simulink model "simulator_prototype_v2"  (R2021b)
(part 7 of 12)

t4573 = t3468.*t4113;
t4590 = t4080.*(t1896-t3232).*(-1.0e-8);
t4591 = (t4080.*(t1896-t3232))./1.0e+8;
t4603 = t4080.*(t1896-t3232).*(-6.2e-7);
t4604 = t4080.*(t1896-t3232).*6.2e-7;
t4610 = t4149.*(t1896-t3232).*(-7.26735e-3);
t4611 = t4149.*(t1896-t3232).*7.26735e-3;
t4648 = t528+t983+t1015+t1068+t1494+t1529+t2523+t2789+t2809+t3020+t3021;
t4649 = t2292+t3283+t3583+t3590;
t4653 = t1018+t1020+t1049+t1505+t2760+t2789+t2809+t2822+t3020+t3021;
t4654 = t562+t996+t1046+t1093+t1516+t1543+t2636+t2902+t2921+t3040+t3041;
t4662 = t1050+t1051+t1067+t1527+t2852+t2902+t2921+t2936+t3040+t3041;
t4675 = -t4302.*(t1861-t3214);
t4678 = t4302.*(t1861-t3214);
t4716 = t2757+t3403+t3704+t3707;
t4764 = t4323.*(t1896-t3232).*(-7.26735e-3);
t4777 = t3887+t4095;
t4780 = t3889+t4102;
t4785 = -t4365.*(t1861-t3214);
t4787 = t4365.*(t1861-t3214);
t4790 = t4080.*(t2694-t2701+t3036-t3043).*(-1.0e-8);
t4811 = t4783.*1.838876e-2;
t4813 = t4784.*9.99471e-3;
t4814 = t3909+t4126;
t4827 = t3915+t4137;
t4830 = t4080.*(t2694-t2701+t3036-t3043).*(-3.24e-6);
t4831 = t4080.*(t2694-t2701+t3036-t3043).*(-7.83e-6);
t4832 = t4080.*(t2694-t2701+t3036-t3043).*(-6.2e-7);
t4840 = t28.*t4817;
t4841 = t34.*t4817;
t4872 = t4399.*(t1896-t3232).*(-7.26735e-3);
t4873 = t4399.*(t1896-t3232).*7.26735e-3;
t4977 = t4211+t4218;
t4994 = t3209.*t4707;
t4995 = t3210.*t4707;
t5013 = t3229.*t4776.*7.26735e-3;
t5014 = t3230.*t4776.*7.26735e-3;
t5030 = -t5029;
t5058 = t3481.*t4758;
t5144 = t3524.*t4795.*7.26735e-3;
t5145 = t4795.*(t1896-t3232).*(-7.26735e-3);
t5159 = t3481.*t4865.*9.840000000000001e-6;
t5189 = t3789.*t4817;
t5197 = t50.*t189.*t5191.*9.543032792050485e-17;
t5199 = t3882.*t4707;
t5200 = -t4707.*(-t1901+t3122+t3270);
t5202 = t4707.*(-t1901+t3122+t3270);
t5207 = -t3863.*(t4127+t33.*(t1959-t3306+t38.*t1022.*(t855-t878).*2.196325630278387e-1));
t5225 = t3904.*t4776.*7.26735e-3;
t5226 = t4776.*(t1959-t3306+t38.*t1022.*(t855-t878).*2.196325630278387e-1).*(-7.26735e-3);
t5236 = -t5231;
t5244 = -t5241;
t5255 = t4080.*t4758;
t5265 = t4099+t4784;
t5266 = t4104+t4783;
t5301 = t4113.*t4795.*7.26735e-3;
t5302 = t4795.*(t1005+t26.*(t1941-t3308+t39.*t1022.*(t855-t878).*2.196325630278387e-1)).*(-7.26735e-3);
t5361 = t4312.*t4822;
et67 = -t2306-t2317+t3144+t3147+t35.*t941.*t948.*(t850-t874).*3.775747223193135e-1;
et68 = t36.*t941.*t948.*(t850-t874).*2.244797987218524e-1;
t5362 = (et67+et68).*(-t3519+t3521+t50.*t188.*t202.*(t46-t47).*2.711709361697228e-39);
t5433 = t3732.*t3877.*t3901.*t4134.*1.08769e-2;
t5434 = t3732.*t4134.*(t2674-t2676+t3022-t3027).*(t2694-t2701+t3036-t3043).*1.08769e-2;
t5440 = t3689.*t3877.*t3901.*t4175.*1.08769e-2;
t5441 = t3689.*t4175.*(t2674-t2676+t3022-t3027).*(t2694-t2701+t3036-t3043).*1.08769e-2;
t5480 = t3784.*t3877.*t3901.*t4134.*1.08769e-2;
t5481 = t3784.*t4134.*(t2674-t2676+t3022-t3027).*(t2694-t2701+t3036-t3043).*1.08769e-2;
t5483 = t3782.*t3877.*t3901.*t4175.*1.08769e-2;
t5484 = t3782.*t4175.*(t2674-t2676+t3022-t3027).*(t2694-t2701+t3036-t3043).*1.08769e-2;
t5489 = t3733+t4448+t4467;
t5668 = t3877.*t3901.*t3918.*(t1488+t1874+t2519+t2740+t2747+t3096+t3097).*(-7.26735e-3);
t5669 = t3918.*(t2674-t2676+t3022-t3027).*(t2694-t2701+t3036-t3043).*(t1488+t1874+t2519+t2740+t2747+t3096+t3097).*(-7.26735e-3);
t5670 = t3877.*t3901.*t3918.*(t1488+t1874+t2519+t2740+t2747+t3096+t3097).*7.26735e-3;
t5671 = t3918.*(t2674-t2676+t3022-t3027).*(t2694-t2701+t3036-t3043).*(t1488+t1874+t2519+t2740+t2747+t3096+t3097).*7.26735e-3;
t5672 = t3877.*t3892.*t3901.*(t1513+t1879+t2598+t2820+t2834+t3117+t3118).*(-7.26735e-3);
t5673 = t3892.*(t2674-t2676+t3022-t3027).*(t2694-t2701+t3036-t3043).*(t1513+t1879+t2598+t2820+t2834+t3117+t3118).*(-7.26735e-3);
t5674 = t3877.*t3892.*t3901.*(t1513+t1879+t2598+t2820+t2834+t3117+t3118).*7.26735e-3;
t5675 = t3892.*(t2674-t2676+t3022-t3027).*(t2694-t2701+t3036-t3043).*(t1513+t1879+t2598+t2820+t2834+t3117+t3118).*7.26735e-3;
t5678 = t3877.*t3901.*t3984.*(t1488+t1874+t2519+t2740+t2747+t3096+t3097).*(-7.26735e-3);
t5679 = t3984.*(t2674-t2676+t3022-t3027).*(t2694-t2701+t3036-t3043).*(t1488+t1874+t2519+t2740+t2747+t3096+t3097).*(-7.26735e-3);
tau_c = ft_9({t1005,t1022,t1089,t1104,t1105,t1108,t1115,t1121,t1158,t1159,t1190,t1193,t1194,t1196,t1205,t1207,t1208,t1210,t1212,t1214,t1217,t1218,t1219,t1220,t1221,t1222,t123,t1230,t1235,t1236,t1237,t1238,t1288,t1289,t1302,t1303,t1319,t1320,t1336,t1348,t1350,t1351,t1360,t1369,t1378,t1396,t14,t140,t1425,t1435,t1456,t1477,t1488,t15,t1513,t1539,t1544,t1545,t1547,t1548,t1549,t1553,t1554,t1559,t1564,t1565,t1576,t1577,t1578,t1579,t1581,t1584,t1585,t1586,t1587,t1591,t1595,t1596,t1598,t1599,t16,t1600,t1601,t1602,t1604,t1605,t1606,t1607,t1608,t1609,t1612,t1613,t1614,t1615,t1616,t1626,t1627,t1628,t1629,t1631,t1637,t1640,t1641,t1648,t1649,t1659,t1660,t1661,t1666,t1667,t1683,t1686,t1690,t1692,t17,t1700,t1701,t1703,t1704,t1705,t1712,t1717,t1738,t1741,t1742,t1750,t1752,t1753,t1754,t1758,t1759,t1775,t1776,t18,t1861,t1874,t1879,t188,t1881,t189,t1896,t19,t1901,t1941,t1953,t1959,t1973,t1993,t1994,t2,t20,t201,t202,t2023,t2053,t2060,t2089,t2090,t2098,t2099,t21,t2117,t2120,t2122,t2123,t2125,t2130,t2137,t2138,t2139,t2140,t2141,t2142,t2145,t2146,t2147,t2149,t2150,t2151,t2152,t2153,t2154,t2155,t2156,t2157,t2159,t2160,t2162,t2164,t2165,t2166,t2167,t2168,t2169,t2174,t2183,t2187,t2193,t2194,t2195,t2199,t22,t2203,t2215,t2219,t2222,t2223,t2239,t2240,t2256,t2257,t2291,t2292,t2293,t2294,t2295,t2296,t2297,t2298,t2299,t23,t2300,t2301,t2302,t2303,t2304,t2306,t2307,t2308,t2309,t2310,t2311,t2313,t2317,t2320,t2322,t2323,t2324,t2325,t2326,t2327,t2328,t2329,t2337,t2338,t2339,t2341,t2342,t2343,t2344,t2352,t2353,t2354,t2355,t2357,t2358,t2359,t236,t2360,t2361,t2362,t2363,t2364,t2365,t2366,t2367,t2368,t2369,t237,t2370,t2371,t2374,t2375,t2378,t2379,t238,t2380,t2384,t2388,t2389,t2391,t2394,t2395,t2397,t2398,t2399,t24,t2400,t2401,t2402,t2403,t2404,t2405,t241,t2413,t2414,t2419,t2421,t2422,t2423,t2433,t2434,t2438,t244,t2447,t2448,t2449,t2450,t2459,t2460,t2461,t2471,t2472,t2492,t2493,t2494,t25,t2502,t2508,t2509,t2510,t2515,t2519,t2520,t2525,t2527,t2529,t2530,t2532,t2534,t2539,t2555,t2556,t2572,t2575,t2583,t2598,t26,t2605,t2606,t2612,t2613,t2615,t2618,t2619,t262,t2638,t264,t2651,t2652,t2664,t2670,t2671,t2673,t2674,t2675,t2676,t2678,t2680,t2681,t2682,t2683,t2684,t2685,t2686,t2687,t2689,t2690,t2692,t2693,t2694,t2695,t2696,t2697,t2698,t27,t2700,t2701,t2704,t2705,t2707,t2708,t2709,t2711,t2712,t2713,t2715,t2716,t2717,t2719,t2720,t2721,t2733,t2735,t2736,t2740,t2742,t2744,t2745,t2747,t2748,t2749,t2750,t2753,t2754,t2759,t2765,t2769,t2773,t2774,t2775,t2777,t2778,t2779,t2781,t2785,t2786,t2787,t2788,t2790,t2792,t2795,t2797,t2798,t2799,t28,t2801,t2802,t2803,t2804,t2805,t2807,t2808,t2813,t2814,t2820,t2823,t2828,t2831,t2834,t2835,t2838,t2850,t2851,t2927,t2937,t2941,t2942,t2945,t2946,t2947,t2948,t2950,t2951,t2953,t2954,t2955,t2956,t2957,t2962,t2963,t2964,t2965,t2966,t2969,t2970,t2971,t2972,t2973,t2975,t2976,t2977,t2978,t2979,t2982,t2984,t2985,t2986,t2987,t2990,t2991,t2993,t2994,t2998,t3,t30,t3003,t3004,t3006,t3008,t3009,t3010,t3015,t3016,t3017,t3018,t3019,t3022,t3027,t3029,t3030,t3031,t3036,t3043,t3044,t3045,t3047,t3049,t3050,t3051,t3054,t3055,t3056,t3057,t3063,t3064,t3065,t3066,t3067,t3068,t3069,t3072,t3073,t3074,t3075,t3076,t3077,t3078,t3079,t3080,t3081,t3082,t3083,t3085,t3086,t3087,t3088,t3096,t3097,t31,t3109,t3117,t3118,t3119,t3121,t3122,t3128,t3129,t313,t3130,t3131,t3132,t3133,t3134,t3135,t3139,t314,t3140,t3141,t3142,t3144,t3147,t3149,t3150,t3152,t3153,t3154,t3155,t3156,t3157,t3158,t3159,t3160,t3161,t3162,t3163,t3164,t3165,t3166,t3170,t3171,t3172,t3178,t3179,t3180,t3184,t3186,t3187,t3188,t3189,t3190,t3191,t3193,t3194,t3196,t3197,t3198,t3199,t32,t3200,t3201,t3204,t3205,t3206,t3209,t321,t3210,t3212,t3214,t3215,t3217,t3218,t322,t3220,t3222,t3223,t3224,t3225,t3226,t3227,t3228,t3229,t3230,t3231,t3232,t3233,t3235,t3238,t3240,t3241,t3242,t3244,t3245,t3246,t3247,t3248,t3249,t3250,t3252,t3253,t3254,t3256,t3258,t3259,t326,t3260,t3261,t3262,t3263,t3264,t3265,t3266,t3269,t3270,t3271,t3272,t3275,t3276,t3277,t3278,t328,t3280,t3281,t3282,t3283,t3284,t3285,t3287,t3288,t3289,t329,t3290,t3291,t3293,t3294,t3296,t3297,t33,t330,t3300,t3301,t3302,t3303,t3304,t3305,t3306,t3308,t331,t3313,t3316,t3318,t3319,t332,t3321,t3322,t3323,t3324,t3325,t3326,t3327,t3328,t3329,t333,t3330,t3331,t3332,t3333,t3334,t3335,t3336,t3338,t3339,t3341,t3342,t3343,t3344,t3346,t3347,t3348,t3349,t335,t3350,t3351,t3352,t3353,t3354,t3355,t3356,t3359,t3360,t3367,t3369,t3370,t3373,t3376,t3377,t3379,t338,t3382,t3383,t3384,t3385,t3386,t3387,t3388,t3389,t339,t3392,t3394,t3395,t3396,t3397,t3398,t3399,t34,t3400,t3401,t3407,t3408,t3409,t341,t3410,t3411,t3412,t3415,t3417,t3419,t3420,t3421,t3422,t3423,t3424,t3427,t3428,t3429,t343,t3430,t3432,t3433,t3434,t3435,t3436,t3437,t3438,t3440,t3441,t3442,t3443,t3444,t3445,t3446,t3447,t3449,t3450,t3451,t3452,t3453,t3455,t3456,t3457,t3458,t3459,t346,t3461,t3464,t3465,t3467,t3468,t3470,t3473,t3475,t3477,t3479,t3480,t3481,t3483,t3484,t3485,t3486,t3487,t3488,t3489,t3490,t3495,t3498,t35,t350,t3505,t351,t3511,t3519,t352,t3522,t3523,t3524,t3526,t3527,t3528,t3529,t3531,t3533,t3534,t3535,t3536,t3537,t3538,t354,t3541,t3547,t3552,t3558,t3559,t356,t3560,t3561,t3563,t3566,t3576,t3577,t3578,t3579,t358,t3581,t3584,t3588,t359,t3590,t3595,t3598,t36,t360,t3607,t3617,t362,t3622,t3623,t3624,t3625,t3627,t3628,t363,t3630,t3634,t364,t3645,t3647,t365,t3655,t3659,t366,t3662,t3665,t3667,t3669,t3670,t3672,t3673,t3674,t3676,t3677,t3678,t3679,t3680,t3681,t3682,t3683,t3684,t3685,t3686,t3687,t3688,t3689,t369,t3690,t3699,t370,t3700,t3703,t3705,t371,t3711,t372,t3725,t3732,t3734,t3735,t3736,t3737,t3738,t3739,t3740,t3741,t3743,t3745,t3746,t3748,t3749,t3751,t3753,t3755,t3756,t3757,t3758,t3759,t3760,t3762,t3763,t3764,t3765,t3766,t3767,t3768,t3769,t3770,t3771,t3772,t3774,t3775,t3776,t3778,t3779,t378,t3782,t3783,t3784,t3785,t3786,t3787,t3788,t3789,t3790,t3791,t3792,t3793,t3794,t3795,t3796,t3798,t3799,t38,t380,t3800,t3802,t3804,t3805,t3807,t3811,t3812,t3813,t3814,t3815,t3816,t3817,t3818,t3819,t382,t3821,t3822,t3823,t3826,t3827,t3828,t3832,t3833,t3834,t3836,t3842,t3843,t3844,t3845,t3847,t3849,t3850,t3852,t3853,t3854,t3855,t3856,t3858,t3859,t3862,t3863,t3864,t3865,t3866,t3867,t3869,t387,t3870,t3871,t3872,t3873,t3876,t3877,t3880,t3882,t3886,t3891,t3892,t3893,t3894,t3895,t3898,t39,t3900,t3901,t3904,t3908,t3910,t3913,t3916,t3917,t3918,t3919,t3920,t3921,t3925,t3926,t3927,t3928,t3929,t3932,t3933,t3934,t3935,t3936,t3937,t3938,t3939,t3940,t3941,t3943,t3945,t3949,t3953,t3954,t3955,t3956,t3958,t3960,t3962,t3964,t3965,t3966,t3970,t3971,t3974,t3975,t3976,t3978,t3984,t3987,t3993,t3994,t3995,t3997,t3998,t4,t4000,t4001,t4002,t4003,t4004,t4005,t4009,t4012,t4019,t4020,t4023,t4028,t4029,t4030,t4033,t4045,t4046,t4048,t4049,t4054,t4058,t4060,t4063,t4080,t4087,t4088,t410,t4106,t4107,t4108,t4109,t4111,t4113,t4122,t4125,t4127,t4129,t4131,t4133,t4134,t4138,t4139,t4143,t4144,t4149,t4154,t4157,t4158,t4160,t4162,t4163,t4164,t4165,t4166,t4170,t4171,t4172,t4173,t4174,t4175,t4176,t4177,t4182,t4183,t4185,t4186,t4187,t4188,t4191,t4195,t4196,t4197,t4198,t42,t4204,t4205,t4206,t4207,t4212,t4214,t4215,t4219,t4220,t4221,t4225,t4228,t4230,t4231,t4233,t4234,t4235,t4236,t4241,t4242,t4244,t4249,t4250,t4251,t4253,t4254,t4257,t4259,t4262,t4263,t4272,t4273,t4277,t4279,t4280,t4281,t4283,t4285,t4286,t4288,t429,t4290,t4292,t4295,t4298,t4299,t43,t4300,t4302,t4304,t4308,t4310,t4317,t4318,t4321,t4322,t4323,t4324,t4327,t4328,t4329,t4330,t4333,t4334,t4336,t4337,t4338,t4339,t4340,t4342,t4344,t4346,t4347,t4348,t4349,t4350,t4351,t4352,t4355,t4356,t4360,t4362,t4363,t4364,t4365,t4366,t4367,t4368,t4371,t4399,t4401,t4404,t4405,t4407,t4408,t4412,t4413,t4415,t4416,t4417,t4418,t4419,t4420,t4421,t4425,t4426,t4427,t4428,t4429,t4430,t4431,t4432,t4434,t4435,t4436,t4437,t4439,t4441,t4444,t4446,t4447,t4449,t4450,t4451,t4453,t4454,t4455,t4456,t4458,t4460,t4462,t4463,t4468,t4471,t4473,t4474,t4476,t4479,t4480,t4483,t4484,t4489,t4496,t4500,t4573,t4574,t4579,t4587,t4589,t4591,t4594,t4599,t46,t4602,t4604,t4607,t4610,t4611,t4614,t4615,t4617,t4620,t4640,t4641,t4642,t4644,t4645,t4647,t4648,t4649,t4650,t4652,t4653,t4654,t4655,t4661,t4662,t4663,t4664,t4667,t4669,t4678,t4679,t4680,t4682,t4683,t4686,t4687,t4688,t4689,t4690,t4691,t4692,t4693,t4694,t4695,t4696,t4697,t4698,t4699,t47,t4700,t4701,t4702,t4703,t4704,t4705,t4716,t4742,t4758,t4764,t4772,t4777,t4779,t4780,t4785,t4787,t4789,t4790,t4791,t4792,t4795,t4811,t4813,t4814,t4816,t4817,t4820,t4821,t4822,t4823,t4826,t4829,t4830,t4831,t4832,t4837,t4838,t4839,t4840,t4841,t4842,t4860,t4865,t4868,t4869,t4870,t4871,t4872,t4873,t4898,t4911,t4931,t4963,t4964,t4965,t4966,t4974,t4976,t4977,t4985,t4986,t4994,t4995,t5,t50,t5001,t5002,t5005,t5007,t5010,t5013,t5014,t5017,t5021,t5023,t5026,t5030,t5035,t5036,t5037,t5038,t5039,t5040,t5041,t5042,t5043,t5044,t5045,t5046,t5047,t5048,t5049,t5050,t5058,t5061,t5144,t5145,t5153,t5159,t5167,t5168,t5169,t5189,t5191,t5197,t5199,t5202,t5207,t5219,t5221,t5223,t5224,t5225,t5226,t5227,t5229,t5230,t5231,t5233,t5235,t5236,t5239,t5240,t5241,t5243,t5244,t5245,t5246,t5247,t5248,t5252,t5254,t5255,t5257,t5265,t5266,t5301,t5302,t5306,t5308,t5316,t5317,t5320,t5328,t5337,t5338,t5339,t5340,t5342,t5344,t5345,t5346,t5347,t5348,t5349,t5350,t5361,t5362,t5377,t5379,t5380,t5381,t5383,t5384,t5388,t5389,t5399,t5402,t5403,t5405,t5407,t5411,t5427,t5428,t5433,t5434,t5440,t5441,t5443,t5444,t5480,t5481,t5482,t5483,t5484,t5485,t5486,t5487,t5488,t5489,t5490,t5491,t5492,t5493,t5494,t5496,t5498,t5500,t5510,t5517,t5518,t5524,t5531,t5552,t5578,t5580,t56,t5620,t5626,t5627,t5631,t5670,t5671,t5674,t5675,t5678,t5679,t5694,t5695,t5702,t5703,t5719,t5722,t5723,t58,t5835,t5839,t5840,t59,t5932,t5951,t5953,t5954,t6,t60,t6183,t6184,t6185,t6219,t6221,t6247,t6253,t628,t635,t636,t638,t640,t641,t642,t643,t645,t646,t6484,t6485,t6486,t649,t654,t6543,t6544,t655,t656,t657,t659,t660,t663,t664,t665,t6658,t666,t6663,t667,t668,t669,t67,t670,t672,t673,t674,t675,t676,t677,t678,t679,t68,t681,t6811,t6812,t6813,t682,t683,t684,t685,t686,t687,t689,t6892,t6893,t691,t692,t693,t694,t7,t70,t702,t7041,t707,t708,t71,t710,t715,t716,t717,t718,t721,t722,t724,t725,t73,t736,t738,t740,t741,t749,t756,t76,t762,t768,t777,t792,t793,t801,t802,t808,t813,t819,t821,t850,t855,t874,t878,t89,t90,t91,t92,t941,t944,t948,t951,t97});
end
function tau_c = ft_9(ct)
t1005 = ct{1};
t1022 = ct{2};
t1089 = ct{3};
t1104 = ct{4};
t1105 = ct{5};
t1108 = ct{6};
t1115 = ct{7};
t1121 = ct{8};
t1158 = ct{9};
t1159 = ct{10};
t1190 = ct{11};
t1193 = ct{12};
t1194 = ct{13};
t1196 = ct{14};
t1205 = ct{15};
t1207 = ct{16};
t1208 = ct{17};
t1210 = ct{18};
t1212 = ct{19};
t1214 = ct{20};
t1217 = ct{21};
t1218 = ct{22};
t1219 = ct{23};
t1220 = ct{24};
t1221 = ct{25};
t1222 = ct{26};
t123 = ct{27};
t1230 = ct{28};
t1235 = ct{29};
t1236 = ct{30};
t1237 = ct{31};
t1238 = ct{32};
t1288 = ct{33};
t1289 = ct{34};
t1302 = ct{35};
t1303 = ct{36};
t1319 = ct{37};
t1320 = ct{38};
t1336 = ct{39};
t1348 = ct{40};
t1350 = ct{41};
t1351 = ct{42};
t1360 = ct{43};
t1369 = ct{44};
t1378 = ct{45};
t1396 = ct{46};
t14 = ct{47};
t140 = ct{48};
t1425 = ct{49};
t1435 = ct{50};
t1456 = ct{51};
t1477 = ct{52};
t1488 = ct{53};
t15 = ct{54};
t1513 = ct{55};
t1539 = ct{56};
t1544 = ct{57};
t1545 = ct{58};
t1547 = ct{59};
t1548 = ct{60};
t1549 = ct{61};
t1553 = ct{62};
t1554 = ct{63};
t1559 = ct{64};
t1564 = ct{65};
t1565 = ct{66};
t1576 = ct{67};
t1577 = ct{68};
t1578 = ct{69};
t1579 = ct{70};
t1581 = ct{71};
t1584 = ct{72};
t1585 = ct{73};
t1586 = ct{74};
t1587 = ct{75};
t1591 = ct{76};
t1595 = ct{77};
t1596 = ct{78};
t1598 = ct{79};
t1599 = ct{80};
t16 = ct{81};
t1600 = ct{82};
t1601 = ct{83};
t1602 = ct{84};
t1604 = ct{85};
t1605 = ct{86};
t1606 = ct{87};
t1607 = ct{88};
t1608 = ct{89};
t1609 = ct{90};
t1612 = ct{91};
t1613 = ct{92};
t1614 = ct{93};
t1615 = ct{94};
t1616 = ct{95};
t1626 = ct{96};
t1627 = ct{97};
t1628 = ct{98};
t1629 = ct{99};
t1631 = ct{100};
t1637 = ct{101};
t1640 = ct{102};
t1641 = ct{103};
t1648 = ct{104};
t1649 = ct{105};
t1659 = ct{106};
t1660 = ct{107};
t1661 = ct{108};
t1666 = ct{109};
t1667 = ct{110};
t1683 = ct{111};
t1686 = ct{112};
t1690 = ct{113};
t1692 = ct{114};
t17 = ct{115};
t1700 = ct{116};
t1701 = ct{117};
t1703 = ct{118};
t1704 = ct{119};
t1705 = ct{120};
t1712 = ct{121};
t1717 = ct{122};
t1738 = ct{123};
t1741 = ct{124};
t1742 = ct{125};
t1750 = ct{126};
t1752 = ct{127};
t1753 = ct{128};
t1754 = ct{129};
t1758 = ct{130};
t1759 = ct{131};
t1775 = ct{132};
t1776 = ct{133};
t18 = ct{134};
t1861 = ct{135};
t1874 = ct{136};
t1879 = ct{137};
t188 = ct{138};
t1881 = ct{139};
t189 = ct{140};
t1896 = ct{141};
t19 = ct{142};
t1901 = ct{143};
t1941 = ct{144};
t1953 = ct{145};
t1959 = ct{146};
t1973 = ct{147};
t1993 = ct{148};
t1994 = ct{149};
t2 = ct{150};
t20 = ct{151};
t201 = ct{152};
t202 = ct{153};
t2023 = ct{154};
t2053 = ct{155};
t2060 = ct{156};
t2089 = ct{157};
t2090 = ct{158};
t2098 = ct{159};
t2099 = ct{160};
t21 = ct{161};
t2117 = ct{162};
t2120 = ct{163};
t2122 = ct{164};
t2123 = ct{165};
t2125 = ct{166};
t2130 = ct{167};
t2137 = ct{168};
t2138 = ct{169};
t2139 = ct{170};
t2140 = ct{171};
t2141 = ct{172};
t2142 = ct{173};
t2145 = ct{174};
t2146 = ct{175};
t2147 = ct{176};
t2149 = ct{177};
t2150 = ct{178};
t2151 = ct{179};
t2152 = ct{180};
t2153 = ct{181};
t2154 = ct{182};
t2155 = ct{183};
t2156 = ct{184};
t2157 = ct{185};
t2159 = ct{186};
t2160 = ct{187};
t2162 = ct{188};
t2164 = ct{189};
t2165 = ct{190};
t2166 = ct{191};
t2167 = ct{192};
t2168 = ct{193};
t2169 = ct{194};
t2174 = ct{195};
t2183 = ct{196};
t2187 = ct{197};
t2193 = ct{198};
t2194 = ct{199};
t2195 = ct{200};
t2199 = ct{201};
t22 = ct{202};
t2203 = ct{203};
t2215 = ct{204};
t2219 = ct{205};
t2222 = ct{206};
t2223 = ct{207};
t2239 = ct{208};
t2240 = ct{209};
t2256 = ct{210};
t2257 = ct{211};
t2291 = ct{212};
t2292 = ct{213};
t2293 = ct{214};
t2294 = ct{215};
t2295 = ct{216};
t2296 = ct{217};
t2297 = ct{218};
t2298 = ct{219};
t2299 = ct{220};
t23 = ct{221};
t2300 = ct{222};
t2301 = ct{223};
t2302 = ct{224};
t2303 = ct{225};
t2304 = ct{226};
t2306 = ct{227};
t2307 = ct{228};
t2308 = ct{229};
t2309 = ct{230};
t2310 = ct{231};
t2311 = ct{232};
t2313 = ct{233};
t2317 = ct{234};
t2320 = ct{235};
t2322 = ct{236};
t2323 = ct{237};
t2324 = ct{238};
t2325 = ct{239};
t2326 = ct{240};
t2327 = ct{241};
t2328 = ct{242};
t2329 = ct{243};
t2337 = ct{244};
t2338 = ct{245};
t2339 = ct{246};
t2341 = ct{247};
t2342 = ct{248};
t2343 = ct{249};
t2344 = ct{250};
t2352 = ct{251};
t2353 = ct{252};
t2354 = ct{253};
t2355 = ct{254};
t2357 = ct{255};
t2358 = ct{256};
t2359 = ct{257};
t236 = ct{258};
t2360 = ct{259};
t2361 = ct{260};
t2362 = ct{261};
t2363 = ct{262};
t2364 = ct{263};
t2365 = ct{264};
t2366 = ct{265};
t2367 = ct{266};
t2368 = ct{267};
t2369 = ct{268};
t237 = ct{269};
t2370 = ct{270};
t2371 = ct{271};
t2374 = ct{272};
t2375 = ct{273};
t2378 = ct{274};
t2379 = ct{275};
t238 = ct{276};
t2380 = ct{277};
t2384 = ct{278};
t2388 = ct{279};
t2389 = ct{280};
t2391 = ct{281};
t2394 = ct{282};
t2395 = ct{283};
t2397 = ct{284};
t2398 = ct{285};
t2399 = ct{286};
t24 = ct{287};
t2400 = ct{288};
t2401 = ct{289};
t2402 = ct{290};
t2403 = ct{291};
t2404 = ct{292};
t2405 = ct{293};
t241 = ct{294};
t2413 = ct{295};
t2414 = ct{296};
t2419 = ct{297};
t2421 = ct{298};
t2422 = ct{299};
t2423 = ct{300};
t2433 = ct{301};
t2434 = ct{302};
t2438 = ct{303};
t244 = ct{304};
t2447 = ct{305};
t2448 = ct{306};
t2449 = ct{307};
t2450 = ct{308};
t2459 = ct{309};
t2460 = ct{310};
t2461 = ct{311};
t2471 = ct{312};
t2472 = ct{313};
t2492 = ct{314};
t2493 = ct{315};
t2494 = ct{316};
t25 = ct{317};
t2502 = ct{318};
t2508 = ct{319};
t2509 = ct{320};
t2510 = ct{321};
t2515 = ct{322};
t2519 = ct{323};
t2520 = ct{324};
t2525 = ct{325};
t2527 = ct{326};
t2529 = ct{327};
t2530 = ct{328};
t2532 = ct{329};
t2534 = ct{330};
t2539 = ct{331};
t2555 = ct{332};
t2556 = ct{333};
t2572 = ct{334};
t2575 = ct{335};
t2583 = ct{336};
t2598 = ct{337};
t26 = ct{338};
t2605 = ct{339};
t2606 = ct{340};
t2612 = ct{341};
t2613 = ct{342};
t2615 = ct{343};
t2618 = ct{344};
t2619 = ct{345};
t262 = ct{346};
t2638 = ct{347};
t264 = ct{348};
t2651 = ct{349};
t2652 = ct{350};
t2664 = ct{351};
t2670 = ct{352};
t2671 = ct{353};
t2673 = ct{354};
t2674 = ct{355};
t2675 = ct{356};
t2676 = ct{357};
t2678 = ct{358};
t2680 = ct{359};
t2681 = ct{360};
t2682 = ct{361};
t2683 = ct{362};
t2684 = ct{363};
t2685 = ct{364};
t2686 = ct{365};
t2687 = ct{366};
t2689 = ct{367};
t2690 = ct{368};
t2692 = ct{369};
t2693 = ct{370};
t2694 = ct{371};
t2695 = ct{372};
t2696 = ct{373};
t2697 = ct{374};
t2698 = ct{375};
t27 = ct{376};
t2700 = ct{377};
t2701 = ct{378};
t2704 = ct{379};
t2705 = ct{380};
t2707 = ct{381};
t2708 = ct{382};
t2709 = ct{383};
t2711 = ct{384};
t2712 = ct{385};
t2713 = ct{386};
t2715 = ct{387};
t2716 = ct{388};
t2717 = ct{389};
t2719 = ct{390};
t2720 = ct{391};
t2721 = ct{392};
t2733 = ct{393};
t2735 = ct{394};
t2736 = ct{395};
t2740 = ct{396};
t2742 = ct{397};
t2744 = ct{398};
t2745 = ct{399};
t2747 = ct{400};
t2748 = ct{401};
t2749 = ct{402};
t2750 = ct{403};
t2753 = ct{404};
t2754 = ct{405};
t2759 = ct{406};
t2765 = ct{407};
t2769 = ct{408};
t2773 = ct{409};
t2774 = ct{410};
t2775 = ct{411};
t2777 = ct{412};
t2778 = ct{413};
t2779 = ct{414};
t2781 = ct{415};
t2785 = ct{416};
t2786 = ct{417};
t2787 = ct{418};
t2788 = ct{419};
t2790 = ct{420};
t2792 = ct{421};
t2795 = ct{422};
t2797 = ct{423};
t2798 = ct{424};
t2799 = ct{425};
t28 = ct{426};
t2801 = ct{427};
t2802 = ct{428};
t2803 = ct{429};
t2804 = ct{430};
t2805 = ct{431};
t2807 = ct{432};
t2808 = ct{433};
t2813 = ct{434};
t2814 = ct{435};
t2820 = ct{436};
t2823 = ct{437};
t2828 = ct{438};
t2831 = ct{439};
t2834 = ct{440};
t2835 = ct{441};
t2838 = ct{442};
t2850 = ct{443};
t2851 = ct{444};
t2927 = ct{445};
t2937 = ct{446};
t2941 = ct{447};
t2942 = ct{448};
t2945 = ct{449};
t2946 = ct{450};
t2947 = ct{451};
t2948 = ct{452};
t2950 = ct{453};
t2951 = ct{454};
t2953 = ct{455};
t2954 = ct{456};
t2955 = ct{457};
t2956 = ct{458};
t2957 = ct{459};
t2962 = ct{460};
t2963 = ct{461};
t2964 = ct{462};
t2965 = ct{463};
t2966 = ct{464};
t2969 = ct{465};
t2970 = ct{466};
t2971 = ct{467};
t2972 = ct{468};
t2973 = ct{469};
t2975 = ct{470};
t2976 = ct{471};
t2977 = ct{472};
t2978 = ct{473};
t2979 = ct{474};
t2982 = ct{475};
t2984 = ct{476};
t2985 = ct{477};
t2986 = ct{478};
t2987 = ct{479};
t2990 = ct{480};
t2991 = ct{481};
t2993 = ct{482};
t2994 = ct{483};
t2998 = ct{484};
t3 = ct{485};
t30 = ct{486};
t3003 = ct{487};
t3004 = ct{488};
t3006 = ct{489};
t3008 = ct{490};
t3009 = ct{491};
t3010 = ct{492};
t3015 = ct{493};
t3016 = ct{494};
t3017 = ct{495};
t3018 = ct{496};
t3019 = ct{497};
t3022 = ct{498};
t3027 = ct{499};
t3029 = ct{500};
t3030 = ct{501};
t3031 = ct{502};
t3036 = ct{503};
t3043 = ct{504};
t3044 = ct{505};
t3045 = ct{506};
t3047 = ct{507};
t3049 = ct{508};
t3050 = ct{509};
t3051 = ct{510};
t3054 = ct{511};
t3055 = ct{512};
t3056 = ct{513};
t3057 = ct{514};
t3063 = ct{515};
t3064 = ct{516};
t3065 = ct{517};
t3066 = ct{518};
t3067 = ct{519};
t3068 = ct{520};
t3069 = ct{521};
t3072 = ct{522};
t3073 = ct{523};
t3074 = ct{524};
t3075 = ct{525};
t3076 = ct{526};
t3077 = ct{527};
t3078 = ct{528};
t3079 = ct{529};
t3080 = ct{530};
t3081 = ct{531};
t3082 = ct{532};
t3083 = ct{533};
t3085 = ct{534};
t3086 = ct{535};
t3087 = ct{536};
t3088 = ct{537};
t3096 = ct{538};
t3097 = ct{539};
t31 = ct{540};
t3109 = ct{541};
t3117 = ct{542};
t3118 = ct{543};
t3119 = ct{544};
t3121 = ct{545};
t3122 = ct{546};
t3128 = ct{547};
t3129 = ct{548};
t313 = ct{549};
t3130 = ct{550};
t3131 = ct{551};
t3132 = ct{552};
t3133 = ct{553};
t3134 = ct{554};
t3135 = ct{555};
t3139 = ct{556};
t314 = ct{557};
t3140 = ct{558};
t3141 = ct{559};
t3142 = ct{560};
t3144 = ct{561};
t3147 = ct{562};
t3149 = ct{563};
t3150 = ct{564};
t3152 = ct{565};
t3153 = ct{566};
t3154 = ct{567};
t3155 = ct{568};
t3156 = ct{569};
t3157 = ct{570};
t3158 = ct{571};
t3159 = ct{572};
t3160 = ct{573};
t3161 = ct{574};
t3162 = ct{575};
t3163 = ct{576};
t3164 = ct{577};
t3165 = ct{578};
t3166 = ct{579};
t3170 = ct{580};
t3171 = ct{581};
t3172 = ct{582};
t3178 = ct{583};
t3179 = ct{584};
t3180 = ct{585};
t3184 = ct{586};
t3186 = ct{587};
t3187 = ct{588};
t3188 = ct{589};
t3189 = ct{590};
t3190 = ct{591};
t3191 = ct{592};
t3193 = ct{593};
t3194 = ct{594};
t3196 = ct{595};
t3197 = ct{596};
t3198 = ct{597};
t3199 = ct{598};
t32 = ct{599};
t3200 = ct{600};
t3201 = ct{601};
t3204 = ct{602};
t3205 = ct{603};
t3206 = ct{604};
t3209 = ct{605};
t321 = ct{606};
t3210 = ct{607};
t3212 = ct{608};
t3214 = ct{609};
t3215 = ct{610};
t3217 = ct{611};
t3218 = ct{612};
t322 = ct{613};
t3220 = ct{614};
t3222 = ct{615};
t3223 = ct{616};
t3224 = ct{617};
t3225 = ct{618};
t3226 = ct{619};
t3227 = ct{620};
t3228 = ct{621};
t3229 = ct{622};
t3230 = ct{623};
t3231 = ct{624};
t3232 = ct{625};
t3233 = ct{626};
t3235 = ct{627};
t3238 = ct{628};
t3240 = ct{629};
t3241 = ct{630};
t3242 = ct{631};
t3244 = ct{632};
t3245 = ct{633};
t3246 = ct{634};
t3247 = ct{635};
t3248 = ct{636};
t3249 = ct{637};
t3250 = ct{638};
t3252 = ct{639};
t3253 = ct{640};
t3254 = ct{641};
t3256 = ct{642};
t3258 = ct{643};
t3259 = ct{644};
t326 = ct{645};
t3260 = ct{646};
t3261 = ct{647};
t3262 = ct{648};
t3263 = ct{649};
t3264 = ct{650};
t3265 = ct{651};
t3266 = ct{652};
t3269 = ct{653};
t3270 = ct{654};
t3271 = ct{655};
t3272 = ct{656};
t3275 = ct{657};
t3276 = ct{658};
t3277 = ct{659};
t3278 = ct{660};
t328 = ct{661};
t3280 = ct{662};
t3281 = ct{663};
t3282 = ct{664};
t3283 = ct{665};
t3284 = ct{666};
t3285 = ct{667};
t3287 = ct{668};
t3288 = ct{669};
t3289 = ct{670};
t329 = ct{671};
t3290 = ct{672};
t3291 = ct{673};
t3293 = ct{674};
t3294 = ct{675};
t3296 = ct{676};
t3297 = ct{677};
t33 = ct{678};
t330 = ct{679};
t3300 = ct{680};
t3301 = ct{681};
t3302 = ct{682};
t3303 = ct{683};
t3304 = ct{684};
t3305 = ct{685};
t3306 = ct{686};
t3308 = ct{687};
t331 = ct{688};
t3313 = ct{689};
t3316 = ct{690};
t3318 = ct{691};
t3319 = ct{692};
t332 = ct{693};
t3321 = ct{694};
t3322 = ct{695};
t3323 = ct{696};
t3324 = ct{697};
t3325 = ct{698};
t3326 = ct{699};
t3327 = ct{700};
t3328 = ct{701};
t3329 = ct{702};
t333 = ct{703};
t3330 = ct{704};
t3331 = ct{705};
t3332 = ct{706};
t3333 = ct{707};
t3334 = ct{708};
t3335 = ct{709};
t3336 = ct{710};
t3338 = ct{711};
t3339 = ct{712};
t3341 = ct{713};
t3342 = ct{714};
t3343 = ct{715};
t3344 = ct{716};
t3346 = ct{717};
t3347 = ct{718};
t3348 = ct{719};
t3349 = ct{720};
t335 = ct{721};
t3350 = ct{722};
t3351 = ct{723};
t3352 = ct{724};
t3353 = ct{725};
t3354 = ct{726};
t3355 = ct{727};
t3356 = ct{728};
t3359 = ct{729};
t3360 = ct{730};
t3367 = ct{731};
t3369 = ct{732};
t3370 = ct{733};
t3373 = ct{734};
t3376 = ct{735};
t3377 = ct{736};
t3379 = ct{737};
t338 = ct{738};
t3382 = ct{739};
t3383 = ct{740};
t3384 = ct{741};
t3385 = ct{742};
t3386 = ct{743};
t3387 = ct{744};
t3388 = ct{745};
t3389 = ct{746};
t339 = ct{747};
t3392 = ct{748};
t3394 = ct{749};
t3395 = ct{750};
t3396 = ct{751};
t3397 = ct{752};
t3398 = ct{753};
t3399 = ct{754};
t34 = ct{755};
t3400 = ct{756};
t3401 = ct{757};
t3407 = ct{758};
t3408 = ct{759};
t3409 = ct{760};
t341 = ct{761};
t3410 = ct{762};
t3411 = ct{763};
t3412 = ct{764};
t3415 = ct{765};
t3417 = ct{766};
t3419 = ct{767};
t3420 = ct{768};
t3421 = ct{769};
t3422 = ct{770};
t3423 = ct{771};
t3424 = ct{772};
t3427 = ct{773};
t3428 = ct{774};
t3429 = ct{775};
t343 = ct{776};
t3430 = ct{777};
t3432 = ct{778};
t3433 = ct{779};
t3434 = ct{780};
t3435 = ct{781};
t3436 = ct{782};
t3437 = ct{783};
t3438 = ct{784};
t3440 = ct{785};
t3441 = ct{786};
t3442 = ct{787};
t3443 = ct{788};
t3444 = ct{789};
t3445 = ct{790};
t3446 = ct{791};
t3447 = ct{792};
t3449 = ct{793};
t3450 = ct{794};
t3451 = ct{795};
t3452 = ct{796};
t3453 = ct{797};
t3455 = ct{798};
t3456 = ct{799};
t3457 = ct{800};
t3458 = ct{801};
t3459 = ct{802};
t346 = ct{803};
t3461 = ct{804};
t3464 = ct{805};
t3465 = ct{806};
t3467 = ct{807};
t3468 = ct{808};
t3470 = ct{809};
t3473 = ct{810};
t3475 = ct{811};
t3477 = ct{812};
t3479 = ct{813};
t3480 = ct{814};
t3481 = ct{815};
t3483 = ct{816};
t3484 = ct{817};
t3485 = ct{818};
t3486 = ct{819};
t3487 = ct{820};
t3488 = ct{821};
t3489 = ct{822};
t3490 = ct{823};
t3495 = ct{824};
t3498 = ct{825};
t35 = ct{826};
t350 = ct{827};
t3505 = ct{828};
t351 = ct{829};
t3511 = ct{830};
t3519 = ct{831};
t352 = ct{832};
t3522 = ct{833};
t3523 = ct{834};
t3524 = ct{835};
t3526 = ct{836};
t3527 = ct{837};
t3528 = ct{838};
t3529 = ct{839};
t3531 = ct{840};
t3533 = ct{841};
t3534 = ct{842};
t3535 = ct{843};
t3536 = ct{844};
t3537 = ct{845};
t3538 = ct{846};
t354 = ct{847};
t3541 = ct{848};
t3547 = ct{849};
t3552 = ct{850};
t3558 = ct{851};
t3559 = ct{852};
t356 = ct{853};
t3560 = ct{854};
t3561 = ct{855};
t3563 = ct{856};
t3566 = ct{857};
t3576 = ct{858};
t3577 = ct{859};
t3578 = ct{860};
t3579 = ct{861};
t358 = ct{862};
t3581 = ct{863};
t3584 = ct{864};
t3588 = ct{865};
t359 = ct{866};
t3590 = ct{867};
t3595 = ct{868};
t3598 = ct{869};
t36 = ct{870};
t360 = ct{871};
t3607 = ct{872};
t3617 = ct{873};
t362 = ct{874};
t3622 = ct{875};
t3623 = ct{876};
t3624 = ct{877};
t3625 = ct{878};
t3627 = ct{879};
t3628 = ct{880};
t363 = ct{881};
t3630 = ct{882};
t3634 = ct{883};
t364 = ct{884};
t3645 = ct{885};
t3647 = ct{886};
t365 = ct{887};
t3655 = ct{888};
t3659 = ct{889};
t366 = ct{890};
t3662 = ct{891};
t3665 = ct{892};
t3667 = ct{893};
t3669 = ct{894};
t3670 = ct{895};
t3672 = ct{896};
t3673 = ct{897};
t3674 = ct{898};
t3676 = ct{899};
t3677 = ct{900};
t3678 = ct{901};
t3679 = ct{902};
t3680 = ct{903};
t3681 = ct{904};
t3682 = ct{905};
t3683 = ct{906};
t3684 = ct{907};
t3685 = ct{908};
t3686 = ct{909};
t3687 = ct{910};
t3688 = ct{911};
t3689 = ct{912};
t369 = ct{913};
t3690 = ct{914};
t3699 = ct{915};
t370 = ct{916};
t3700 = ct{917};
t3703 = ct{918};
t3705 = ct{919};
t371 = ct{920};
t3711 = ct{921};
t372 = ct{922};
t3725 = ct{923};
t3732 = ct{924};
t3734 = ct{925};
t3735 = ct{926};
t3736 = ct{927};
t3737 = ct{928};
t3738 = ct{929};
t3739 = ct{930};
t3740 = ct{931};
t3741 = ct{932};
t3743 = ct{933};
t3745 = ct{934};
t3746 = ct{935};
t3748 = ct{936};
t3749 = ct{937};
t3751 = ct{938};
t3753 = ct{939};
t3755 = ct{940};
t3756 = ct{941};
t3757 = ct{942};
t3758 = ct{943};
t3759 = ct{944};
t3760 = ct{945};
t3762 = ct{946};
t3763 = ct{947};
t3764 = ct{948};
t3765 = ct{949};
t3766 = ct{950};
t3767 = ct{951};
t3768 = ct{952};
t3769 = ct{953};
t3770 = ct{954};
t3771 = ct{955};
t3772 = ct{956};
t3774 = ct{957};
t3775 = ct{958};
t3776 = ct{959};
t3778 = ct{960};
t3779 = ct{961};
t378 = ct{962};
t3782 = ct{963};
t3783 = ct{964};
t3784 = ct{965};
t3785 = ct{966};
t3786 = ct{967};
t3787 = ct{968};
t3788 = ct{969};
t3789 = ct{970};
t3790 = ct{971};
t3791 = ct{972};
t3792 = ct{973};
t3793 = ct{974};
t3794 = ct{975};
t3795 = ct{976};
t3796 = ct{977};
t3798 = ct{978};
t3799 = ct{979};
t38 = ct{980};
t380 = ct{981};
t3800 = ct{982};
t3802 = ct{983};
t3804 = ct{984};
t3805 = ct{985};
t3807 = ct{986};
t3811 = ct{987};
t3812 = ct{988};
t3813 = ct{989};
t3814 = ct{990};
t3815 = ct{991};
t3816 = ct{992};
t3817 = ct{993};
t3818 = ct{994};
t3819 = ct{995};
t382 = ct{996};
t3821 = ct{997};
t3822 = ct{998};
t3823 = ct{999};
t3826 = ct{1000};
t3827 = ct{1001};
t3828 = ct{1002};
t3832 = ct{1003};
t3833 = ct{1004};
t3834 = ct{1005};
t3836 = ct{1006};
t3842 = ct{1007};
t3843 = ct{1008};
t3844 = ct{1009};
t3845 = ct{1010};
t3847 = ct{1011};
t3849 = ct{1012};
t3850 = ct{1013};
t3852 = ct{1014};
t3853 = ct{1015};
t3854 = ct{1016};
t3855 = ct{1017};
t3856 = ct{1018};
t3858 = ct{1019};
t3859 = ct{1020};
t3862 = ct{1021};
t3863 = ct{1022};
t3864 = ct{1023};
t3865 = ct{1024};
t3866 = ct{1025};
t3867 = ct{1026};
t3869 = ct{1027};
t387 = ct{1028};
t3870 = ct{1029};
t3871 = ct{1030};
t3872 = ct{1031};
t3873 = ct{1032};
t3876 = ct{1033};
t3877 = ct{1034};
t3880 = ct{1035};
t3882 = ct{1036};
t3886 = ct{1037};
t3891 = ct{1038};
t3892 = ct{1039};
t3893 = ct{1040};
t3894 = ct{1041};
t3895 = ct{1042};
t3898 = ct{1043};
t39 = ct{1044};
t3900 = ct{1045};
t3901 = ct{1046};
t3904 = ct{1047};
t3908 = ct{1048};
t3910 = ct{1049};
t3913 = ct{1050};
t3916 = ct{1051};
t3917 = ct{1052};
t3918 = ct{1053};
t3919 = ct{1054};
t3920 = ct{1055};
t3921 = ct{1056};
t3925 = ct{1057};
t3926 = ct{1058};
t3927 = ct{1059};
t3928 = ct{1060};
t3929 = ct{1061};
t3932 = ct{1062};
t3933 = ct{1063};
t3934 = ct{1064};
t3935 = ct{1065};
t3936 = ct{1066};
t3937 = ct{1067};
t3938 = ct{1068};
t3939 = ct{1069};
t3940 = ct{1070};
t3941 = ct{1071};
t3943 = ct{1072};
t3945 = ct{1073};
t3949 = ct{1074};
t3953 = ct{1075};
t3954 = ct{1076};
t3955 = ct{1077};
t3956 = ct{1078};
t3958 = ct{1079};
t3960 = ct{1080};
t3962 = ct{1081};
t3964 = ct{1082};
t3965 = ct{1083};
t3966 = ct{1084};
t3970 = ct{1085};
t3971 = ct{1086};
t3974 = ct{1087};
t3975 = ct{1088};
t3976 = ct{1089};
t3978 = ct{1090};
t3984 = ct{1091};
t3987 = ct{1092};
t3993 = ct{1093};
t3994 = ct{1094};
t3995 = ct{1095};
t3997 = ct{1096};
t3998 = ct{1097};
t4 = ct{1098};
t4000 = ct{1099};
t4001 = ct{1100};
t4002 = ct{1101};
t4003 = ct{1102};
t4004 = ct{1103};
t4005 = ct{1104};
t4009 = ct{1105};
t4012 = ct{1106};
t4019 = ct{1107};
t4020 = ct{1108};
t4023 = ct{1109};
t4028 = ct{1110};
t4029 = ct{1111};
t4030 = ct{1112};
t4033 = ct{1113};
t4045 = ct{1114};
t4046 = ct{1115};
t4048 = ct{1116};
t4049 = ct{1117};
t4054 = ct{1118};
t4058 = ct{1119};
t4060 = ct{1120};
t4063 = ct{1121};
t4080 = ct{1122};
t4087 = ct{1123};
t4088 = ct{1124};
t410 = ct{1125};
t4106 = ct{1126};
t4107 = ct{1127};
t4108 = ct{1128};
t4109 = ct{1129};
t4111 = ct{1130};
t4113 = ct{1131};
t4122 = ct{1132};
t4125 = ct{1133};
t4127 = ct{1134};
t4129 = ct{1135};
t4131 = ct{1136};
t4133 = ct{1137};
t4134 = ct{1138};
t4138 = ct{1139};
t4139 = ct{1140};
t4143 = ct{1141};
t4144 = ct{1142};
t4149 = ct{1143};
t4154 = ct{1144};
t4157 = ct{1145};
t4158 = ct{1146};
t4160 = ct{1147};
t4162 = ct{1148};
t4163 = ct{1149};
t4164 = ct{1150};
t4165 = ct{1151};
t4166 = ct{1152};
t4170 = ct{1153};
t4171 = ct{1154};
t4172 = ct{1155};
t4173 = ct{1156};
t4174 = ct{1157};
t4175 = ct{1158};
t4176 = ct{1159};
t4177 = ct{1160};
t4182 = ct{1161};
t4183 = ct{1162};
t4185 = ct{1163};
t4186 = ct{1164};
t4187 = ct{1165};
t4188 = ct{1166};
t4191 = ct{1167};
t4195 = ct{1168};
t4196 = ct{1169};
t4197 = ct{1170};
t4198 = ct{1171};
t42 = ct{1172};
t4204 = ct{1173};
t4205 = ct{1174};
t4206 = ct{1175};
t4207 = ct{1176};
t4212 = ct{1177};
t4214 = ct{1178};
t4215 = ct{1179};
t4219 = ct{1180};
t4220 = ct{1181};
t4221 = ct{1182};
t4225 = ct{1183};
t4228 = ct{1184};
t4230 = ct{1185};
t4231 = ct{1186};
t4233 = ct{1187};
t4234 = ct{1188};
t4235 = ct{1189};
t4236 = ct{1190};
t4241 = ct{1191};
t4242 = ct{1192};
t4244 = ct{1193};
t4249 = ct{1194};
t4250 = ct{1195};
t4251 = ct{1196};
t4253 = ct{1197};
t4254 = ct{1198};
t4257 = ct{1199};
t4259 = ct{1200};
t4262 = ct{1201};
t4263 = ct{1202};
t4272 = ct{1203};
t4273 = ct{1204};
t4277 = ct{1205};
t4279 = ct{1206};
t4280 = ct{1207};
t4281 = ct{1208};
t4283 = ct{1209};
t4285 = ct{1210};
t4286 = ct{1211};
t4288 = ct{1212};
t429 = ct{1213};
t4290 = ct{1214};
t4292 = ct{1215};
t4295 = ct{1216};
t4298 = ct{1217};
t4299 = ct{1218};
t43 = ct{1219};
t4300 = ct{1220};
t4302 = ct{1221};
t4304 = ct{1222};
t4308 = ct{1223};
t4310 = ct{1224};
t4317 = ct{1225};
t4318 = ct{1226};
t4321 = ct{1227};
t4322 = ct{1228};
t4323 = ct{1229};
t4324 = ct{1230};
t4327 = ct{1231};
t4328 = ct{1232};
t4329 = ct{1233};
t4330 = ct{1234};
t4333 = ct{1235};
t4334 = ct{1236};
t4336 = ct{1237};
t4337 = ct{1238};
t4338 = ct{1239};
t4339 = ct{1240};
t4340 = ct{1241};
t4342 = ct{1242};
t4344 = ct{1243};
t4346 = ct{1244};
t4347 = ct{1245};
t4348 = ct{1246};
t4349 = ct{1247};
t4350 = ct{1248};
t4351 = ct{1249};
t4352 = ct{1250};
t4355 = ct{1251};
t4356 = ct{1252};
t4360 = ct{1253};
t4362 = ct{1254};
t4363 = ct{1255};
t4364 = ct{1256};
t4365 = ct{1257};
t4366 = ct{1258};
t4367 = ct{1259};
t4368 = ct{1260};
t4371 = ct{1261};
t4399 = ct{1262};
t4401 = ct{1263};
t4404 = ct{1264};
t4405 = ct{1265};
t4407 = ct{1266};
t4408 = ct{1267};
t4412 = ct{1268};
t4413 = ct{1269};
t4415 = ct{1270};
t4416 = ct{1271};
t4417 = ct{1272};
t4418 = ct{1273};
t4419 = ct{1274};
t4420 = ct{1275};
t4421 = ct{1276};
t4425 = ct{1277};
t4426 = ct{1278};
t4427 = ct{1279};
t4428 = ct{1280};
t4429 = ct{1281};
t4430 = ct{1282};
t4431 = ct{1283};
t4432 = ct{1284};
t4434 = ct{1285};
t4435 = ct{1286};
t4436 = ct{1287};
t4437 = ct{1288};
t4439 = ct{1289};
t4441 = ct{1290};
t4444 = ct{1291};
t4446 = ct{1292};
t4447 = ct{1293};
t4449 = ct{1294};
t4450 = ct{1295};
t4451 = ct{1296};
t4453 = ct{1297};
t4454 = ct{1298};
t4455 = ct{1299};
t4456 = ct{1300};
t4458 = ct{1301};
t4460 = ct{1302};
t4462 = ct{1303};
t4463 = ct{1304};
t4468 = ct{1305};
t4471 = ct{1306};
t4473 = ct{1307};
t4474 = ct{1308};
t4476 = ct{1309};
t4479 = ct{1310};
t4480 = ct{1311};
t4483 = ct{1312};
t4484 = ct{1313};
t4489 = ct{1314};
t4496 = ct{1315};
t4500 = ct{1316};
t4573 = ct{1317};
t4574 = ct{1318};
t4579 = ct{1319};
t4587 = ct{1320};
t4589 = ct{1321};
t4591 = ct{1322};
t4594 = ct{1323};
t4599 = ct{1324};
t46 = ct{1325};
t4602 = ct{1326};
t4604 = ct{1327};
t4607 = ct{1328};
t4610 = ct{1329};
t4611 = ct{1330};
t4614 = ct{1331};
t4615 = ct{1332};
t4617 = ct{1333};
t4620 = ct{1334};
t4640 = ct{1335};
t4641 = ct{1336};
t4642 = ct{1337};
t4644 = ct{1338};
t4645 = ct{1339};
t4647 = ct{1340};
t4648 = ct{1341};
t4649 = ct{1342};
t4650 = ct{1343};
t4652 = ct{1344};
t4653 = ct{1345};
t4654 = ct{1346};
t4655 = ct{1347};
t4661 = ct{1348};
t4662 = ct{1349};
t4663 = ct{1350};
t4664 = ct{1351};
t4667 = ct{1352};
t4669 = ct{1353};
t4678 = ct{1354};
t4679 = ct{1355};
t4680 = ct{1356};
t4682 = ct{1357};
t4683 = ct{1358};
t4686 = ct{1359};
t4687 = ct{1360};
t4688 = ct{1361};
t4689 = ct{1362};
t4690 = ct{1363};
t4691 = ct{1364};
t4692 = ct{1365};
t4693 = ct{1366};
t4694 = ct{1367};
t4695 = ct{1368};
t4696 = ct{1369};
t4697 = ct{1370};
t4698 = ct{1371};
t4699 = ct{1372};
t47 = ct{1373};
t4700 = ct{1374};
t4701 = ct{1375};
t4702 = ct{1376};
t4703 = ct{1377};
t4704 = ct{1378};
t4705 = ct{1379};
t4716 = ct{1380};
t4742 = ct{1381};
t4758 = ct{1382};
t4764 = ct{1383};
t4772 = ct{1384};
t4777 = ct{1385};
t4779 = ct{1386};
t4780 = ct{1387};
t4785 = ct{1388};
t4787 = ct{1389};
t4789 = ct{1390};
t4790 = ct{1391};
t4791 = ct{1392};
t4792 = ct{1393};
t4795 = ct{1394};
t4811 = ct{1395};
t4813 = ct{1396};
t4814 = ct{1397};
t4816 = ct{1398};
t4817 = ct{1399};
t4820 = ct{1400};
t4821 = ct{1401};
t4822 = ct{1402};
t4823 = ct{1403};
t4826 = ct{1404};
t4829 = ct{1405};
t4830 = ct{1406};
t4831 = ct{1407};
t4832 = ct{1408};
t4837 = ct{1409};
t4838 = ct{1410};
t4839 = ct{1411};
t4840 = ct{1412};
t4841 = ct{1413};
t4842 = ct{1414};
t4860 = ct{1415};
t4865 = ct{1416};
t4868 = ct{1417};
t4869 = ct{1418};
t4870 = ct{1419};
t4871 = ct{1420};
t4872 = ct{1421};
t4873 = ct{1422};
t4898 = ct{1423};
t4911 = ct{1424};
t4931 = ct{1425};
t4963 = ct{1426};
t4964 = ct{1427};
t4965 = ct{1428};
t4966 = ct{1429};
t4974 = ct{1430};
t4976 = ct{1431};
t4977 = ct{1432};
t4985 = ct{1433};
t4986 = ct{1434};
t4994 = ct{1435};
t4995 = ct{1436};
t5 = ct{1437};
t50 = ct{1438};
t5001 = ct{1439};
t5002 = ct{1440};
t5005 = ct{1441};
t5007 = ct{1442};
t5010 = ct{1443};
t5013 = ct{1444};
t5014 = ct{1445};
t5017 = ct{1446};
t5021 = ct{1447};
t5023 = ct{1448};
t5026 = ct{1449};
t5030 = ct{1450};
t5035 = ct{1451};
t5036 = ct{1452};
t5037 = ct{1453};
t5038 = ct{1454};
t5039 = ct{1455};
t5040 = ct{1456};
t5041 = ct{1457};
t5042 = ct{1458};
t5043 = ct{1459};
t5044 = ct{1460};
t5045 = ct{1461};
t5046 = ct{1462};
t5047 = ct{1463};
t5048 = ct{1464};
t5049 = ct{1465};
t5050 = ct{1466};
t5058 = ct{1467};
t5061 = ct{1468};
t5144 = ct{1469};
t5145 = ct{1470};
t5153 = ct{1471};
t5159 = ct{1472};
t5167 = ct{1473};
t5168 = ct{1474};
t5169 = ct{1475};
t5189 = ct{1476};
t5191 = ct{1477};
t5197 = ct{1478};
t5199 = ct{1479};
t5202 = ct{1480};
t5207 = ct{1481};
t5219 = ct{1482};
t5221 = ct{1483};
t5223 = ct{1484};
t5224 = ct{1485};
t5225 = ct{1486};
t5226 = ct{1487};
t5227 = ct{1488};
t5229 = ct{1489};
t5230 = ct{1490};
t5231 = ct{1491};
t5233 = ct{1492};
t5235 = ct{1493};
t5236 = ct{1494};
t5239 = ct{1495};
t5240 = ct{1496};
t5241 = ct{1497};
t5243 = ct{1498};
t5244 = ct{1499};
t5245 = ct{1500};
t5246 = ct{1501};
t5247 = ct{1502};
t5248 = ct{1503};
t5252 = ct{1504};
t5254 = ct{1505};
t5255 = ct{1506};
t5257 = ct{1507};
t5265 = ct{1508};
t5266 = ct{1509};
t5301 = ct{1510};
t5302 = ct{1511};
t5306 = ct{1512};
t5308 = ct{1513};
t5316 = ct{1514};
t5317 = ct{1515};
t5320 = ct{1516};
t5328 = ct{1517};
t5337 = ct{1518};
t5338 = ct{1519};
t5339 = ct{1520};
t5340 = ct{1521};
t5342 = ct{1522};
t5344 = ct{1523};
t5345 = ct{1524};
t5346 = ct{1525};
t5347 = ct{1526};
t5348 = ct{1527};
t5349 = ct{1528};
t5350 = ct{1529};
t5361 = ct{1530};
t5362 = ct{1531};
t5377 = ct{1532};
t5379 = ct{1533};
t5380 = ct{1534};
t5381 = ct{1535};
t5383 = ct{1536};
t5384 = ct{1537};
t5388 = ct{1538};
t5389 = ct{1539};
t5399 = ct{1540};
t5402 = ct{1541};
t5403 = ct{1542};
t5405 = ct{1543};
t5407 = ct{1544};
t5411 = ct{1545};
t5427 = ct{1546};
t5428 = ct{1547};
t5433 = ct{1548};
t5434 = ct{1549};
t5440 = ct{1550};
t5441 = ct{1551};
t5443 = ct{1552};
t5444 = ct{1553};
t5480 = ct{1554};
t5481 = ct{1555};
t5482 = ct{1556};
t5483 = ct{1557};
t5484 = ct{1558};
t5485 = ct{1559};
t5486 = ct{1560};
t5487 = ct{1561};
t5488 = ct{1562};
t5489 = ct{1563};
t5490 = ct{1564};
t5491 = ct{1565};
t5492 = ct{1566};
t5493 = ct{1567};
t5494 = ct{1568};
t5496 = ct{1569};
t5498 = ct{1570};
t5500 = ct{1571};
t5510 = ct{1572};
t5517 = ct{1573};
t5518 = ct{1574};
t5524 = ct{1575};
t5531 = ct{1576};
t5552 = ct{1577};
t5578 = ct{1578};
t5580 = ct{1579};
t56 = ct{1580};
t5620 = ct{1581};
t5626 = ct{1582};
t5627 = ct{1583};
t5631 = ct{1584};
t5670 = ct{1585};
t5671 = ct{1586};
t5674 = ct{1587};
t5675 = ct{1588};
t5678 = ct{1589};
t5679 = ct{1590};
t5694 = ct{1591};
t5695 = ct{1592};
t5702 = ct{1593};
t5703 = ct{1594};
t5719 = ct{1595};
t5722 = ct{1596};
t5723 = ct{1597};
t58 = ct{1598};
t5835 = ct{1599};
t5839 = ct{1600};
t5840 = ct{1601};
t59 = ct{1602};
t5932 = ct{1603};
t5951 = ct{1604};
t5953 = ct{1605};
t5954 = ct{1606};
t6 = ct{1607};
t60 = ct{1608};
t6183 = ct{1609};
t6184 = ct{1610};
t6185 = ct{1611};
t6219 = ct{1612};
t6221 = ct{1613};
t6247 = ct{1614};
t6253 = ct{1615};
t628 = ct{1616};
t635 = ct{1617};
t636 = ct{1618};
t638 = ct{1619};
t640 = ct{1620};
t641 = ct{1621};
t642 = ct{1622};
t643 = ct{1623};
t645 = ct{1624};
t646 = ct{1625};
t6484 = ct{1626};
t6485 = ct{1627};
t6486 = ct{1628};
t649 = ct{1629};
t654 = ct{1630};
t6543 = ct{1631};
t6544 = ct{1632};
t655 = ct{1633};
t656 = ct{1634};
t657 = ct{1635};
t659 = ct{1636};
t660 = ct{1637};
t663 = ct{1638};
t664 = ct{1639};
t665 = ct{1640};
t6658 = ct{1641};
t666 = ct{1642};
t6663 = ct{1643};
t667 = ct{1644};
t668 = ct{1645};
t669 = ct{1646};
t67 = ct{1647};
t670 = ct{1648};
t672 = ct{1649};
t673 = ct{1650};
t674 = ct{1651};
t675 = ct{1652};
t676 = ct{1653};
t677 = ct{1654};
t678 = ct{1655};
t679 = ct{1656};
t68 = ct{1657};
t681 = ct{1658};
t6811 = ct{1659};
t6812 = ct{1660};
t6813 = ct{1661};
t682 = ct{1662};
t683 = ct{1663};
t684 = ct{1664};
t685 = ct{1665};
t686 = ct{1666};
t687 = ct{1667};
t689 = ct{1668};
t6892 = ct{1669};
t6893 = ct{1670};
t691 = ct{1671};
t692 = ct{1672};
t693 = ct{1673};
t694 = ct{1674};
t7 = ct{1675};
t70 = ct{1676};
t702 = ct{1677};
t7041 = ct{1678};
t707 = ct{1679};
t708 = ct{1680};
t71 = ct{1681};
t710 = ct{1682};
t715 = ct{1683};
t716 = ct{1684};
t717 = ct{1685};
t718 = ct{1686};
t721 = ct{1687};
t722 = ct{1688};
t724 = ct{1689};
t725 = ct{1690};
t73 = ct{1691};
t736 = ct{1692};
t738 = ct{1693};
t740 = ct{1694};
t741 = ct{1695};
t749 = ct{1696};
t756 = ct{1697};
t76 = ct{1698};
t762 = ct{1699};
t768 = ct{1700};
t777 = ct{1701};
t792 = ct{1702};
t793 = ct{1703};
t801 = ct{1704};
t802 = ct{1705};
t808 = ct{1706};
t813 = ct{1707};
t819 = ct{1708};
t821 = ct{1709};
t850 = ct{1710};
t855 = ct{1711};
t874 = ct{1712};
t878 = ct{1713};
t89 = ct{1714};
t90 = ct{1715};
t91 = ct{1716};
t92 = ct{1717};
t941 = ct{1718};
t944 = ct{1719};
t948 = ct{1720};
t951 = ct{1721};
t97 = ct{1722};
t5681 = t3877.*t3901.*t3941.*(t1513+t1879+t2598+t2820+t2834+t3117+t3118).*(-7.26735e-3);
t5682 = t3941.*(t2674-t2676+t3022-t3027).*(t2694-t2701+t3036-t3043).*(t1513+t1879+t2598+t2820+t2834+t3117+t3118).*(-7.26735e-3);
t5700 = t3877.*t3901.*t4149.*(t1488+t1874+t2519+t2740+t2747+t3096+t3097).*(-7.26735e-3);
t5701 = t4149.*(t2674-t2676+t3022-t3027).*(t2694-t2701+t3036-t3043).*(t1488+t1874+t2519+t2740+t2747+t3096+t3097).*(-7.26735e-3);
t5720 = -t5719;
t5791 = t3901.*t4175.*t5223.*1.08769e-2;
t5792 = t4175.*t5224.*(t2694-t2701+t3036-t3043).*(-1.08769e-2);
t5852 = t4333+t4334+t4340+t4349;
t5853 = t4342+t4347+t4348+t4350;
t5890 = t3877.*t4134.*t5485;
t5891 = -t4134.*t5486.*(t2674-t2676+t3022-t3027);
et69 = -t2748-t2749+t2773+t2781-t2788+t3204+t3458+t3997-t4009+t262.*(t46-t47).*2.075672598245148e-23;
et70 = t264.*(t46-t47).*1.875105520197095e-20;
t5930 = -t3617.*t3877.*(et69+et70);
et71 = t50.*t189.*(-t4447+t4458+t3385.*(t2813-t2835+t18.*(t1456-t2355).*1.02e-6+t23.*(t1456-t2355).*9.0e-8)+t3386.*(-t2804+t2838+t3109+t23.*(t1456-t2355).*9.3e-7));
et72 = -9.543032792050485e-17;
t5994 = et71.*et72;
t6003 = -t2297.*(-t4447+t4458+t3385.*(t2813-t2835+t18.*(t1456-t2355).*1.02e-6+t23.*(t1456-t2355).*9.0e-8)+t3386.*(-t2804+t2838+t3109+t23.*(t1456-t2355).*9.3e-7));
t6004 = t2297.*(-t4447+t4458+t3385.*(t2813-t2835+t18.*(t1456-t2355).*1.02e-6+t23.*(t1456-t2355).*9.0e-8)+t3386.*(-t2804+t2838+t3109+t23.*(t1456-t2355).*9.3e-7));
t6013 = -t3047.*(-t4447+t4458+t3385.*(t2813-t2835+t18.*(t1456-t2355).*1.02e-6+t23.*(t1456-t2355).*9.0e-8)+t3386.*(-t2804+t2838+t3109+t23.*(t1456-t2355).*9.3e-7));
t6017 = t3047.*(-t4447+t4458+t3385.*(t2813-t2835+t18.*(t1456-t2355).*1.02e-6+t23.*(t1456-t2355).*9.0e-8)+t3386.*(-t2804+t2838+t3109+t23.*(t1456-t2355).*9.3e-7));
t6029 = t4172+t4174+t4964+t4966;
t6033 = -t201.*(t4173+t4965+t123.*t188.*(t2694-t2701+t3036-t3043).*2.442490654175345e-23+t50.*t189.*t4860.*(t42-t43).*2.711709361697228e-39);
t6206 = t3877.*t4134.*t5840;
t6207 = -t4134.*t5839.*(t2674-t2676+t3022-t3027);
t6209 = t4134.*t5839.*(t2674-t2676+t3022-t3027);
t6325 = t3901.*t4175.*(t1554+t2361+t2362+t2367+t2414+t3928+t3934+t4160+t4163+t17.*(-t1901+t3122+t3270).*5.68686e-3).*(-1.08769e-2);
t6339 = t3901.*t4175.*t5954.*1.08769e-2;
t6340 = t4175.*t5953.*(t2694-t2701+t3036-t3043).*(-1.08769e-2);
t6341 = t4175.*t5953.*(t2694-t2701+t3036-t3043).*1.08769e-2;
et73 = -t2137+t2777+t2778+t2779-t2787+t4012-t4205+t4207+t27.*(t1959-t3306+t38.*t1022.*(t855-t878).*2.196325630278387e-1).*6.1855407534e-5;
et74 = t33.*(t1959-t3306+t38.*t1022.*(t855-t878).*2.196325630278387e-1).*1.35652563578e-4;
t6367 = t4134.*(et73+et74).*(t2674-t2676+t3022-t3027);
t6507 = -t3891.*t6183.*(t2674-t2676+t3022-t3027);
et75 = t1288+t1289+t1302+t1303-t1319-t1320+t1336-t1348+t1350+t1351-t1360+t1369-t1378+t1396-t1425+t1435-t2174+t2183-t2187+t2193-t2194-t2195+t2199-t2203-t2215+t2219-t2222-t2223+t2239+t2240-t2256-t2257+t2555+t2556+t2572+t2583-t2605-t2606+t2612+t2613-t2618-t2619+t2651+t2652;
et76 = t24.*t25.*t26.*t50.*t202.*(-3.566935413776081e-21);
et77 = t30.*t31.*t32.*t50.*t202.*(-3.992732227073824e-24);
et78 = t24.*t25.*t32.*t33.*t50.*t202.*(-3.509445006623964e-21);
et79 = t27.*t30.*t31.*t32.*t50.*t202.*(-7.696420262413979e-21);
t6508 = -t3877.*t3891.*(et75+et76+et77+et78+et79);
et80 = t1288+t1289+t1302+t1303-t1319-t1320+t1336-t1348+t1350+t1351-t1360+t1369-t1378+t1396-t1425+t1435-t2174+t2183-t2187+t2193-t2194-t2195+t2199-t2203-t2215+t2219-t2222-t2223+t2239+t2240-t2256-t2257+t2555+t2556+t2572+t2583-t2605-t2606+t2612+t2613-t2618-t2619+t2651+t2652;
et81 = t24.*t25.*t26.*t50.*t202.*(-3.566935413776081e-21);
et82 = t30.*t31.*t32.*t50.*t202.*(-3.992732227073824e-24);
et83 = t24.*t25.*t32.*t33.*t50.*t202.*(-3.509445006623964e-21);
et84 = t27.*t30.*t31.*t32.*t50.*t202.*(-7.696420262413979e-21);
t6511 = t3877.*t3891.*(et80+et81+et82+et83+et84);
t6689 = t4134.*t4822.*t6183;
et85 = -t2306-t2317+t3144+t3147+t35.*t941.*t948.*(t850-t874).*3.775747223193135e-1;
et86 = t36.*t941.*t948.*(t850-t874).*2.244797987218524e-1;
et87 = t1288+t1289+t1302+t1303-t1319-t1320+t1336-t1348+t1350+t1351-t1360+t1369-t1378+t1396-t1425+t1435-t2174+t2183-t2187+t2193-t2194-t2195+t2199-t2203-t2215+t2219-t2222-t2223+t2239+t2240-t2256-t2257+t2555+t2556+t2572+t2583-t2605-t2606+t2612+t2613-t2618-t2619+t2651+t2652;
et88 = t24.*t25.*t26.*t50.*t202.*(-3.566935413776081e-21);
et89 = t30.*t31.*t32.*t50.*t202.*(-3.992732227073824e-24);
et90 = t24.*t25.*t32.*t33.*t50.*t202.*(-3.509445006623964e-21);
et91 = t27.*t30.*t31.*t32.*t50.*t202.*(-7.696420262413979e-21);
t6692 = t4134.*(et85+et86).*(et87+et88+et89+et90+et91);
et92 = -t2137+t2777+t2778+t2779-t2787+t4012-t4205+t4207+t27.*(t1959-t3306+t38.*t1022.*(t855-t878).*2.196325630278387e-1).*6.1855407534e-5;
et93 = t33.*(t1959-t3306+t38.*t1022.*(t855-t878).*2.196325630278387e-1).*1.35652563578e-4;
t6914 = -t5951.*(et92+et93);
et94 = -t2137+t2777+t2778+t2779-t2787+t4012-t4205+t4207+t27.*(t1959-t3306+t38.*t1022.*(t855-t878).*2.196325630278387e-1).*6.1855407534e-5;
et95 = t33.*(t1959-t3306+t38.*t1022.*(t855-t878).*2.196325630278387e-1).*1.35652563578e-4;
t6916 = t5951.*(et94+et95);
t7197 = t4687+t4690+t4691+t4692+t5035+t5040+t5043+t5047;
t7199 = t4694+t4696+t4700+t4701+t5039+t5041+t5049+t5050;
et96 = t50.*t202.*(t4686-t5035+t5038-t5040-t5047+t3880.*(t2694-t2701+t3036-t3043).*5.0e-8+t3901.*(-t1881+t3121+t3269).*5.0e-8+t3901.*(-t1901+t3122+t3270).*1.1e-7);
et97 = -9.543032792050485e-17;
t7204 = et96.*et97;
et98 = t50.*t202.*(t4686-t5035+t5038-t5040-t5047+t3880.*(t2694-t2701+t3036-t3043).*5.0e-8+t3901.*(-t1881+t3121+t3269).*5.0e-8+t3901.*(-t1901+t3122+t3270).*1.1e-7);
et99 = 9.543032792050485e-17;
t7205 = et98.*et99;
et100 = t50.*t202.*(t4699-t5039-t5041+t5048-t5049+t3880.*(t2694-t2701+t3036-t3043).*1.6e-7+t3901.*(-t1881+t3121+t3269).*1.6e-7+t3901.*(-t1901+t3122+t3270).*5.0e-8);
et101 = -5.673626844500105e-17;
t7206 = et100.*et101;
t3286 = -t3275;
t3292 = -t3282;
t3295 = -t3285;
t3298 = -t3294;
t3307 = -t3301;
t3309 = -t3304;
t3310 = -t3305;
t3337 = -t3329;
t3340 = -t3332;
t3345 = -t3339;
t3357 = -t3350;
t3358 = -t3352;
t3404 = -t3394;
t3405 = -t3397;
t3413 = -t3410;
t3414 = -t3412;
t3491 = t18.*t3483;
t3492 = -t3485;
t3493 = t23.*t3483;
t3496 = t17.*t3484;
t3497 = t18.*t3484;
t3499 = t22.*t3484;
t3500 = t23.*t3484;
t3506 = t3485.*(3.0./5.0e+2);
t3508 = t3487.*(3.0./5.0e+2);
t3513 = t22.*t3483.*(3.0./5.0e+2);
t3530 = t50.*t202.*t3242.*8.875020496606951e-23;
t3532 = -t3529;
t3539 = -t3534;
t3542 = t50.*t202.*t3242.*8.588729512845436e-24;
t3543 = t28.*t3528;
t3544 = t34.*t3528;
t3545 = t27.*t3531;
t3546 = t28.*t3531;
t3548 = t33.*t3531;
t3549 = t34.*t3531;
t3553 = t3535.*(3.0./5.0e+2);
t3555 = t3537.*(3.0./5.0e+2);
t3564 = t33.*t3528.*(3.0./5.0e+2);
t3570 = t3486.*9.99471e-3;
t3571 = t3488.*1.838876e-2;
t3572 = t3485.*1.247162e-2;
t3573 = t3487.*1.247162e-2;
t3574 = t3485.*5.68686e-3;
t3575 = t3487.*5.68686e-3;
t3591 = t17.*t3483.*1.247162e-2;
t3592 = t3485.*3.131399999999998e-4;
t3593 = t3487.*3.131399999999998e-4;
t3594 = t22.*t3483.*5.68686e-3;
t3613 = t22.*t3483.*3.131399999999998e-4;
t3618 = t3536.*9.99471e-3;
t3619 = t3538.*1.838876e-2;
t3620 = t3535.*1.247162e-2;
t3621 = t3537.*1.247162e-2;
t3636 = t27.*t3528.*1.247162e-2;
t3637 = t3535.*3.131399999999998e-4;
t3638 = t3537.*3.131399999999998e-4;
t3648 = t3563.*(-1.838876e-2);
t3649 = t3535.*4.36041e-5;
t3650 = t3537.*4.36041e-5;
t3652 = t33.*t3528.*3.131399999999998e-4;
t3658 = t33.*t3528.*4.36041e-5;
t3664 = -t3659;
t3691 = t3535.*1.35652563578e-4;
t3692 = t3537.*1.35652563578e-4;
t3693 = t3538.*1.33637554986e-4;
t3694 = t3536.*7.26350557185e-5;
t3695 = t3535.*6.1855407534e-5;
t3696 = t3537.*6.1855407534e-5;
t3706 = t2363.*t3242.*9.3e-7;
t3708 = t27.*t3528.*1.35652563578e-4;
t3714 = t33.*t3528.*6.1855407534e-5;
t3724 = t2363.*t3242.*9.0e-8;
t3727 = t3563.*(-1.33637554986e-4);
t3744 = -t3743;
t3797 = -t3796;
t3801 = t3057.*t3242.*9.3e-7;
t3803 = -t3800;
t3806 = t3057.*t3242.*9.0e-8;
t3824 = -t3812;
t3825 = -t3813;
t3829 = t2973.*t3528;
t3830 = t2971.*t3531;
t3831 = t2972.*t3531;
t3835 = t2973.*t3531;
t3841 = t2976.*t3528;
t3857 = -t3528.*(t1545-t2615);
t3860 = t3528.*(t1545-t2615);
t3861 = -t3858;
t3868 = t3119.*t3528;
t3875 = t27.*t3132.*t3528;
t3897 = t3154.*t3528;
t3899 = t3154.*t3531;
t3922 = -t3919;
t3942 = t3215+t3487;
t3959 = t3206.*t3528;
t3977 = -t3975;
t3979 = (t3230.*t3483)./1.0e+8;
t3981 = (t3230.*t3484)./1.0e+8;
t3983 = t17.*t3230.*t3483.*(-1.0e-8);
t3985 = t3233+t3537;
t3986 = t3241+t3535;
t4024 = -t4020;
t4027 = t3230.*t3483.*9.840000000000001e-6;
t4032 = t3230.*t3484.*9.840000000000001e-6;
t4039 = -t4029;
t4041 = -t4030;
t4047 = t3230.*t3483.*6.2e-7;
t4050 = t3230.*t3483.*3.24e-6;
t4051 = t3230.*t3483.*7.83e-6;
t4053 = t3230.*t3484.*6.2e-7;
t4055 = t3230.*t3484.*3.24e-6;
t4057 = t3230.*t3484.*7.83e-6;
t4061 = t22.*t3230.*t3483.*5.7e-7;
t4062 = t17.*t3230.*t3483.*1.02e-6;
t4065 = t17.*t3230.*t3483.*2.4e-7;
t4067 = t17.*t3230.*t3483.*4.0e-8;
t4068 = t22.*t3230.*t3483.*4.0e-8;
t4078 = t34.*(t3235-t3535).*(-9.99471e-3);
t4079 = t28.*(t3235-t3535).*(-1.838876e-2);
t4101 = -t4087;
t4135 = t28.*(t3235-t3535).*(-1.33637554986e-4);
t4136 = t34.*(t3235-t3535).*(-7.26350557185e-5);
t4140 = -t4133;
t4150 = -t4144;
t4151 = t4087.*9.99471e-3;
t4152 = t4088.*1.838876e-2;
t4161 = -t4154;
t4168 = t3420.*t3528;
t4178 = -t4176;
t4179 = t4131.*9.99471e-3;
t4181 = t4133.*1.838876e-2;
t4189 = -t4185;
t4190 = -t4187;
t4199 = t3468.*t3528;
t4200 = t3468.*t3531;
t4201 = -t4198;
t4208 = t4131.*7.26350557185e-5;
t4210 = -t4204;
t4213 = t4133.*1.33637554986e-4;
t4222 = t3486+t3495;
t4223 = t3488+t3505;
t4227 = -t4225;
t4229 = -t4228;
t4237 = (t3483.*t3528)./1.0e+8;
t4238 = (t3484.*t3528)./1.0e+8;
t4239 = (t3483.*t3531)./1.0e+8;
t4243 = -t4241;
t4245 = t3536+t3552;
t4246 = t3538+t3563;
t4252 = t3483.*t3528.*6.2e-7;
t4255 = t3484.*t3528.*6.2e-7;
t4256 = t3483.*t3531.*6.2e-7;
t4260 = t22.*t3483.*t3528.*5.7e-7;
t4261 = t17.*t3483.*t3528.*1.02e-6;
t4264 = t17.*t3483.*t3528.*2.4e-7;
t4265 = t17.*t3483.*t3528.*4.0e-8;
t4266 = t22.*t3483.*t3528.*4.0e-8;
t4274 = t17.*t2297.*(t3235-t3535).*(-1.02e-6);
t4278 = t2300+t2313+t3285+t3304;
t4287 = t33.*t3528.*t3789;
t4291 = -t4290;
t4294 = -t4292;
t4296 = -t3063.*(t3235-t3535);
t4306 = -t3132.*(t3235-t3535);
t4309 = (t1953-t2828).*(t3235-t3535);
t4319 = t2962+t3519+t3523;
t4326 = t2753+t2792+t3398+t3411;
t4400 = t3385.*t3943;
t4403 = t3386.*t3945;
t4409 = t27.*t3528.*t3863;
t4410 = -t4408;
t4422 = -t4418;
t4423 = -t4419;
t4424 = -t4420;
t4438 = (t3483.*t3901)./1.0e+8;
t4440 = (t3483.*t3904)./1.0e+8;
t4442 = (t3484.*t3901)./1.0e+8;
t4452 = t3483.*t3901.*9.840000000000001e-6;
t4459 = t3484.*t3901.*9.840000000000001e-6;
t4461 = t3484.*t3904.*9.840000000000001e-6;
t4464 = t3483.*t3901.*6.2e-7;
t4465 = t3483.*t3901.*3.24e-6;
t4466 = t3483.*t3901.*7.83e-6;
t4469 = t3483.*t3904.*3.24e-6;
t4470 = t3484.*t3901.*6.2e-7;
t4472 = t3483.*t3904.*7.83e-6;
t4475 = t3483.*t3904.*6.2e-7;
t4477 = t3484.*t3901.*3.24e-6;
t4478 = t3484.*t3901.*7.83e-6;
t4481 = t22.*t3483.*t3901.*5.7e-7;
t4482 = t17.*t3483.*t3901.*1.02e-6;
t4487 = t17.*t3483.*t3901.*2.4e-7;
t4488 = t17.*t3483.*t3901.*4.0e-8;
t4490 = t22.*t3483.*t3901.*4.0e-8;
t4581 = -t4573;
t4582 = (t3235-t3535).*(t335-t1539-t2831+t2851);
t4583 = t17.*(t1861-t3214).*(t3235-t3535).*1.02e-6;
t4588 = t3483.*t4108;
t4592 = t3528.*(t951+t16.*(-t1881+t3121+t3269)).*(-1.0e-8);
t4593 = (t3528.*(t951+t16.*(-t1881+t3121+t3269)))./1.0e+8;
t4596 = (t3483.*t4113)./1.0e+8;
t4605 = t3528.*(t951+t16.*(-t1881+t3121+t3269)).*(-6.2e-7);
t4606 = t3528.*(t951+t16.*(-t1881+t3121+t3269)).*6.2e-7;
t4608 = t3483.*t4113.*6.2e-7;
t4612 = t3528.*t4149.*7.26735e-3;
t4621 = -t3789.*(t3235-t3535);
t4624 = -t3793.*(t3235-t3535);
t4656 = -t3843.*(t3235-t3535);
t4658 = t3843.*(t3235-t3535);
t4665 = t3209.*t4366;
t4666 = t3210.*t4366;
t4671 = -t3863.*(t3235-t3535);
t4673 = t3863.*(t3235-t3535);
t4676 = t3483.*t4302;
t4684 = t3229.*t4401.*7.26735e-3;
t4685 = t3230.*t4401.*7.26735e-3;
t4770 = t3528.*t4323.*7.26735e-3;
t4781 = t18.*t4777;
t4782 = t23.*t4777;
t4786 = t3483.*t4365;
t4824 = t3913+t4138;
t4861 = t4841.*9.99471e-3;
t4862 = t4840.*1.838876e-2;
t4874 = t3528.*t4399.*7.26735e-3;
t4876 = t28.*(t3235-t3535).*(t2813-t2835+t18.*(t1456-t2355).*1.02e-6+t23.*(t1456-t2355).*9.0e-8);
t4877 = t34.*(t3235-t3535).*(-t2804+t2838+t3109+t23.*(t1456-t2355).*9.3e-7);
t4889 = t4841.*7.26350557185e-5;
t4891 = t4840.*1.33637554986e-4;
t4961 = t3209.*t4648;
t4962 = t3210.*t4648;
t4982 = t3229.*t4654.*7.26735e-3;
t4983 = t3230.*t4654.*7.26735e-3;
t4987 = t855.*t4977;
t4988 = t50.*t202.*t4977.*(-1.110223024625157e-16);
t4996 = -t4653.*(t1861-t3214);
t4997 = t3483.*t4653;
t4999 = t3132.*t4814;
t5011 = (t3229.*t4780)./1.0e+8;
t5015 = t3229.*t4777.*5.7e-7;
t5018 = t3229.*t4780.*1.02e-6;
t5020 = t3229.*t4777.*4.0e-8;
t5024 = t3229.*t4780.*2.4e-7;
t5028 = t3229.*t4780.*4.0e-8;
t5031 = t4662.*(t1896-t3232).*(-7.26735e-3);
t5032 = t4662.*(t1896-t3232).*7.26735e-3;
t5033 = t3528.*t4662.*7.26735e-3;
t5063 = t3483.*t4758;
t5064 = -t5058;
t5069 = t3484.*t4758;
t5090 = t3818+t3832+t3900;
t5092 = t645+t646+t666+t683+t1576+t1579+t1584+t1585+t2291+t2311+t2682+t3029+t3281+t3300;
t5094 = t3528.*(t17.*((t237.*(t42-t43))./9.007199254740992e+15+t21.*(-t1881+t3121+t3269))+t22.*(-t1901+t3122+t3270)).*(-1.0e-8);
t5095 = t4780.*(t1896-t3232).*(-1.0e-8);
t5096 = (t4780.*(t1896-t3232))./1.0e+8;
t5110 = t4777.*(t1896-t3232).*(-5.7e-7);
t5115 = t4777.*(t1896-t3232).*5.7e-7;
t5118 = t3528.*(t17.*((t237.*(t42-t43))./9.007199254740992e+15+t21.*(-t1881+t3121+t3269))+t22.*(-t1901+t3122+t3270)).*(-1.02e-6);
t5120 = t4780.*(t1896-t3232).*(-1.02e-6);
t5121 = t3528.*(t17.*((t237.*(t42-t43))./9.007199254740992e+15+t21.*(-t1881+t3121+t3269))+t22.*(-t1901+t3122+t3270)).*(-2.4e-7);
t5122 = t4777.*(t1896-t3232).*(-4.0e-8);
t5123 = t3528.*t4779.*5.7e-7;
t5124 = t4780.*(t1896-t3232).*1.02e-6;
t5125 = t4780.*(t1896-t3232).*(-2.4e-7);
t5126 = t4777.*(t1896-t3232).*4.0e-8;
t5127 = t3528.*(t17.*((t237.*(t42-t43))./9.007199254740992e+15+t21.*(-t1881+t3121+t3269))+t22.*(-t1901+t3122+t3270)).*(-4.0e-8);
t5128 = t4780.*(t1896-t3232).*2.4e-7;
t5129 = t4780.*(t1896-t3232).*(-4.0e-8);
t5130 = t4780.*(t1896-t3232).*4.0e-8;
t5131 = t3528.*t4779.*4.0e-8;
t5146 = -t5144;
t5147 = t3528.*t4795.*7.26735e-3;
t5148 = t3531.*t4795.*7.26735e-3;
t5152 = (t3483.*t4860)./1.0e+8;
t5160 = t3484.*t4860.*9.840000000000001e-6;
t5163 = t3483.*t4860.*3.24e-6;
t5164 = t3483.*t4860.*7.83e-6;
t5165 = t3483.*t4860.*6.2e-7;
t5195 = t3628.*t4277.*(t2694-t2701+t3036-t3043).*(-2.889644e-2);
t5198 = -t5197;
t5201 = -t5199;
t5203 = -t3617.*t4324.*(t2674-t2676+t3022-t3027);
t5205 = t3785+t3995+t4272;
t5206 = t3863.*t4814;
t5222 = t4780.*(t2694-t2701+t3036-t3043).*(-1.0e-8);
t5228 = t4777.*(t2694-t2701+t3036-t3043).*(-5.7e-7);
t5232 = t4780.*(t2694-t2701+t3036-t3043).*(-1.02e-6);
t5234 = t4777.*(t2694-t2701+t3036-t3043).*(-4.0e-8);
t5237 = t4780.*(t2694-t2701+t3036-t3043).*1.02e-6;
t5238 = t4780.*(t2694-t2701+t3036-t3043).*(-2.4e-7);
t5242 = t4780.*(t2694-t2701+t3036-t3043).*(-4.0e-8);
t5249 = t1193+t1194+t1222+t1236+t2138+t2141+t2156+t2157+t2733+t2765+t2948+t3069+t3396+t3407;
t5260 = t4780.*(t3235-t3535).*(-1.02e-6);
t5292 = t4129+t4840;
t5295 = t4139+t4841;
t5391 = t3230.*t5265.*9.3e-7;
t5392 = t3230.*t5265.*9.0e-8;
t5393 = t3230.*t5266.*1.02e-6;
t5395 = t3230.*t5266.*9.0e-8;
t5431 = t2520+t2525+t3464+t3467+t4191+t4195;
t5458 = t3528.*t5265.*9.3e-7;
t5461 = t3528.*t5265.*9.0e-8;
t5462 = t3528.*t5266.*1.02e-6;
t5465 = t3528.*t5266.*9.0e-8;
t5499 = t188.*t5489.*8.595599785252598e-1;
t5504 = t4175.*t4649.*(t2694-t2701+t3036-t3043).*(-1.08769e-2);
t5505 = t4175.*t4649.*(t2694-t2701+t3036-t3043).*1.08769e-2;
t5509 = t1548+t1564+t2326+t2343+t2352+t2353+t2354+t3149+t3369+t3926+t3936;
t5514 = t2307.*t5489;
t5515 = t17.*t2297.*t5489;
t5516 = t2338.*t5489;
t5522 = -t4134.*t4716.*(t2674-t2676+t3022-t3027);
t5523 = t4134.*t4716.*(t2674-t2676+t3022-t3027);
t5535 = t2994.*t5489;
t5550 = t3901.*t5265.*9.3e-7;
t5553 = t3901.*t5265.*9.0e-8;
t5554 = t3901.*t5266.*1.02e-6;
t5556 = t3901.*t5266.*9.0e-8;
t5557 = -t5489.*(t1456-t2355);
t5603 = -(t4840-t34.*(t1005+t26.*(t1941-t3308+t39.*t1022.*(t855-t878).*2.196325630278387e-1))).*(t2813-t2835+t18.*(t1456-t2355).*1.02e-6+t23.*(t1456-t2355).*9.0e-8);
t5633 = t2130+t2160+t2748+t2749+t2788+t2795+t2805+t3205+t3459+t4001+t4009;
t5750 = t3387+t3987+t3993+t3994+t4273;
t5841 = t3743+t3792+t3873+t3919+t4198+t4241;
t5876 = t201.*t5852.*8.595599785252598e-1;
t5879 = t201.*t5853.*5.110348748545983e-1;
t5941 = t1553+t2359+t2365+t2366+t2389+t3921+t3929+t3933+t4162+t4164;
t5977 = t4447+t4449+t4455+t4468;
t5993 = t2137+t2787+t2798+t2799+t2802+t4003+t4005+t4019+t4205+t4212;
t6074 = -t3209.*(t3802+t3813-t4283+t4368+t3165.*(t1959-t3306+t38.*t1022.*(t855-t878).*2.196325630278387e-1)+t3119.*(t1896-t3232));
t6075 = t3209.*(t3802+t3813-t4283+t4368+t3165.*(t1959-t3306+t38.*t1022.*(t855-t878).*2.196325630278387e-1)+t3119.*(t1896-t3232));
t6199 = (t2674-t2676+t3022-t3027).*(t3802+t3813-t4283+t4368+t3165.*(t1959-t3306+t38.*t1022.*(t855-t878).*2.196325630278387e-1)+t3119.*(t1896-t3232));
t6317 = t4716.*t5951;
t6493 = t4649.*t6183;
t6515 = t2309+t2374+t2509+t2532+t2977+t2982+t3894+t4107+t4158+t4165+t4811+t4813;
t6691 = -t6689;
t7009 = t1549+t1565+t2309+t2322+t2327+t2328+t2357+t2375+t2509+t2532+t2977+t2982+t3150+t3370+t3894+t3932+t3935+t4107+t4158+t4165+t4811+t4813;
t7032 = t1554+t2309+t2361+t2362+t2367+t2374+t2414+t2509+t2532+t2977+t2982+t3928+t3934+t3938+t4158+t4160+t4165+t4171+t4811+t4813;
t3501 = t22.*t3491;
t3502 = t22.*t3493;
t3503 = -t3493;
t3507 = -t3499;
t3510 = -t3506;
t3512 = -t3508;
t3515 = t3496.*(3.0./5.0e+2);
t3516 = t3499.*(3.0./5.0e+2);
t3550 = -t3544;
t3554 = -t3548;
t3556 = t33.*t3543;
t3557 = t33.*t3544;
t3562 = -t3555;
t3567 = t3545.*(3.0./5.0e+2);
t3568 = t3548.*(3.0./5.0e+2);
t3580 = -t3571;
t3582 = -t3572;
t3585 = t3491.*9.99471e-3;
t3586 = t3493.*9.99471e-3;
t3587 = t3491.*1.838876e-2;
t3589 = t3493.*1.838876e-2;
t3597 = t3497.*9.99471e-3;
t3601 = t3500.*1.838876e-2;
t3602 = -t3591;
t3603 = t3496.*1.247162e-2;
t3604 = t3499.*1.247162e-2;
t3605 = -t3592;
t3606 = t3496.*5.68686e-3;
t3608 = t3499.*5.68686e-3;
t3615 = t3496.*3.131399999999998e-4;
t3616 = t3499.*3.131399999999998e-4;
t3626 = -t3619;
t3629 = -t3621;
t3631 = t3543.*9.99471e-3;
t3632 = t3544.*9.99471e-3;
t3633 = t3543.*1.838876e-2;
t3635 = t3544.*1.838876e-2;
t3640 = t3546.*9.99471e-3;
t3642 = t3549.*1.838876e-2;
t3643 = t3545.*1.247162e-2;
t3644 = t3548.*1.247162e-2;
t3656 = t3545.*3.131399999999998e-4;
t3657 = t3548.*3.131399999999998e-4;
t3660 = t3545.*4.36041e-5;
t3661 = t3548.*4.36041e-5;
t3698 = -t3691;
t3701 = -t3693;
t3709 = t3543.*1.33637554986e-4;
t3710 = t3544.*1.33637554986e-4;
t3712 = t3543.*7.26350557185e-5;
t3713 = t3544.*7.26350557185e-5;
t3715 = -t3706;
t3716 = t3545.*1.35652563578e-4;
t3717 = t3548.*1.35652563578e-4;
t3719 = t3549.*1.33637554986e-4;
t3720 = t3546.*7.26350557185e-5;
t3721 = t3545.*6.1855407534e-5;
t3722 = -t3714;
t3723 = t3548.*6.1855407534e-5;
t3729 = -t3724;
t3837 = -t3829;
t3838 = -t3831;
t3839 = -t3835;
t3906 = -t3899;
t3946 = t3217+t3492;
t3950 = t18.*t3942;
t3951 = t23.*t3942;
t3957 = t3222+t3496;
t3968 = -t3959;
t3980 = -t3979;
t3982 = t17.*t3979;
t3990 = t28.*t3985;
t3991 = t34.*t3985;
t3992 = t3240+t3545;
t4031 = -t4027;
t4052 = -t4047;
t4059 = -t4053;
t4064 = -t4062;
t4069 = -t4067;
t4070 = -t4068;
t4155 = -t4151;
t4184 = -t4181;
t4202 = -t4199;
t4203 = -t4200;
t4217 = -t4213;
t4240 = t17.*t4237;
t4267 = -t4265;
t4268 = -t4266;
t4305 = t3132.*t3985;
t4314 = -t4309;
t4353 = -t3985.*(t2801-t2850);
tau_c = ft_10({t1005,t1022,t1089,t1104,t1105,t1108,t1115,t1121,t1158,t1159,t1190,t1196,t1205,t1207,t1208,t1210,t1212,t1214,t1217,t1218,t1219,t1220,t1221,t123,t1230,t1235,t1237,t1238,t1288,t1289,t1302,t1303,t1319,t1320,t1336,t1348,t1350,t1351,t1360,t1369,t1378,t1396,t14,t140,t1425,t1435,t1456,t1477,t1488,t15,t1513,t1539,t1544,t1547,t1548,t1553,t1554,t1559,t1564,t1576,t1577,t1578,t1579,t1581,t1584,t1585,t1586,t1587,t1591,t1595,t1596,t1598,t1599,t16,t1600,t1601,t1602,t1604,t1605,t1606,t1607,t1608,t1609,t1612,t1613,t1614,t1615,t1616,t1626,t1627,t1628,t1629,t1631,t1637,t1640,t1641,t1648,t1649,t1659,t1660,t1661,t1666,t1667,t1683,t1686,t1690,t1692,t17,t1700,t1701,t1703,t1704,t1705,t1712,t1717,t1738,t1741,t1742,t1750,t1752,t1753,t1754,t1758,t1759,t1775,t1776,t18,t1861,t1874,t1879,t188,t1881,t189,t1896,t19,t1901,t1941,t1953,t1959,t1973,t1993,t1994,t2,t20,t201,t202,t2023,t2053,t2060,t2089,t2090,t2098,t2099,t21,t2117,t2120,t2122,t2123,t2125,t2137,t2139,t2140,t2142,t2145,t2146,t2147,t2149,t2150,t2151,t2152,t2153,t2154,t2155,t2159,t2162,t2164,t2165,t2166,t2167,t2168,t2169,t2174,t2183,t2187,t2193,t2194,t2195,t2199,t22,t2203,t2215,t2219,t2222,t2223,t2239,t2240,t2256,t2257,t2291,t2292,t2293,t2294,t2295,t2296,t2297,t2298,t2299,t23,t2301,t2302,t2303,t2304,t2306,t2307,t2308,t2310,t2311,t2317,t2320,t2323,t2324,t2325,t2326,t2329,t2337,t2338,t2339,t2341,t2342,t2343,t2344,t2352,t2353,t2355,t2358,t2359,t236,t2360,t2361,t2362,t2363,t2364,t2365,t2366,t2367,t2368,t2369,t237,t2370,t2371,t2378,t2379,t238,t2380,t2384,t2388,t2389,t2391,t2394,t2395,t2397,t2398,t2399,t24,t2400,t2401,t2402,t2403,t2404,t2405,t241,t2413,t2414,t2419,t2421,t2422,t2423,t2433,t2434,t2438,t244,t2447,t2448,t2449,t2450,t2459,t2460,t2461,t2471,t2472,t2492,t2493,t2494,t25,t2502,t2508,t2510,t2515,t2519,t2527,t2529,t2530,t2534,t2539,t2555,t2556,t2572,t2575,t2583,t2598,t26,t2605,t2606,t2612,t2613,t2618,t2619,t262,t2638,t264,t2651,t2652,t2664,t2670,t2671,t2673,t2674,t2675,t2676,t2678,t2680,t2681,t2683,t2684,t2685,t2686,t2687,t2689,t2690,t2692,t2693,t2694,t2695,t2696,t2697,t2698,t27,t2700,t2701,t2704,t2705,t2707,t2708,t2709,t2711,t2712,t2713,t2715,t2716,t2717,t2719,t2720,t2721,t2735,t2736,t2740,t2742,t2744,t2745,t2747,t2748,t2749,t2750,t2754,t2759,t2769,t2773,t2774,t2775,t2777,t2778,t2779,t2781,t2785,t2786,t2787,t2788,t2790,t2797,t28,t2801,t2803,t2804,t2807,t2808,t2813,t2814,t2820,t2823,t2828,t2831,t2834,t2835,t2838,t2850,t2851,t2927,t2937,t2941,t2942,t2945,t2946,t2947,t2950,t2951,t2953,t2954,t2955,t2956,t2957,t2963,t2964,t2965,t2966,t2969,t2970,t2975,t2978,t2979,t2984,t2985,t2986,t2987,t2990,t2991,t2993,t2994,t2998,t3,t30,t3003,t3004,t3006,t3008,t3009,t3010,t3015,t3016,t3017,t3018,t3019,t3022,t3027,t3029,t3030,t3031,t3036,t3043,t3044,t3045,t3047,t3049,t3050,t3051,t3054,t3055,t3056,t3057,t3063,t3064,t3065,t3066,t3067,t3068,t3072,t3073,t3074,t3075,t3076,t3077,t3078,t3079,t3080,t3081,t3082,t3083,t3085,t3086,t3087,t3088,t3096,t3097,t31,t3109,t3117,t3118,t3121,t3122,t3128,t3129,t313,t3130,t3131,t3132,t3133,t3134,t3135,t3139,t314,t3140,t3141,t3142,t3144,t3147,t3149,t3152,t3153,t3155,t3156,t3157,t3158,t3159,t3160,t3161,t3162,t3163,t3164,t3166,t3170,t3171,t3172,t3178,t3179,t3180,t3184,t3186,t3187,t3188,t3189,t3190,t3191,t3193,t3194,t3196,t3197,t3198,t3199,t32,t3200,t3201,t3204,t3206,t3209,t321,t3210,t3212,t3214,t3218,t322,t3220,t3223,t3224,t3225,t3226,t3227,t3228,t3229,t3230,t3231,t3232,t3235,t3238,t3244,t3245,t3246,t3247,t3248,t3249,t3250,t3252,t3253,t3254,t3256,t3258,t3259,t326,t3260,t3261,t3262,t3263,t3264,t3265,t3266,t3269,t3270,t3271,t3272,t3275,t3276,t3277,t3278,t328,t3280,t3281,t3282,t3283,t3284,t3286,t3287,t3288,t3289,t329,t3290,t3291,t3292,t3293,t3294,t3295,t3296,t3297,t3298,t33,t330,t3300,t3302,t3303,t3305,t3306,t3307,t3308,t3309,t331,t3310,t3313,t3316,t3318,t3319,t332,t3321,t3322,t3323,t3324,t3325,t3326,t3327,t3328,t333,t3330,t3331,t3333,t3334,t3335,t3336,t3337,t3338,t3340,t3341,t3342,t3343,t3344,t3345,t3346,t3347,t3348,t3349,t335,t3351,t3353,t3354,t3355,t3356,t3357,t3358,t3359,t3360,t3367,t3369,t3373,t3376,t3377,t3379,t338,t3382,t3383,t3384,t3385,t3386,t3388,t3389,t339,t3392,t3395,t3397,t3399,t34,t3400,t3401,t3404,t3405,t3408,t3409,t341,t3410,t3412,t3413,t3414,t3415,t3417,t3419,t3420,t3421,t3422,t3423,t3424,t3427,t3428,t3429,t343,t3430,t3432,t3433,t3434,t3435,t3436,t3437,t3438,t3440,t3441,t3442,t3443,t3444,t3445,t3446,t3447,t3449,t3450,t3451,t3452,t3453,t3455,t3456,t3457,t3458,t346,t3461,t3465,t3468,t3470,t3473,t3475,t3477,t3479,t3480,t3481,t3483,t3484,t3489,t3490,t3491,t3493,t3497,t3498,t35,t350,t3500,t3501,t3502,t3503,t3505,t3507,t3508,t351,t3510,t3511,t3512,t3513,t3515,t3516,t352,t3522,t3524,t3526,t3527,t3528,t3530,t3531,t3532,t3533,t3535,t3539,t354,t3541,t3542,t3543,t3544,t3546,t3547,t3549,t3550,t3553,t3554,t3556,t3557,t3558,t3559,t356,t3560,t3561,t3562,t3563,t3564,t3566,t3567,t3568,t3570,t3571,t3572,t3573,t3574,t3575,t3576,t3577,t3578,t3579,t358,t3580,t3581,t3582,t3584,t3585,t3586,t3587,t3588,t3589,t359,t3590,t3591,t3593,t3594,t3595,t3597,t3598,t36,t360,t3601,t3602,t3603,t3604,t3605,t3606,t3607,t3608,t3613,t3615,t3616,t3617,t3618,t3619,t362,t3620,t3621,t3622,t3623,t3624,t3625,t3626,t3627,t3628,t3629,t363,t3630,t3631,t3632,t3633,t3634,t3635,t3636,t3637,t3638,t364,t3640,t3642,t3643,t3644,t3645,t3647,t3648,t3649,t365,t3650,t3652,t3655,t3656,t3657,t3658,t3659,t366,t3660,t3661,t3662,t3664,t3665,t3667,t3669,t3670,t3672,t3673,t3674,t3676,t3677,t3678,t3679,t3680,t3681,t3682,t3683,t3684,t3685,t3686,t3687,t3688,t3689,t369,t3690,t3692,t3693,t3694,t3695,t3696,t3698,t3699,t370,t3700,t3701,t3703,t3705,t3706,t3708,t3709,t371,t3710,t3711,t3712,t3713,t3714,t3715,t3716,t3717,t3719,t372,t3720,t3721,t3722,t3723,t3724,t3725,t3727,t3729,t3732,t3734,t3735,t3736,t3737,t3738,t3739,t3740,t3741,t3744,t3745,t3746,t3748,t3749,t3751,t3753,t3755,t3756,t3757,t3758,t3759,t3760,t3762,t3763,t3764,t3765,t3766,t3767,t3768,t3769,t3770,t3771,t3772,t3774,t3775,t3776,t3778,t3779,t378,t3782,t3783,t3784,t3786,t3787,t3788,t3789,t3790,t3791,t3793,t3794,t3795,t3797,t3798,t3799,t38,t380,t3801,t3803,t3804,t3805,t3806,t3807,t3811,t3814,t3815,t3816,t3817,t3819,t382,t3821,t3822,t3823,t3824,t3825,t3826,t3827,t3828,t3830,t3833,t3834,t3836,t3837,t3838,t3839,t3841,t3842,t3843,t3844,t3845,t3847,t3849,t3850,t3852,t3853,t3854,t3855,t3856,t3858,t3859,t3860,t3861,t3862,t3863,t3864,t3865,t3866,t3867,t3868,t3869,t387,t3870,t3871,t3872,t3875,t3876,t3877,t3880,t3882,t3886,t3891,t3892,t3893,t3895,t3897,t3898,t39,t3901,t3904,t3906,t3908,t3910,t3916,t3917,t3918,t3920,t3921,t3922,t3925,t3926,t3927,t3928,t3933,t3934,t3936,t3937,t3939,t3940,t3941,t3942,t3943,t3945,t3946,t3949,t3950,t3951,t3953,t3954,t3955,t3956,t3957,t3958,t3959,t3960,t3962,t3964,t3965,t3966,t3968,t3970,t3971,t3974,t3976,t3977,t3978,t3980,t3981,t3982,t3983,t3984,t3985,t3990,t3991,t3992,t3997,t3998,t4,t4000,t4002,t4004,t4009,t4012,t4023,t4024,t4027,t4028,t4031,t4032,t4033,t4039,t4041,t4045,t4046,t4048,t4049,t4050,t4051,t4052,t4053,t4054,t4055,t4057,t4058,t4059,t4060,t4061,t4062,t4063,t4064,t4065,t4067,t4069,t4070,t4078,t4079,t4080,t4087,t4088,t410,t4101,t4106,t4108,t4109,t4111,t4113,t4122,t4125,t4127,t4131,t4133,t4134,t4135,t4136,t4140,t4143,t4149,t4150,t4151,t4152,t4154,t4155,t4157,t4160,t4161,t4162,t4163,t4166,t4168,t4170,t4173,t4175,t4177,t4178,t4179,t4182,t4183,t4184,t4186,t4188,t4189,t4190,t4196,t4197,t42,t4200,t4201,t4202,t4203,t4205,t4206,t4207,t4208,t4210,t4214,t4215,t4217,t4219,t4220,t4221,t4222,t4223,t4225,t4227,t4228,t4229,t4230,t4231,t4233,t4234,t4235,t4236,t4237,t4238,t4239,t4240,t4242,t4243,t4244,t4245,t4246,t4249,t4250,t4251,t4252,t4253,t4254,t4255,t4256,t4257,t4259,t4260,t4261,t4262,t4263,t4264,t4266,t4267,t4268,t4274,t4277,t4278,t4279,t4280,t4281,t4283,t4285,t4286,t4287,t4288,t429,t4290,t4291,t4292,t4294,t4295,t4296,t4298,t4299,t43,t4300,t4304,t4305,t4306,t4308,t4310,t4314,t4317,t4318,t4321,t4322,t4323,t4324,t4326,t4327,t4328,t4329,t4330,t4336,t4337,t4338,t4339,t4344,t4346,t4351,t4352,t4353,t4355,t4356,t4360,t4362,t4363,t4364,t4367,t4371,t4400,t4403,t4404,t4405,t4407,t4409,t4410,t4412,t4413,t4415,t4416,t4417,t4421,t4422,t4423,t4424,t4425,t4426,t4427,t4428,t4429,t4430,t4431,t4432,t4434,t4435,t4436,t4437,t4438,t4439,t4440,t4441,t4442,t4444,t4446,t4447,t4450,t4451,t4452,t4453,t4454,t4456,t4458,t4459,t4460,t4461,t4462,t4463,t4464,t4465,t4466,t4469,t4470,t4471,t4472,t4473,t4474,t4475,t4476,t4477,t4478,t4479,t4480,t4481,t4482,t4483,t4484,t4487,t4488,t4489,t4490,t4496,t4500,t4574,t4579,t4581,t4582,t4583,t4587,t4588,t4589,t4591,t4593,t4594,t4596,t4599,t46,t4602,t4604,t4606,t4607,t4608,t4610,t4611,t4612,t4614,t4615,t4617,t4620,t4621,t4624,t4640,t4641,t4642,t4644,t4645,t4647,t4649,t4650,t4652,t4655,t4658,t4661,t4663,t4664,t4665,t4666,t4667,t4669,t4673,t4676,t4678,t4679,t4680,t4682,t4683,t4684,t4685,t4686,t4688,t4689,t4693,t4695,t4697,t4698,t4699,t47,t4702,t4703,t4704,t4705,t4716,t4742,t4758,t4764,t4770,t4772,t4777,t4780,t4781,t4782,t4785,t4786,t4787,t4789,t4790,t4791,t4792,t4795,t4814,t4816,t4817,t4820,t4821,t4822,t4823,t4824,t4826,t4829,t4830,t4831,t4832,t4837,t4838,t4839,t4840,t4842,t4860,t4861,t4862,t4865,t4868,t4869,t4870,t4871,t4872,t4873,t4874,t4876,t4877,t4889,t4891,t4898,t4911,t4931,t4961,t4962,t4963,t4965,t4974,t4976,t4977,t4982,t4983,t4985,t4986,t4987,t4994,t4995,t4996,t4997,t4999,t5,t50,t5001,t5002,t5005,t5007,t5010,t5011,t5013,t5014,t5015,t5017,t5018,t5020,t5021,t5023,t5024,t5026,t5028,t5030,t5031,t5032,t5033,t5035,t5036,t5037,t5038,t5039,t5040,t5041,t5042,t5044,t5045,t5046,t5047,t5048,t5049,t5058,t5061,t5063,t5064,t5069,t5090,t5092,t5094,t5096,t5115,t5118,t5121,t5123,t5124,t5126,t5127,t5128,t5130,t5131,t5144,t5145,t5146,t5147,t5148,t5152,t5153,t5159,t5160,t5163,t5164,t5165,t5167,t5168,t5169,t5189,t5191,t5195,t5198,t5201,t5202,t5203,t5205,t5206,t5207,t5219,t5221,t5222,t5223,t5224,t5225,t5226,t5227,t5228,t5229,t5230,t5231,t5232,t5233,t5234,t5235,t5236,t5237,t5238,t5239,t5240,t5241,t5242,t5243,t5244,t5245,t5246,t5247,t5248,t5249,t5252,t5254,t5255,t5257,t5260,t5265,t5266,t5295,t5301,t5302,t5306,t5308,t5316,t5317,t5320,t5328,t5337,t5338,t5339,t5340,t5342,t5344,t5345,t5346,t5347,t5348,t5349,t5350,t5361,t5362,t5377,t5379,t5380,t5381,t5383,t5384,t5388,t5389,t5391,t5392,t5393,t5395,t5399,t5402,t5403,t5405,t5407,t5411,t5427,t5428,t5431,t5433,t5434,t5440,t5441,t5443,t5444,t5458,t5461,t5462,t5465,t5480,t5481,t5482,t5483,t5484,t5485,t5486,t5487,t5488,t5489,t5490,t5491,t5492,t5493,t5494,t5496,t5498,t5499,t5500,t5504,t5505,t5509,t5510,t5514,t5515,t5516,t5517,t5518,t5522,t5523,t5524,t5531,t5535,t5550,t5552,t5553,t5554,t5556,t5557,t5578,t5580,t56,t5603,t5620,t5626,t5627,t5631,t5670,t5671,t5674,t5675,t5678,t5679,t5681,t5682,t5694,t5695,t5700,t5701,t5702,t5703,t5720,t5722,t5723,t5750,t5791,t5792,t58,t5835,t5839,t5840,t5841,t5852,t5853,t5876,t5879,t5890,t5891,t59,t5930,t5932,t5941,t5951,t5953,t5954,t5977,t5994,t6,t60,t6004,t6017,t6075,t6183,t6184,t6185,t6199,t6206,t6207,t6209,t6219,t6221,t6247,t6253,t628,t6317,t6339,t6341,t635,t636,t6367,t638,t640,t641,t642,t643,t6484,t6485,t6486,t649,t6493,t6507,t6508,t6511,t6515,t654,t6543,t6544,t655,t656,t657,t659,t660,t663,t664,t665,t6658,t6663,t667,t668,t6689,t669,t6691,t6692,t67,t670,t672,t673,t674,t675,t676,t677,t678,t679,t68,t681,t6811,t6812,t6813,t682,t684,t685,t686,t687,t689,t6892,t6893,t691,t6916,t692,t693,t694,t7,t70,t7009,t702,t7032,t7041,t707,t708,t71,t710,t715,t716,t717,t718,t7204,t721,t722,t724,t725,t73,t736,t738,t740,t741,t749,t756,t76,t762,t768,t777,t792,t793,t801,t802,t808,t813,t819,t821,t850,t855,t874,t878,t89,t90,t91,t92,t941,t944,t948,t951,t97});
end
function tau_c = ft_10(ct)
t1005 = ct{1};
t1022 = ct{2};
t1089 = ct{3};
t1104 = ct{4};
t1105 = ct{5};
t1108 = ct{6};
t1115 = ct{7};
t1121 = ct{8};
t1158 = ct{9};
t1159 = ct{10};
t1190 = ct{11};
t1196 = ct{12};
t1205 = ct{13};
t1207 = ct{14};
t1208 = ct{15};
t1210 = ct{16};
t1212 = ct{17};
t1214 = ct{18};
t1217 = ct{19};
t1218 = ct{20};
t1219 = ct{21};
t1220 = ct{22};
t1221 = ct{23};
t123 = ct{24};
t1230 = ct{25};
t1235 = ct{26};
t1237 = ct{27};
t1238 = ct{28};
t1288 = ct{29};
t1289 = ct{30};
t1302 = ct{31};
t1303 = ct{32};
t1319 = ct{33};
t1320 = ct{34};
t1336 = ct{35};
t1348 = ct{36};
t1350 = ct{37};
t1351 = ct{38};
t1360 = ct{39};
t1369 = ct{40};
t1378 = ct{41};
t1396 = ct{42};
t14 = ct{43};
t140 = ct{44};
t1425 = ct{45};
t1435 = ct{46};
t1456 = ct{47};
t1477 = ct{48};
t1488 = ct{49};
t15 = ct{50};
t1513 = ct{51};
t1539 = ct{52};
t1544 = ct{53};
t1547 = ct{54};
t1548 = ct{55};
t1553 = ct{56};
t1554 = ct{57};
t1559 = ct{58};
t1564 = ct{59};
t1576 = ct{60};
t1577 = ct{61};
t1578 = ct{62};
t1579 = ct{63};
t1581 = ct{64};
t1584 = ct{65};
t1585 = ct{66};
t1586 = ct{67};
t1587 = ct{68};
t1591 = ct{69};
t1595 = ct{70};
t1596 = ct{71};
t1598 = ct{72};
t1599 = ct{73};
t16 = ct{74};
t1600 = ct{75};
t1601 = ct{76};
t1602 = ct{77};
t1604 = ct{78};
t1605 = ct{79};
t1606 = ct{80};
t1607 = ct{81};
t1608 = ct{82};
t1609 = ct{83};
t1612 = ct{84};
t1613 = ct{85};
t1614 = ct{86};
t1615 = ct{87};
t1616 = ct{88};
t1626 = ct{89};
t1627 = ct{90};
t1628 = ct{91};
t1629 = ct{92};
t1631 = ct{93};
t1637 = ct{94};
t1640 = ct{95};
t1641 = ct{96};
t1648 = ct{97};
t1649 = ct{98};
t1659 = ct{99};
t1660 = ct{100};
t1661 = ct{101};
t1666 = ct{102};
t1667 = ct{103};
t1683 = ct{104};
t1686 = ct{105};
t1690 = ct{106};
t1692 = ct{107};
t17 = ct{108};
t1700 = ct{109};
t1701 = ct{110};
t1703 = ct{111};
t1704 = ct{112};
t1705 = ct{113};
t1712 = ct{114};
t1717 = ct{115};
t1738 = ct{116};
t1741 = ct{117};
t1742 = ct{118};
t1750 = ct{119};
t1752 = ct{120};
t1753 = ct{121};
t1754 = ct{122};
t1758 = ct{123};
t1759 = ct{124};
t1775 = ct{125};
t1776 = ct{126};
t18 = ct{127};
t1861 = ct{128};
t1874 = ct{129};
t1879 = ct{130};
t188 = ct{131};
t1881 = ct{132};
t189 = ct{133};
t1896 = ct{134};
t19 = ct{135};
t1901 = ct{136};
t1941 = ct{137};
t1953 = ct{138};
t1959 = ct{139};
t1973 = ct{140};
t1993 = ct{141};
t1994 = ct{142};
t2 = ct{143};
t20 = ct{144};
t201 = ct{145};
t202 = ct{146};
t2023 = ct{147};
t2053 = ct{148};
t2060 = ct{149};
t2089 = ct{150};
t2090 = ct{151};
t2098 = ct{152};
t2099 = ct{153};
t21 = ct{154};
t2117 = ct{155};
t2120 = ct{156};
t2122 = ct{157};
t2123 = ct{158};
t2125 = ct{159};
t2137 = ct{160};
t2139 = ct{161};
t2140 = ct{162};
t2142 = ct{163};
t2145 = ct{164};
t2146 = ct{165};
t2147 = ct{166};
t2149 = ct{167};
t2150 = ct{168};
t2151 = ct{169};
t2152 = ct{170};
t2153 = ct{171};
t2154 = ct{172};
t2155 = ct{173};
t2159 = ct{174};
t2162 = ct{175};
t2164 = ct{176};
t2165 = ct{177};
t2166 = ct{178};
t2167 = ct{179};
t2168 = ct{180};
t2169 = ct{181};
t2174 = ct{182};
t2183 = ct{183};
t2187 = ct{184};
t2193 = ct{185};
t2194 = ct{186};
t2195 = ct{187};
t2199 = ct{188};
t22 = ct{189};
t2203 = ct{190};
t2215 = ct{191};
t2219 = ct{192};
t2222 = ct{193};
t2223 = ct{194};
t2239 = ct{195};
t2240 = ct{196};
t2256 = ct{197};
t2257 = ct{198};
t2291 = ct{199};
t2292 = ct{200};
t2293 = ct{201};
t2294 = ct{202};
t2295 = ct{203};
t2296 = ct{204};
t2297 = ct{205};
t2298 = ct{206};
t2299 = ct{207};
t23 = ct{208};
t2301 = ct{209};
t2302 = ct{210};
t2303 = ct{211};
t2304 = ct{212};
t2306 = ct{213};
t2307 = ct{214};
t2308 = ct{215};
t2310 = ct{216};
t2311 = ct{217};
t2317 = ct{218};
t2320 = ct{219};
t2323 = ct{220};
t2324 = ct{221};
t2325 = ct{222};
t2326 = ct{223};
t2329 = ct{224};
t2337 = ct{225};
t2338 = ct{226};
t2339 = ct{227};
t2341 = ct{228};
t2342 = ct{229};
t2343 = ct{230};
t2344 = ct{231};
t2352 = ct{232};
t2353 = ct{233};
t2355 = ct{234};
t2358 = ct{235};
t2359 = ct{236};
t236 = ct{237};
t2360 = ct{238};
t2361 = ct{239};
t2362 = ct{240};
t2363 = ct{241};
t2364 = ct{242};
t2365 = ct{243};
t2366 = ct{244};
t2367 = ct{245};
t2368 = ct{246};
t2369 = ct{247};
t237 = ct{248};
t2370 = ct{249};
t2371 = ct{250};
t2378 = ct{251};
t2379 = ct{252};
t238 = ct{253};
t2380 = ct{254};
t2384 = ct{255};
t2388 = ct{256};
t2389 = ct{257};
t2391 = ct{258};
t2394 = ct{259};
t2395 = ct{260};
t2397 = ct{261};
t2398 = ct{262};
t2399 = ct{263};
t24 = ct{264};
t2400 = ct{265};
t2401 = ct{266};
t2402 = ct{267};
t2403 = ct{268};
t2404 = ct{269};
t2405 = ct{270};
t241 = ct{271};
t2413 = ct{272};
t2414 = ct{273};
t2419 = ct{274};
t2421 = ct{275};
t2422 = ct{276};
t2423 = ct{277};
t2433 = ct{278};
t2434 = ct{279};
t2438 = ct{280};
t244 = ct{281};
t2447 = ct{282};
t2448 = ct{283};
t2449 = ct{284};
t2450 = ct{285};
t2459 = ct{286};
t2460 = ct{287};
t2461 = ct{288};
t2471 = ct{289};
t2472 = ct{290};
t2492 = ct{291};
t2493 = ct{292};
t2494 = ct{293};
t25 = ct{294};
t2502 = ct{295};
t2508 = ct{296};
t2510 = ct{297};
t2515 = ct{298};
t2519 = ct{299};
t2527 = ct{300};
t2529 = ct{301};
t2530 = ct{302};
t2534 = ct{303};
t2539 = ct{304};
t2555 = ct{305};
t2556 = ct{306};
t2572 = ct{307};
t2575 = ct{308};
t2583 = ct{309};
t2598 = ct{310};
t26 = ct{311};
t2605 = ct{312};
t2606 = ct{313};
t2612 = ct{314};
t2613 = ct{315};
t2618 = ct{316};
t2619 = ct{317};
t262 = ct{318};
t2638 = ct{319};
t264 = ct{320};
t2651 = ct{321};
t2652 = ct{322};
t2664 = ct{323};
t2670 = ct{324};
t2671 = ct{325};
t2673 = ct{326};
t2674 = ct{327};
t2675 = ct{328};
t2676 = ct{329};
t2678 = ct{330};
t2680 = ct{331};
t2681 = ct{332};
t2683 = ct{333};
t2684 = ct{334};
t2685 = ct{335};
t2686 = ct{336};
t2687 = ct{337};
t2689 = ct{338};
t2690 = ct{339};
t2692 = ct{340};
t2693 = ct{341};
t2694 = ct{342};
t2695 = ct{343};
t2696 = ct{344};
t2697 = ct{345};
t2698 = ct{346};
t27 = ct{347};
t2700 = ct{348};
t2701 = ct{349};
t2704 = ct{350};
t2705 = ct{351};
t2707 = ct{352};
t2708 = ct{353};
t2709 = ct{354};
t2711 = ct{355};
t2712 = ct{356};
t2713 = ct{357};
t2715 = ct{358};
t2716 = ct{359};
t2717 = ct{360};
t2719 = ct{361};
t2720 = ct{362};
t2721 = ct{363};
t2735 = ct{364};
t2736 = ct{365};
t2740 = ct{366};
t2742 = ct{367};
t2744 = ct{368};
t2745 = ct{369};
t2747 = ct{370};
t2748 = ct{371};
t2749 = ct{372};
t2750 = ct{373};
t2754 = ct{374};
t2759 = ct{375};
t2769 = ct{376};
t2773 = ct{377};
t2774 = ct{378};
t2775 = ct{379};
t2777 = ct{380};
t2778 = ct{381};
t2779 = ct{382};
t2781 = ct{383};
t2785 = ct{384};
t2786 = ct{385};
t2787 = ct{386};
t2788 = ct{387};
t2790 = ct{388};
t2797 = ct{389};
t28 = ct{390};
t2801 = ct{391};
t2803 = ct{392};
t2804 = ct{393};
t2807 = ct{394};
t2808 = ct{395};
t2813 = ct{396};
t2814 = ct{397};
t2820 = ct{398};
t2823 = ct{399};
t2828 = ct{400};
t2831 = ct{401};
t2834 = ct{402};
t2835 = ct{403};
t2838 = ct{404};
t2850 = ct{405};
t2851 = ct{406};
t2927 = ct{407};
t2937 = ct{408};
t2941 = ct{409};
t2942 = ct{410};
t2945 = ct{411};
t2946 = ct{412};
t2947 = ct{413};
t2950 = ct{414};
t2951 = ct{415};
t2953 = ct{416};
t2954 = ct{417};
t2955 = ct{418};
t2956 = ct{419};
t2957 = ct{420};
t2963 = ct{421};
t2964 = ct{422};
t2965 = ct{423};
t2966 = ct{424};
t2969 = ct{425};
t2970 = ct{426};
t2975 = ct{427};
t2978 = ct{428};
t2979 = ct{429};
t2984 = ct{430};
t2985 = ct{431};
t2986 = ct{432};
t2987 = ct{433};
t2990 = ct{434};
t2991 = ct{435};
t2993 = ct{436};
t2994 = ct{437};
t2998 = ct{438};
t3 = ct{439};
t30 = ct{440};
t3003 = ct{441};
t3004 = ct{442};
t3006 = ct{443};
t3008 = ct{444};
t3009 = ct{445};
t3010 = ct{446};
t3015 = ct{447};
t3016 = ct{448};
t3017 = ct{449};
t3018 = ct{450};
t3019 = ct{451};
t3022 = ct{452};
t3027 = ct{453};
t3029 = ct{454};
t3030 = ct{455};
t3031 = ct{456};
t3036 = ct{457};
t3043 = ct{458};
t3044 = ct{459};
t3045 = ct{460};
t3047 = ct{461};
t3049 = ct{462};
t3050 = ct{463};
t3051 = ct{464};
t3054 = ct{465};
t3055 = ct{466};
t3056 = ct{467};
t3057 = ct{468};
t3063 = ct{469};
t3064 = ct{470};
t3065 = ct{471};
t3066 = ct{472};
t3067 = ct{473};
t3068 = ct{474};
t3072 = ct{475};
t3073 = ct{476};
t3074 = ct{477};
t3075 = ct{478};
t3076 = ct{479};
t3077 = ct{480};
t3078 = ct{481};
t3079 = ct{482};
t3080 = ct{483};
t3081 = ct{484};
t3082 = ct{485};
t3083 = ct{486};
t3085 = ct{487};
t3086 = ct{488};
t3087 = ct{489};
t3088 = ct{490};
t3096 = ct{491};
t3097 = ct{492};
t31 = ct{493};
t3109 = ct{494};
t3117 = ct{495};
t3118 = ct{496};
t3121 = ct{497};
t3122 = ct{498};
t3128 = ct{499};
t3129 = ct{500};
t313 = ct{501};
t3130 = ct{502};
t3131 = ct{503};
t3132 = ct{504};
t3133 = ct{505};
t3134 = ct{506};
t3135 = ct{507};
t3139 = ct{508};
t314 = ct{509};
t3140 = ct{510};
t3141 = ct{511};
t3142 = ct{512};
t3144 = ct{513};
t3147 = ct{514};
t3149 = ct{515};
t3152 = ct{516};
t3153 = ct{517};
t3155 = ct{518};
t3156 = ct{519};
t3157 = ct{520};
t3158 = ct{521};
t3159 = ct{522};
t3160 = ct{523};
t3161 = ct{524};
t3162 = ct{525};
t3163 = ct{526};
t3164 = ct{527};
t3166 = ct{528};
t3170 = ct{529};
t3171 = ct{530};
t3172 = ct{531};
t3178 = ct{532};
t3179 = ct{533};
t3180 = ct{534};
t3184 = ct{535};
t3186 = ct{536};
t3187 = ct{537};
t3188 = ct{538};
t3189 = ct{539};
t3190 = ct{540};
t3191 = ct{541};
t3193 = ct{542};
t3194 = ct{543};
t3196 = ct{544};
t3197 = ct{545};
t3198 = ct{546};
t3199 = ct{547};
t32 = ct{548};
t3200 = ct{549};
t3201 = ct{550};
t3204 = ct{551};
t3206 = ct{552};
t3209 = ct{553};
t321 = ct{554};
t3210 = ct{555};
t3212 = ct{556};
t3214 = ct{557};
t3218 = ct{558};
t322 = ct{559};
t3220 = ct{560};
t3223 = ct{561};
t3224 = ct{562};
t3225 = ct{563};
t3226 = ct{564};
t3227 = ct{565};
t3228 = ct{566};
t3229 = ct{567};
t3230 = ct{568};
t3231 = ct{569};
t3232 = ct{570};
t3235 = ct{571};
t3238 = ct{572};
t3244 = ct{573};
t3245 = ct{574};
t3246 = ct{575};
t3247 = ct{576};
t3248 = ct{577};
t3249 = ct{578};
t3250 = ct{579};
t3252 = ct{580};
t3253 = ct{581};
t3254 = ct{582};
t3256 = ct{583};
t3258 = ct{584};
t3259 = ct{585};
t326 = ct{586};
t3260 = ct{587};
t3261 = ct{588};
t3262 = ct{589};
t3263 = ct{590};
t3264 = ct{591};
t3265 = ct{592};
t3266 = ct{593};
t3269 = ct{594};
t3270 = ct{595};
t3271 = ct{596};
t3272 = ct{597};
t3275 = ct{598};
t3276 = ct{599};
t3277 = ct{600};
t3278 = ct{601};
t328 = ct{602};
t3280 = ct{603};
t3281 = ct{604};
t3282 = ct{605};
t3283 = ct{606};
t3284 = ct{607};
t3286 = ct{608};
t3287 = ct{609};
t3288 = ct{610};
t3289 = ct{611};
t329 = ct{612};
t3290 = ct{613};
t3291 = ct{614};
t3292 = ct{615};
t3293 = ct{616};
t3294 = ct{617};
t3295 = ct{618};
t3296 = ct{619};
t3297 = ct{620};
t3298 = ct{621};
t33 = ct{622};
t330 = ct{623};
t3300 = ct{624};
t3302 = ct{625};
t3303 = ct{626};
t3305 = ct{627};
t3306 = ct{628};
t3307 = ct{629};
t3308 = ct{630};
t3309 = ct{631};
t331 = ct{632};
t3310 = ct{633};
t3313 = ct{634};
t3316 = ct{635};
t3318 = ct{636};
t3319 = ct{637};
t332 = ct{638};
t3321 = ct{639};
t3322 = ct{640};
t3323 = ct{641};
t3324 = ct{642};
t3325 = ct{643};
t3326 = ct{644};
t3327 = ct{645};
t3328 = ct{646};
t333 = ct{647};
t3330 = ct{648};
t3331 = ct{649};
t3333 = ct{650};
t3334 = ct{651};
t3335 = ct{652};
t3336 = ct{653};
t3337 = ct{654};
t3338 = ct{655};
t3340 = ct{656};
t3341 = ct{657};
t3342 = ct{658};
t3343 = ct{659};
t3344 = ct{660};
t3345 = ct{661};
t3346 = ct{662};
t3347 = ct{663};
t3348 = ct{664};
t3349 = ct{665};
t335 = ct{666};
t3351 = ct{667};
t3353 = ct{668};
t3354 = ct{669};
t3355 = ct{670};
t3356 = ct{671};
t3357 = ct{672};
t3358 = ct{673};
t3359 = ct{674};
t3360 = ct{675};
t3367 = ct{676};
t3369 = ct{677};
t3373 = ct{678};
t3376 = ct{679};
t3377 = ct{680};
t3379 = ct{681};
t338 = ct{682};
t3382 = ct{683};
t3383 = ct{684};
t3384 = ct{685};
t3385 = ct{686};
t3386 = ct{687};
t3388 = ct{688};
t3389 = ct{689};
t339 = ct{690};
t3392 = ct{691};
t3395 = ct{692};
t3397 = ct{693};
t3399 = ct{694};
t34 = ct{695};
t3400 = ct{696};
t3401 = ct{697};
t3404 = ct{698};
t3405 = ct{699};
t3408 = ct{700};
t3409 = ct{701};
t341 = ct{702};
t3410 = ct{703};
t3412 = ct{704};
t3413 = ct{705};
t3414 = ct{706};
t3415 = ct{707};
t3417 = ct{708};
t3419 = ct{709};
t3420 = ct{710};
t3421 = ct{711};
t3422 = ct{712};
t3423 = ct{713};
t3424 = ct{714};
t3427 = ct{715};
t3428 = ct{716};
t3429 = ct{717};
t343 = ct{718};
t3430 = ct{719};
t3432 = ct{720};
t3433 = ct{721};
t3434 = ct{722};
t3435 = ct{723};
t3436 = ct{724};
t3437 = ct{725};
t3438 = ct{726};
t3440 = ct{727};
t3441 = ct{728};
t3442 = ct{729};
t3443 = ct{730};
t3444 = ct{731};
t3445 = ct{732};
t3446 = ct{733};
t3447 = ct{734};
t3449 = ct{735};
t3450 = ct{736};
t3451 = ct{737};
t3452 = ct{738};
t3453 = ct{739};
t3455 = ct{740};
t3456 = ct{741};
t3457 = ct{742};
t3458 = ct{743};
t346 = ct{744};
t3461 = ct{745};
t3465 = ct{746};
t3468 = ct{747};
t3470 = ct{748};
t3473 = ct{749};
t3475 = ct{750};
t3477 = ct{751};
t3479 = ct{752};
t3480 = ct{753};
t3481 = ct{754};
t3483 = ct{755};
t3484 = ct{756};
t3489 = ct{757};
t3490 = ct{758};
t3491 = ct{759};
t3493 = ct{760};
t3497 = ct{761};
t3498 = ct{762};
t35 = ct{763};
t350 = ct{764};
t3500 = ct{765};
t3501 = ct{766};
t3502 = ct{767};
t3503 = ct{768};
t3505 = ct{769};
t3507 = ct{770};
t3508 = ct{771};
t351 = ct{772};
t3510 = ct{773};
t3511 = ct{774};
t3512 = ct{775};
t3513 = ct{776};
t3515 = ct{777};
t3516 = ct{778};
t352 = ct{779};
t3522 = ct{780};
t3524 = ct{781};
t3526 = ct{782};
t3527 = ct{783};
t3528 = ct{784};
t3530 = ct{785};
t3531 = ct{786};
t3532 = ct{787};
t3533 = ct{788};
t3535 = ct{789};
t3539 = ct{790};
t354 = ct{791};
t3541 = ct{792};
t3542 = ct{793};
t3543 = ct{794};
t3544 = ct{795};
t3546 = ct{796};
t3547 = ct{797};
t3549 = ct{798};
t3550 = ct{799};
t3553 = ct{800};
t3554 = ct{801};
t3556 = ct{802};
t3557 = ct{803};
t3558 = ct{804};
t3559 = ct{805};
t356 = ct{806};
t3560 = ct{807};
t3561 = ct{808};
t3562 = ct{809};
t3563 = ct{810};
t3564 = ct{811};
t3566 = ct{812};
t3567 = ct{813};
t3568 = ct{814};
t3570 = ct{815};
t3571 = ct{816};
t3572 = ct{817};
t3573 = ct{818};
t3574 = ct{819};
t3575 = ct{820};
t3576 = ct{821};
t3577 = ct{822};
t3578 = ct{823};
t3579 = ct{824};
t358 = ct{825};
t3580 = ct{826};
t3581 = ct{827};
t3582 = ct{828};
t3584 = ct{829};
t3585 = ct{830};
t3586 = ct{831};
t3587 = ct{832};
t3588 = ct{833};
t3589 = ct{834};
t359 = ct{835};
t3590 = ct{836};
t3591 = ct{837};
t3593 = ct{838};
t3594 = ct{839};
t3595 = ct{840};
t3597 = ct{841};
t3598 = ct{842};
t36 = ct{843};
t360 = ct{844};
t3601 = ct{845};
t3602 = ct{846};
t3603 = ct{847};
t3604 = ct{848};
t3605 = ct{849};
t3606 = ct{850};
t3607 = ct{851};
t3608 = ct{852};
t3613 = ct{853};
t3615 = ct{854};
t3616 = ct{855};
t3617 = ct{856};
t3618 = ct{857};
t3619 = ct{858};
t362 = ct{859};
t3620 = ct{860};
t3621 = ct{861};
t3622 = ct{862};
t3623 = ct{863};
t3624 = ct{864};
t3625 = ct{865};
t3626 = ct{866};
t3627 = ct{867};
t3628 = ct{868};
t3629 = ct{869};
t363 = ct{870};
t3630 = ct{871};
t3631 = ct{872};
t3632 = ct{873};
t3633 = ct{874};
t3634 = ct{875};
t3635 = ct{876};
t3636 = ct{877};
t3637 = ct{878};
t3638 = ct{879};
t364 = ct{880};
t3640 = ct{881};
t3642 = ct{882};
t3643 = ct{883};
t3644 = ct{884};
t3645 = ct{885};
t3647 = ct{886};
t3648 = ct{887};
t3649 = ct{888};
t365 = ct{889};
t3650 = ct{890};
t3652 = ct{891};
t3655 = ct{892};
t3656 = ct{893};
t3657 = ct{894};
t3658 = ct{895};
t3659 = ct{896};
t366 = ct{897};
t3660 = ct{898};
t3661 = ct{899};
t3662 = ct{900};
t3664 = ct{901};
t3665 = ct{902};
t3667 = ct{903};
t3669 = ct{904};
t3670 = ct{905};
t3672 = ct{906};
t3673 = ct{907};
t3674 = ct{908};
t3676 = ct{909};
t3677 = ct{910};
t3678 = ct{911};
t3679 = ct{912};
t3680 = ct{913};
t3681 = ct{914};
t3682 = ct{915};
t3683 = ct{916};
t3684 = ct{917};
t3685 = ct{918};
t3686 = ct{919};
t3687 = ct{920};
t3688 = ct{921};
t3689 = ct{922};
t369 = ct{923};
t3690 = ct{924};
t3692 = ct{925};
t3693 = ct{926};
t3694 = ct{927};
t3695 = ct{928};
t3696 = ct{929};
t3698 = ct{930};
t3699 = ct{931};
t370 = ct{932};
t3700 = ct{933};
t3701 = ct{934};
t3703 = ct{935};
t3705 = ct{936};
t3706 = ct{937};
t3708 = ct{938};
t3709 = ct{939};
t371 = ct{940};
t3710 = ct{941};
t3711 = ct{942};
t3712 = ct{943};
t3713 = ct{944};
t3714 = ct{945};
t3715 = ct{946};
t3716 = ct{947};
t3717 = ct{948};
t3719 = ct{949};
t372 = ct{950};
t3720 = ct{951};
t3721 = ct{952};
t3722 = ct{953};
t3723 = ct{954};
t3724 = ct{955};
t3725 = ct{956};
t3727 = ct{957};
t3729 = ct{958};
t3732 = ct{959};
t3734 = ct{960};
t3735 = ct{961};
t3736 = ct{962};
t3737 = ct{963};
t3738 = ct{964};
t3739 = ct{965};
t3740 = ct{966};
t3741 = ct{967};
t3744 = ct{968};
t3745 = ct{969};
t3746 = ct{970};
t3748 = ct{971};
t3749 = ct{972};
t3751 = ct{973};
t3753 = ct{974};
t3755 = ct{975};
t3756 = ct{976};
t3757 = ct{977};
t3758 = ct{978};
t3759 = ct{979};
t3760 = ct{980};
t3762 = ct{981};
t3763 = ct{982};
t3764 = ct{983};
t3765 = ct{984};
t3766 = ct{985};
t3767 = ct{986};
t3768 = ct{987};
t3769 = ct{988};
t3770 = ct{989};
t3771 = ct{990};
t3772 = ct{991};
t3774 = ct{992};
t3775 = ct{993};
t3776 = ct{994};
t3778 = ct{995};
t3779 = ct{996};
t378 = ct{997};
t3782 = ct{998};
t3783 = ct{999};
t3784 = ct{1000};
t3786 = ct{1001};
t3787 = ct{1002};
t3788 = ct{1003};
t3789 = ct{1004};
t3790 = ct{1005};
t3791 = ct{1006};
t3793 = ct{1007};
t3794 = ct{1008};
t3795 = ct{1009};
t3797 = ct{1010};
t3798 = ct{1011};
t3799 = ct{1012};
t38 = ct{1013};
t380 = ct{1014};
t3801 = ct{1015};
t3803 = ct{1016};
t3804 = ct{1017};
t3805 = ct{1018};
t3806 = ct{1019};
t3807 = ct{1020};
t3811 = ct{1021};
t3814 = ct{1022};
t3815 = ct{1023};
t3816 = ct{1024};
t3817 = ct{1025};
t3819 = ct{1026};
t382 = ct{1027};
t3821 = ct{1028};
t3822 = ct{1029};
t3823 = ct{1030};
t3824 = ct{1031};
t3825 = ct{1032};
t3826 = ct{1033};
t3827 = ct{1034};
t3828 = ct{1035};
t3830 = ct{1036};
t3833 = ct{1037};
t3834 = ct{1038};
t3836 = ct{1039};
t3837 = ct{1040};
t3838 = ct{1041};
t3839 = ct{1042};
t3841 = ct{1043};
t3842 = ct{1044};
t3843 = ct{1045};
t3844 = ct{1046};
t3845 = ct{1047};
t3847 = ct{1048};
t3849 = ct{1049};
t3850 = ct{1050};
t3852 = ct{1051};
t3853 = ct{1052};
t3854 = ct{1053};
t3855 = ct{1054};
t3856 = ct{1055};
t3858 = ct{1056};
t3859 = ct{1057};
t3860 = ct{1058};
t3861 = ct{1059};
t3862 = ct{1060};
t3863 = ct{1061};
t3864 = ct{1062};
t3865 = ct{1063};
t3866 = ct{1064};
t3867 = ct{1065};
t3868 = ct{1066};
t3869 = ct{1067};
t387 = ct{1068};
t3870 = ct{1069};
t3871 = ct{1070};
t3872 = ct{1071};
t3875 = ct{1072};
t3876 = ct{1073};
t3877 = ct{1074};
t3880 = ct{1075};
t3882 = ct{1076};
t3886 = ct{1077};
t3891 = ct{1078};
t3892 = ct{1079};
t3893 = ct{1080};
t3895 = ct{1081};
t3897 = ct{1082};
t3898 = ct{1083};
t39 = ct{1084};
t3901 = ct{1085};
t3904 = ct{1086};
t3906 = ct{1087};
t3908 = ct{1088};
t3910 = ct{1089};
t3916 = ct{1090};
t3917 = ct{1091};
t3918 = ct{1092};
t3920 = ct{1093};
t3921 = ct{1094};
t3922 = ct{1095};
t3925 = ct{1096};
t3926 = ct{1097};
t3927 = ct{1098};
t3928 = ct{1099};
t3933 = ct{1100};
t3934 = ct{1101};
t3936 = ct{1102};
t3937 = ct{1103};
t3939 = ct{1104};
t3940 = ct{1105};
t3941 = ct{1106};
t3942 = ct{1107};
t3943 = ct{1108};
t3945 = ct{1109};
t3946 = ct{1110};
t3949 = ct{1111};
t3950 = ct{1112};
t3951 = ct{1113};
t3953 = ct{1114};
t3954 = ct{1115};
t3955 = ct{1116};
t3956 = ct{1117};
t3957 = ct{1118};
t3958 = ct{1119};
t3959 = ct{1120};
t3960 = ct{1121};
t3962 = ct{1122};
t3964 = ct{1123};
t3965 = ct{1124};
t3966 = ct{1125};
t3968 = ct{1126};
t3970 = ct{1127};
t3971 = ct{1128};
t3974 = ct{1129};
t3976 = ct{1130};
t3977 = ct{1131};
t3978 = ct{1132};
t3980 = ct{1133};
t3981 = ct{1134};
t3982 = ct{1135};
t3983 = ct{1136};
t3984 = ct{1137};
t3985 = ct{1138};
t3990 = ct{1139};
t3991 = ct{1140};
t3992 = ct{1141};
t3997 = ct{1142};
t3998 = ct{1143};
t4 = ct{1144};
t4000 = ct{1145};
t4002 = ct{1146};
t4004 = ct{1147};
t4009 = ct{1148};
t4012 = ct{1149};
t4023 = ct{1150};
t4024 = ct{1151};
t4027 = ct{1152};
t4028 = ct{1153};
t4031 = ct{1154};
t4032 = ct{1155};
t4033 = ct{1156};
t4039 = ct{1157};
t4041 = ct{1158};
t4045 = ct{1159};
t4046 = ct{1160};
t4048 = ct{1161};
t4049 = ct{1162};
t4050 = ct{1163};
t4051 = ct{1164};
t4052 = ct{1165};
t4053 = ct{1166};
t4054 = ct{1167};
t4055 = ct{1168};
t4057 = ct{1169};
t4058 = ct{1170};
t4059 = ct{1171};
t4060 = ct{1172};
t4061 = ct{1173};
t4062 = ct{1174};
t4063 = ct{1175};
t4064 = ct{1176};
t4065 = ct{1177};
t4067 = ct{1178};
t4069 = ct{1179};
t4070 = ct{1180};
t4078 = ct{1181};
t4079 = ct{1182};
t4080 = ct{1183};
t4087 = ct{1184};
t4088 = ct{1185};
t410 = ct{1186};
t4101 = ct{1187};
t4106 = ct{1188};
t4108 = ct{1189};
t4109 = ct{1190};
t4111 = ct{1191};
t4113 = ct{1192};
t4122 = ct{1193};
t4125 = ct{1194};
t4127 = ct{1195};
t4131 = ct{1196};
t4133 = ct{1197};
t4134 = ct{1198};
t4135 = ct{1199};
t4136 = ct{1200};
t4140 = ct{1201};
t4143 = ct{1202};
t4149 = ct{1203};
t4150 = ct{1204};
t4151 = ct{1205};
t4152 = ct{1206};
t4154 = ct{1207};
t4155 = ct{1208};
t4157 = ct{1209};
t4160 = ct{1210};
t4161 = ct{1211};
t4162 = ct{1212};
t4163 = ct{1213};
t4166 = ct{1214};
t4168 = ct{1215};
t4170 = ct{1216};
t4173 = ct{1217};
t4175 = ct{1218};
t4177 = ct{1219};
t4178 = ct{1220};
t4179 = ct{1221};
t4182 = ct{1222};
t4183 = ct{1223};
t4184 = ct{1224};
t4186 = ct{1225};
t4188 = ct{1226};
t4189 = ct{1227};
t4190 = ct{1228};
t4196 = ct{1229};
t4197 = ct{1230};
t42 = ct{1231};
t4200 = ct{1232};
t4201 = ct{1233};
t4202 = ct{1234};
t4203 = ct{1235};
t4205 = ct{1236};
t4206 = ct{1237};
t4207 = ct{1238};
t4208 = ct{1239};
t4210 = ct{1240};
t4214 = ct{1241};
t4215 = ct{1242};
t4217 = ct{1243};
t4219 = ct{1244};
t4220 = ct{1245};
t4221 = ct{1246};
t4222 = ct{1247};
t4223 = ct{1248};
t4225 = ct{1249};
t4227 = ct{1250};
t4228 = ct{1251};
t4229 = ct{1252};
t4230 = ct{1253};
t4231 = ct{1254};
t4233 = ct{1255};
t4234 = ct{1256};
t4235 = ct{1257};
t4236 = ct{1258};
t4237 = ct{1259};
t4238 = ct{1260};
t4239 = ct{1261};
t4240 = ct{1262};
t4242 = ct{1263};
t4243 = ct{1264};
t4244 = ct{1265};
t4245 = ct{1266};
t4246 = ct{1267};
t4249 = ct{1268};
t4250 = ct{1269};
t4251 = ct{1270};
t4252 = ct{1271};
t4253 = ct{1272};
t4254 = ct{1273};
t4255 = ct{1274};
t4256 = ct{1275};
t4257 = ct{1276};
t4259 = ct{1277};
t4260 = ct{1278};
t4261 = ct{1279};
t4262 = ct{1280};
t4263 = ct{1281};
t4264 = ct{1282};
t4266 = ct{1283};
t4267 = ct{1284};
t4268 = ct{1285};
t4274 = ct{1286};
t4277 = ct{1287};
t4278 = ct{1288};
t4279 = ct{1289};
t4280 = ct{1290};
t4281 = ct{1291};
t4283 = ct{1292};
t4285 = ct{1293};
t4286 = ct{1294};
t4287 = ct{1295};
t4288 = ct{1296};
t429 = ct{1297};
t4290 = ct{1298};
t4291 = ct{1299};
t4292 = ct{1300};
t4294 = ct{1301};
t4295 = ct{1302};
t4296 = ct{1303};
t4298 = ct{1304};
t4299 = ct{1305};
t43 = ct{1306};
t4300 = ct{1307};
t4304 = ct{1308};
t4305 = ct{1309};
t4306 = ct{1310};
t4308 = ct{1311};
t4310 = ct{1312};
t4314 = ct{1313};
t4317 = ct{1314};
t4318 = ct{1315};
t4321 = ct{1316};
t4322 = ct{1317};
t4323 = ct{1318};
t4324 = ct{1319};
t4326 = ct{1320};
t4327 = ct{1321};
t4328 = ct{1322};
t4329 = ct{1323};
t4330 = ct{1324};
t4336 = ct{1325};
t4337 = ct{1326};
t4338 = ct{1327};
t4339 = ct{1328};
t4344 = ct{1329};
t4346 = ct{1330};
t4351 = ct{1331};
t4352 = ct{1332};
t4353 = ct{1333};
t4355 = ct{1334};
t4356 = ct{1335};
t4360 = ct{1336};
t4362 = ct{1337};
t4363 = ct{1338};
t4364 = ct{1339};
t4367 = ct{1340};
t4371 = ct{1341};
t4400 = ct{1342};
t4403 = ct{1343};
t4404 = ct{1344};
t4405 = ct{1345};
t4407 = ct{1346};
t4409 = ct{1347};
t4410 = ct{1348};
t4412 = ct{1349};
t4413 = ct{1350};
t4415 = ct{1351};
t4416 = ct{1352};
t4417 = ct{1353};
t4421 = ct{1354};
t4422 = ct{1355};
t4423 = ct{1356};
t4424 = ct{1357};
t4425 = ct{1358};
t4426 = ct{1359};
t4427 = ct{1360};
t4428 = ct{1361};
t4429 = ct{1362};
t4430 = ct{1363};
t4431 = ct{1364};
t4432 = ct{1365};
t4434 = ct{1366};
t4435 = ct{1367};
t4436 = ct{1368};
t4437 = ct{1369};
t4438 = ct{1370};
t4439 = ct{1371};
t4440 = ct{1372};
t4441 = ct{1373};
t4442 = ct{1374};
t4444 = ct{1375};
t4446 = ct{1376};
t4447 = ct{1377};
t4450 = ct{1378};
t4451 = ct{1379};
t4452 = ct{1380};
t4453 = ct{1381};
t4454 = ct{1382};
t4456 = ct{1383};
t4458 = ct{1384};
t4459 = ct{1385};
t4460 = ct{1386};
t4461 = ct{1387};
t4462 = ct{1388};
t4463 = ct{1389};
t4464 = ct{1390};
t4465 = ct{1391};
t4466 = ct{1392};
t4469 = ct{1393};
t4470 = ct{1394};
t4471 = ct{1395};
t4472 = ct{1396};
t4473 = ct{1397};
t4474 = ct{1398};
t4475 = ct{1399};
t4476 = ct{1400};
t4477 = ct{1401};
t4478 = ct{1402};
t4479 = ct{1403};
t4480 = ct{1404};
t4481 = ct{1405};
t4482 = ct{1406};
t4483 = ct{1407};
t4484 = ct{1408};
t4487 = ct{1409};
t4488 = ct{1410};
t4489 = ct{1411};
t4490 = ct{1412};
t4496 = ct{1413};
t4500 = ct{1414};
t4574 = ct{1415};
t4579 = ct{1416};
t4581 = ct{1417};
t4582 = ct{1418};
t4583 = ct{1419};
t4587 = ct{1420};
t4588 = ct{1421};
t4589 = ct{1422};
t4591 = ct{1423};
t4593 = ct{1424};
t4594 = ct{1425};
t4596 = ct{1426};
t4599 = ct{1427};
t46 = ct{1428};
t4602 = ct{1429};
t4604 = ct{1430};
t4606 = ct{1431};
t4607 = ct{1432};
t4608 = ct{1433};
t4610 = ct{1434};
t4611 = ct{1435};
t4612 = ct{1436};
t4614 = ct{1437};
t4615 = ct{1438};
t4617 = ct{1439};
t4620 = ct{1440};
t4621 = ct{1441};
t4624 = ct{1442};
t4640 = ct{1443};
t4641 = ct{1444};
t4642 = ct{1445};
t4644 = ct{1446};
t4645 = ct{1447};
t4647 = ct{1448};
t4649 = ct{1449};
t4650 = ct{1450};
t4652 = ct{1451};
t4655 = ct{1452};
t4658 = ct{1453};
t4661 = ct{1454};
t4663 = ct{1455};
t4664 = ct{1456};
t4665 = ct{1457};
t4666 = ct{1458};
t4667 = ct{1459};
t4669 = ct{1460};
t4673 = ct{1461};
t4676 = ct{1462};
t4678 = ct{1463};
t4679 = ct{1464};
t4680 = ct{1465};
t4682 = ct{1466};
t4683 = ct{1467};
t4684 = ct{1468};
t4685 = ct{1469};
t4686 = ct{1470};
t4688 = ct{1471};
t4689 = ct{1472};
t4693 = ct{1473};
t4695 = ct{1474};
t4697 = ct{1475};
t4698 = ct{1476};
t4699 = ct{1477};
t47 = ct{1478};
t4702 = ct{1479};
t4703 = ct{1480};
t4704 = ct{1481};
t4705 = ct{1482};
t4716 = ct{1483};
t4742 = ct{1484};
t4758 = ct{1485};
t4764 = ct{1486};
t4770 = ct{1487};
t4772 = ct{1488};
t4777 = ct{1489};
t4780 = ct{1490};
t4781 = ct{1491};
t4782 = ct{1492};
t4785 = ct{1493};
t4786 = ct{1494};
t4787 = ct{1495};
t4789 = ct{1496};
t4790 = ct{1497};
t4791 = ct{1498};
t4792 = ct{1499};
t4795 = ct{1500};
t4814 = ct{1501};
t4816 = ct{1502};
t4817 = ct{1503};
t4820 = ct{1504};
t4821 = ct{1505};
t4822 = ct{1506};
t4823 = ct{1507};
t4824 = ct{1508};
t4826 = ct{1509};
t4829 = ct{1510};
t4830 = ct{1511};
t4831 = ct{1512};
t4832 = ct{1513};
t4837 = ct{1514};
t4838 = ct{1515};
t4839 = ct{1516};
t4840 = ct{1517};
t4842 = ct{1518};
t4860 = ct{1519};
t4861 = ct{1520};
t4862 = ct{1521};
t4865 = ct{1522};
t4868 = ct{1523};
t4869 = ct{1524};
t4870 = ct{1525};
t4871 = ct{1526};
t4872 = ct{1527};
t4873 = ct{1528};
t4874 = ct{1529};
t4876 = ct{1530};
t4877 = ct{1531};
t4889 = ct{1532};
t4891 = ct{1533};
t4898 = ct{1534};
t4911 = ct{1535};
t4931 = ct{1536};
t4961 = ct{1537};
t4962 = ct{1538};
t4963 = ct{1539};
t4965 = ct{1540};
t4974 = ct{1541};
t4976 = ct{1542};
t4977 = ct{1543};
t4982 = ct{1544};
t4983 = ct{1545};
t4985 = ct{1546};
t4986 = ct{1547};
t4987 = ct{1548};
t4994 = ct{1549};
t4995 = ct{1550};
t4996 = ct{1551};
t4997 = ct{1552};
t4999 = ct{1553};
t5 = ct{1554};
t50 = ct{1555};
t5001 = ct{1556};
t5002 = ct{1557};
t5005 = ct{1558};
t5007 = ct{1559};
t5010 = ct{1560};
t5011 = ct{1561};
t5013 = ct{1562};
t5014 = ct{1563};
t5015 = ct{1564};
t5017 = ct{1565};
t5018 = ct{1566};
t5020 = ct{1567};
t5021 = ct{1568};
t5023 = ct{1569};
t5024 = ct{1570};
t5026 = ct{1571};
t5028 = ct{1572};
t5030 = ct{1573};
t5031 = ct{1574};
t5032 = ct{1575};
t5033 = ct{1576};
t5035 = ct{1577};
t5036 = ct{1578};
t5037 = ct{1579};
t5038 = ct{1580};
t5039 = ct{1581};
t5040 = ct{1582};
t5041 = ct{1583};
t5042 = ct{1584};
t5044 = ct{1585};
t5045 = ct{1586};
t5046 = ct{1587};
t5047 = ct{1588};
t5048 = ct{1589};
t5049 = ct{1590};
t5058 = ct{1591};
t5061 = ct{1592};
t5063 = ct{1593};
t5064 = ct{1594};
t5069 = ct{1595};
t5090 = ct{1596};
t5092 = ct{1597};
t5094 = ct{1598};
t5096 = ct{1599};
t5115 = ct{1600};
t5118 = ct{1601};
t5121 = ct{1602};
t5123 = ct{1603};
t5124 = ct{1604};
t5126 = ct{1605};
t5127 = ct{1606};
t5128 = ct{1607};
t5130 = ct{1608};
t5131 = ct{1609};
t5144 = ct{1610};
t5145 = ct{1611};
t5146 = ct{1612};
t5147 = ct{1613};
t5148 = ct{1614};
t5152 = ct{1615};
t5153 = ct{1616};
t5159 = ct{1617};
t5160 = ct{1618};
t5163 = ct{1619};
t5164 = ct{1620};
t5165 = ct{1621};
t5167 = ct{1622};
t5168 = ct{1623};
t5169 = ct{1624};
t5189 = ct{1625};
t5191 = ct{1626};
t5195 = ct{1627};
t5198 = ct{1628};
t5201 = ct{1629};
t5202 = ct{1630};
t5203 = ct{1631};
t5205 = ct{1632};
t5206 = ct{1633};
t5207 = ct{1634};
t5219 = ct{1635};
t5221 = ct{1636};
t5222 = ct{1637};
t5223 = ct{1638};
t5224 = ct{1639};
t5225 = ct{1640};
t5226 = ct{1641};
t5227 = ct{1642};
t5228 = ct{1643};
t5229 = ct{1644};
t5230 = ct{1645};
t5231 = ct{1646};
t5232 = ct{1647};
t5233 = ct{1648};
t5234 = ct{1649};
t5235 = ct{1650};
t5236 = ct{1651};
t5237 = ct{1652};
t5238 = ct{1653};
t5239 = ct{1654};
t5240 = ct{1655};
t5241 = ct{1656};
t5242 = ct{1657};
t5243 = ct{1658};
t5244 = ct{1659};
t5245 = ct{1660};
t5246 = ct{1661};
t5247 = ct{1662};
t5248 = ct{1663};
t5249 = ct{1664};
t5252 = ct{1665};
t5254 = ct{1666};
t5255 = ct{1667};
t5257 = ct{1668};
t5260 = ct{1669};
t5265 = ct{1670};
t5266 = ct{1671};
t5295 = ct{1672};
t5301 = ct{1673};
t5302 = ct{1674};
t5306 = ct{1675};
t5308 = ct{1676};
t5316 = ct{1677};
t5317 = ct{1678};
t5320 = ct{1679};
t5328 = ct{1680};
t5337 = ct{1681};
t5338 = ct{1682};
t5339 = ct{1683};
t5340 = ct{1684};
t5342 = ct{1685};
t5344 = ct{1686};
t5345 = ct{1687};
t5346 = ct{1688};
t5347 = ct{1689};
t5348 = ct{1690};
t5349 = ct{1691};
t5350 = ct{1692};
t5361 = ct{1693};
t5362 = ct{1694};
t5377 = ct{1695};
t5379 = ct{1696};
t5380 = ct{1697};
t5381 = ct{1698};
t5383 = ct{1699};
t5384 = ct{1700};
t5388 = ct{1701};
t5389 = ct{1702};
t5391 = ct{1703};
t5392 = ct{1704};
t5393 = ct{1705};
t5395 = ct{1706};
t5399 = ct{1707};
t5402 = ct{1708};
t5403 = ct{1709};
t5405 = ct{1710};
t5407 = ct{1711};
t5411 = ct{1712};
t5427 = ct{1713};
t5428 = ct{1714};
t5431 = ct{1715};
t5433 = ct{1716};
t5434 = ct{1717};
t5440 = ct{1718};
t5441 = ct{1719};
t5443 = ct{1720};
t5444 = ct{1721};
t5458 = ct{1722};
t5461 = ct{1723};
t5462 = ct{1724};
t5465 = ct{1725};
t5480 = ct{1726};
t5481 = ct{1727};
t5482 = ct{1728};
t5483 = ct{1729};
t5484 = ct{1730};
t5485 = ct{1731};
t5486 = ct{1732};
t5487 = ct{1733};
t5488 = ct{1734};
t5489 = ct{1735};
t5490 = ct{1736};
t5491 = ct{1737};
t5492 = ct{1738};
t5493 = ct{1739};
t5494 = ct{1740};
t5496 = ct{1741};
t5498 = ct{1742};
t5499 = ct{1743};
t5500 = ct{1744};
t5504 = ct{1745};
t5505 = ct{1746};
t5509 = ct{1747};
t5510 = ct{1748};
t5514 = ct{1749};
t5515 = ct{1750};
t5516 = ct{1751};
t5517 = ct{1752};
t5518 = ct{1753};
t5522 = ct{1754};
t5523 = ct{1755};
t5524 = ct{1756};
t5531 = ct{1757};
t5535 = ct{1758};
t5550 = ct{1759};
t5552 = ct{1760};
t5553 = ct{1761};
t5554 = ct{1762};
t5556 = ct{1763};
t5557 = ct{1764};
t5578 = ct{1765};
t5580 = ct{1766};
t56 = ct{1767};
t5603 = ct{1768};
t5620 = ct{1769};
t5626 = ct{1770};
t5627 = ct{1771};
t5631 = ct{1772};
t5670 = ct{1773};
t5671 = ct{1774};
t5674 = ct{1775};
t5675 = ct{1776};
t5678 = ct{1777};
t5679 = ct{1778};
t5681 = ct{1779};
t5682 = ct{1780};
t5694 = ct{1781};
t5695 = ct{1782};
t5700 = ct{1783};
t5701 = ct{1784};
t5702 = ct{1785};
t5703 = ct{1786};
t5720 = ct{1787};
t5722 = ct{1788};
t5723 = ct{1789};
t5750 = ct{1790};
t5791 = ct{1791};
t5792 = ct{1792};
t58 = ct{1793};
t5835 = ct{1794};
t5839 = ct{1795};
t5840 = ct{1796};
t5841 = ct{1797};
t5852 = ct{1798};
t5853 = ct{1799};
t5876 = ct{1800};
t5879 = ct{1801};
t5890 = ct{1802};
t5891 = ct{1803};
t59 = ct{1804};
t5930 = ct{1805};
t5932 = ct{1806};
t5941 = ct{1807};
t5951 = ct{1808};
t5953 = ct{1809};
t5954 = ct{1810};
t5977 = ct{1811};
t5994 = ct{1812};
t6 = ct{1813};
t60 = ct{1814};
t6004 = ct{1815};
t6017 = ct{1816};
t6075 = ct{1817};
t6183 = ct{1818};
t6184 = ct{1819};
t6185 = ct{1820};
t6199 = ct{1821};
t6206 = ct{1822};
t6207 = ct{1823};
t6209 = ct{1824};
t6219 = ct{1825};
t6221 = ct{1826};
t6247 = ct{1827};
t6253 = ct{1828};
t628 = ct{1829};
t6317 = ct{1830};
t6339 = ct{1831};
t6341 = ct{1832};
t635 = ct{1833};
t636 = ct{1834};
t6367 = ct{1835};
t638 = ct{1836};
t640 = ct{1837};
t641 = ct{1838};
t642 = ct{1839};
t643 = ct{1840};
t6484 = ct{1841};
t6485 = ct{1842};
t6486 = ct{1843};
t649 = ct{1844};
t6493 = ct{1845};
t6507 = ct{1846};
t6508 = ct{1847};
t6511 = ct{1848};
t6515 = ct{1849};
t654 = ct{1850};
t6543 = ct{1851};
t6544 = ct{1852};
t655 = ct{1853};
t656 = ct{1854};
t657 = ct{1855};
t659 = ct{1856};
t660 = ct{1857};
t663 = ct{1858};
t664 = ct{1859};
t665 = ct{1860};
t6658 = ct{1861};
t6663 = ct{1862};
t667 = ct{1863};
t668 = ct{1864};
t6689 = ct{1865};
t669 = ct{1866};
t6691 = ct{1867};
t6692 = ct{1868};
t67 = ct{1869};
t670 = ct{1870};
t672 = ct{1871};
t673 = ct{1872};
t674 = ct{1873};
t675 = ct{1874};
t676 = ct{1875};
t677 = ct{1876};
t678 = ct{1877};
t679 = ct{1878};
t68 = ct{1879};
t681 = ct{1880};
t6811 = ct{1881};
t6812 = ct{1882};
t6813 = ct{1883};
t682 = ct{1884};
t684 = ct{1885};
t685 = ct{1886};
t686 = ct{1887};
t687 = ct{1888};
t689 = ct{1889};
t6892 = ct{1890};
t6893 = ct{1891};
t691 = ct{1892};
t6916 = ct{1893};
t692 = ct{1894};
t693 = ct{1895};
t694 = ct{1896};
t7 = ct{1897};
t70 = ct{1898};
t7009 = ct{1899};
t702 = ct{1900};
t7032 = ct{1901};
t7041 = ct{1902};
t707 = ct{1903};
t708 = ct{1904};
t71 = ct{1905};
t710 = ct{1906};
t715 = ct{1907};
t716 = ct{1908};
t717 = ct{1909};
t718 = ct{1910};
t7204 = ct{1911};
t721 = ct{1912};
t722 = ct{1913};
t724 = ct{1914};
t725 = ct{1915};
t73 = ct{1916};
t736 = ct{1917};
t738 = ct{1918};
t740 = ct{1919};
t741 = ct{1920};
t749 = ct{1921};
t756 = ct{1922};
t76 = ct{1923};
t762 = ct{1924};
t768 = ct{1925};
t777 = ct{1926};
t792 = ct{1927};
t793 = ct{1928};
t801 = ct{1929};
t802 = ct{1930};
t808 = ct{1931};
t813 = ct{1932};
t819 = ct{1933};
t821 = ct{1934};
t850 = ct{1935};
t855 = ct{1936};
t874 = ct{1937};
t878 = ct{1938};
t89 = ct{1939};
t90 = ct{1940};
t91 = ct{1941};
t92 = ct{1942};
t941 = ct{1943};
t944 = ct{1944};
t948 = ct{1945};
t951 = ct{1946};
t97 = ct{1947};
t4354 = (t3229.*t3942)./1.0e+8;
t4369 = t3229.*t3942.*5.7e-7;
t4370 = t3229.*t3942.*1.02e-6;
t4372 = t3229.*t3942.*2.4e-7;
t4373 = t3229.*t3942.*4.0e-8;
t4402 = -t4400;
t4406 = -t4403;
t4411 = -t4409;
t4443 = t17.*t4438;
t4486 = -t4481;
t4492 = -t4490;
t4497 = t3942.*(t1896-t3232).*(-1.0e-8);
t4498 = (t3942.*(t1896-t3232))./1.0e+8;
t4507 = t3229.*t4222.*9.3e-7;
t4508 = t3229.*t4222.*9.0e-8;
t4509 = t3229.*t4223.*1.02e-6;
t4512 = t3524.*t3942.*5.7e-7;
t4513 = t3229.*t4223.*9.0e-8;
t4515 = t3942.*(t1896-t3232).*(-5.7e-7);
t4518 = t3942.*(t1896-t3232).*(-1.02e-6);
t4520 = t3524.*t3942.*4.0e-8;
t4521 = t3942.*(t1896-t3232).*1.02e-6;
t4524 = t3942.*(t1896-t3232).*(-2.4e-7);
t4525 = t3942.*(t1896-t3232).*(-4.0e-8);
t4530 = t3942.*(t1896-t3232).*2.4e-7;
t4532 = t3942.*(t1896-t3232).*4.0e-8;
t4585 = -t4582;
t4595 = t3688.*t3985;
t4597 = -t4596;
t4609 = -t4608;
t4613 = -t4612;
t4618 = t3788.*t3985;
t4619 = t3789.*t3985;
t4628 = t4222.*(t1896-t3232).*(-9.3e-7);
t4629 = t4222.*(t1896-t3232).*(-9.0e-8);
t4630 = t4223.*(t1896-t3232).*(-1.02e-6);
t4631 = t4223.*(t1896-t3232).*1.02e-6;
t4632 = t4223.*(t1896-t3232).*(-9.0e-8);
t4633 = t4223.*(t1896-t3232).*9.0e-8;
t4670 = t3863.*t3985;
t4706 = t3942.*(t2694-t2701+t3036-t3043).*(-1.0e-8);
t4718 = t3942.*(t2694-t2701+t3036-t3043).*(-5.7e-7);
t4719 = t3942.*(t2694-t2701+t3036-t3043).*(-1.02e-6);
t4720 = t3942.*(t2694-t2701+t3036-t3043).*(-2.4e-7);
t4721 = t3942.*(t2694-t2701+t3036-t3043).*(-4.0e-8);
t4724 = t3942.*(t1959-t3306+t38.*t1022.*(t855-t878).*2.196325630278387e-1).*(-5.7e-7);
t4728 = t3942.*(t1959-t3306+t38.*t1022.*(t855-t878).*2.196325630278387e-1).*5.7e-7;
t4732 = t3942.*(t1959-t3306+t38.*t1022.*(t855-t878).*2.196325630278387e-1).*(-4.0e-8);
t4788 = -t4786;
t4805 = t4781.*1.838876e-2;
t4809 = t4782.*9.99471e-3;
t4818 = t3942.*(t3235-t3535).*(-1.02e-6);
t4843 = t28.*t4824;
t4844 = t34.*t4824;
t4875 = -t4874;
t4880 = t3942.*(t1005+t26.*(t1941-t3308+t39.*t1022.*(t855-t878).*2.196325630278387e-1)).*(-5.7e-7);
t4884 = t3942.*(t1005+t26.*(t1941-t3308+t39.*t1022.*(t855-t878).*2.196325630278387e-1)).*(-4.0e-8);
t4886 = t3271+t3289+t3573+t3574;
t4899 = t4222.*(t2694-t2701+t3036-t3043).*(-9.3e-7);
t4900 = t4222.*(t2694-t2701+t3036-t3043).*(-9.0e-8);
t4901 = t4223.*(t2694-t2701+t3036-t3043).*(-1.02e-6);
t4902 = t4223.*(t2694-t2701+t3036-t3043).*1.02e-6;
t4903 = t4223.*(t2694-t2701+t3036-t3043).*(-9.0e-8);
t4905 = t4223.*(t2694-t2701+t3036-t3043).*9.0e-8;
t4949 = t4222.*(t3235-t3535).*(-9.3e-7);
t4950 = t4222.*(t3235-t3535).*9.3e-7;
t4951 = t4222.*(t3235-t3535).*(-9.0e-8);
t4952 = t4223.*(t3235-t3535).*(-1.02e-6);
t4953 = t4222.*(t3235-t3535).*9.0e-8;
t4954 = t4223.*(t3235-t3535).*(-9.0e-8);
t4967 = -t4245.*(-t2804+t2838+t3109+t23.*(t1456-t2355).*9.3e-7);
t4968 = t4245.*(-t2804+t2838+t3109+t23.*(t1456-t2355).*9.3e-7);
t4969 = -t4246.*(t2813-t2835+t18.*(t1456-t2355).*1.02e-6+t23.*(t1456-t2355).*9.0e-8);
t4973 = t3388+t3401+t3692+t3695;
t4984 = -t4983;
t4990 = t3065+t4024+t4032;
t4991 = t3074+t4039+t4055;
t4992 = t3076+t4041+t4057;
t4998 = -t4997;
t5000 = -t4999;
t5012 = -t5011;
t5022 = -t5018;
t5025 = -t5020;
t5027 = -t5024;
t5051 = -t2388.*(-t3064+t4027+t3229.*(t1861-t3214).*9.840000000000001e-6);
t5076 = -t5069;
t5093 = t641+t663+t664+t678+t1581+t1595+t1596+t1601+t2296+t2324+t2681+t3031+t3282+t3310;
t5149 = -t5148;
t5150 = t58+t59+t5092;
t5151 = t429+t5092;
t5155 = t410+t649+t670+t686+t687+t1577+t1578+t1586+t1600+t2303+t2339+t2689+t3030+t3292+t3305;
t5184 = -t3057.*(-t3080+t4062+t17.*t3229.*(t1861-t3214).*1.02e-6);
t5190 = t3789.*t4824;
t5196 = t3628.*t3901.*t4278.*2.889644e-2;
t5204 = t3617.*t3877.*t4326;
t5208 = -t3524.*(-t3064+t4027+t3229.*(t1861-t3214).*9.840000000000001e-6);
t5212 = -t3531.*(-t3064+t4027+t3229.*(t1861-t3214).*9.840000000000001e-6);
t5250 = t188.*t5205.*8.595599785252598e-1;
t5251 = t1190+t1214+t1219+t1220+t2145+t2146+t2153+t2169+t2742+t2790+t2947+t3078+t3397+t3414;
t5263 = t4088+t4781;
t5264 = t4101+t4782;
t5273 = t3942.*t4865.*5.7e-7;
t5277 = t3942.*t4865.*4.0e-8;
t5288 = t2307.*t5205;
t5289 = t2338.*t5205;
t5290 = t4450+t4452;
t5291 = t4446+t4459;
t5294 = t3248+t3553+t4078+t4079;
t5297 = t4454+t4477;
t5298 = t4456+t4478;
t5299 = t4476+t4482;
t5303 = t322+t330+t5249;
t5304 = t352+t369+t5249;
t5307 = t341+t370+t1196+t1212+t1237+t1238+t2139+t2140+t2159+t2165+t2754+t2814+t2953+t3072+t3405+t3412;
t5318 = t3356+t3649+t4135+t4136;
t5325 = t50.*t202.*(t3244-t3553+t28.*(t3235-t3535).*1.838876e-2+t34.*(t3235-t3535).*9.99471e-3).*(-6.935255936130809e-19);
t5356 = (t3235-t3535).*(-t3080+t4062+t17.*t3229.*(t1861-t3214).*1.02e-6);
t5387 = t3229.*(t4087-t4782).*(-9.3e-7);
t5390 = t3229.*(t4087-t4782).*(-9.0e-8);
t5396 = t3882.*t5090;
t5449 = (t1896-t3232).*(t4087-t4782).*9.3e-7;
t5455 = (t1896-t3232).*(t4087-t4782).*9.0e-8;
t5525 = -t3877.*t4134.*(t3410-t3708+t3714+t26.*t50.*t202.*(t46-t47).*8.687615694748404e-39);
t5536 = -t4326.*(-t56+t60+t649+t670+t686+t687+t1577+t1578+t1586+t1600+t2303+t2339+t2689+t3030+t3292+t3305);
t5537 = t4326.*(-t56+t60+t649+t670+t686+t687+t1577+t1578+t1586+t1600+t2303+t2339+t2689+t3030+t3292+t3305);
t5540 = t3738+t3823+t3824+t3842+t3895;
t5544 = (t4087-t4782).*(t2694-t2701+t3036-t3043).*9.3e-7;
t5547 = (t4087-t4782).*(t2694-t2701+t3036-t3043).*9.0e-8;
t5565 = (t3235-t3535).*(t4087-t4782).*9.3e-7;
t5566 = t3359.*t3901.*(-t56+t60+t649+t670+t686+t687+t1577+t1578+t1586+t1600+t2303+t2339+t2689+t3030+t3292+t3305).*(-2.889644e-2);
t5571 = (t3235-t3535).*(t4087-t4782).*9.0e-8;
t5595 = t3628.*t3901.*t5092.*2.889644e-2;
t5601 = t3628.*(t2694-t2701+t3036-t3043).*(t649+t670+t686+t687+t1577+t1578+t1586+t1600+t2303+t2339+t2689+t3030+t3292+t3305).*2.889644e-2;
t5605 = -t5295.*(-t2804+t2838+t3109+t23.*(t1456-t2355).*9.3e-7);
t5619 = t3628.*(t2694-t2701+t3036-t3043).*(-t56+t60+t649+t670+t686+t687+t1577+t1578+t1586+t1600+t2303+t2339+t2689+t3030+t3292+t3305).*2.889644e-2;
t5639 = t2515+t3077+t3852+t3854+t4046+t4051;
t5640 = t2529+t3075+t3853+t3855+t4045+t4050;
t5645 = t50.*t189.*(t3505.*1.838876e-2-t3570+t3571+t4277+t22.*(t1861-t3214).*(3.0./5.0e+2)+t22.*t23.*(t1861-t3214).*9.99471e-3).*(-9.543032792050485e-17);
t5646 = t50.*t189.*(t3505.*1.838876e-2-t3570+t3571+t4277+t22.*(t1861-t3214).*(3.0./5.0e+2)+t22.*t23.*(t1861-t3214).*9.99471e-3).*9.543032792050485e-17;
t5661 = -t2297.*(t2292+t3283+t3505.*1.838876e-2-t3570+t3571+t3590+t22.*(t1861-t3214).*3.131399999999998e-4+t22.*t23.*(t1861-t3214).*9.99471e-3);
t5662 = -t4278.*(-t321+t332+t1196+t1212+t1237+t1238+t2139+t2140+t2159+t2165+t2754+t2814+t2953+t3072+t3405+t3412);
t5663 = t4278.*(-t321+t332+t1196+t1212+t1237+t1238+t2139+t2140+t2159+t2165+t2754+t2814+t2953+t3072+t3405+t3412);
t5677 = t2363.*(t3318+t3334+t3621-t3637+t28.*(t3235-t3535).*1.838876e-2+t34.*(t3235-t3535).*9.99471e-3).*(-7.26735e-3);
t5683 = t50.*t202.*(t2342-t2423+t3321+t3346+t3563.*1.838876e-2-t3618+t3619+t33.*(t1896-t3232).*(3.0./5.0e+2)+t33.*t34.*(t1896-t3232).*9.99471e-3).*(-6.935255936130809e-19);
t5684 = t50.*t202.*(t2342-t2423+t3321+t3346+t3563.*1.838876e-2-t3618+t3619+t33.*(t1896-t3232).*(3.0./5.0e+2)+t33.*t34.*(t1896-t3232).*9.99471e-3).*6.935255936130809e-19;
et102 = t2363.*(t2368+t3330+t3563.*1.838876e-2-t3618+t3619+t27.*(t1896-t3232).*1.247162e-2+t33.*(t1896-t3232).*3.131399999999998e-4+t33.*t34.*(t1896-t3232).*9.99471e-3);
et103 = -7.26735e-3;
t5699 = et102.*et103;
t5709 = -t3313.*t3877.*(-t321+t332+t1196+t1212+t1237+t1238+t2139+t2140+t2159+t2165+t2754+t2814+t2953+t3072+t3405+t3412);
t5717 = t3617.*t3877.*t5249;
t5718 = t3617.*(t2674-t2676+t3022-t3027).*(t1196+t1212+t1237+t1238+t2139+t2140+t2159+t2165+t2754+t2814+t2953+t3072+t3405+t3412);
t5721 = t3877.*t5431;
t5724 = t4822.*t5090;
t5729 = -t3480.*t3877.*(-t321+t332+t1196+t1212+t1237+t1238+t2139+t2140+t2159+t2165+t2754+t2814+t2953+t3072+t3405+t3412);
t5730 = t3480.*t3877.*(-t321+t332+t1196+t1212+t1237+t1238+t2139+t2140+t2159+t2165+t2754+t2814+t2953+t3072+t3405+t3412);
t5734 = t3617.*(t2674-t2676+t3022-t3027).*(-t321+t332+t1196+t1212+t1237+t1238+t2139+t2140+t2159+t2165+t2754+t2814+t2953+t3072+t3405+t3412);
t5760 = t50.*t189.*t5750.*9.543032792050485e-17;
t5764 = t3566+t3786+t3787+t3858+t3864+t4161;
t5769 = t2297.*t5750;
t5794 = (t1477-t2502).*(t3081-t3086+t4048-t4061+t4067+t17.*t3229.*(t1861-t3214).*4.0e-8);
t5832 = (t2694-t2701+t3036-t3043).*(t3505.*1.838876e-2-t3570+t3571+t22.*(t1861-t3214).*(3.0./5.0e+2)+t22.*t23.*(t1861-t3214).*9.99471e-3).*(t1513+t1879+t2598+t2820+t2834+t3117+t3118).*(-7.26735e-3);
t5834 = t3628.*t5509.*(t2694-t2701+t3036-t3043).*(-2.889644e-2);
et104 = t3563.*1.33637554986e-4+t3693-t3694+t33.*(t1896-t3232).*4.36041e-5;
et105 = t33.*t34.*(t1896-t3232).*7.26350557185e-5;
t5846 = -(et104+et105).*(t2674-t2676+t3022-t3027).*(t1488+t1874+t2519+t2740+t2747+t3096+t3097);
t5856 = -t5249.*(-t56+t60+t649+t670+t686+t687+t1577+t1578+t1586+t1600+t2303+t2339+t2689+t3030+t3292+t3305);
t5857 = t5249.*(-t56+t60+t649+t670+t686+t687+t1577+t1578+t1586+t1600+t2303+t2339+t2689+t3030+t3292+t3305);
t5864 = -(t3349-t3649+t28.*(t3235-t3535).*1.33637554986e-4+t34.*(t3235-t3535).*7.26350557185e-5).*(t2674-t2676+t3022-t3027).*(t1488+t1874+t2519+t2740+t2747+t3096+t3097);
t5866 = t50.*t189.*t5841.*9.543032792050485e-17;
t5869 = -t5092.*(-t321+t332+t1196+t1212+t1237+t1238+t2139+t2140+t2159+t2165+t2754+t2814+t2953+t3072+t3405+t3412);
t5871 = t5092.*(-t321+t332+t1196+t1212+t1237+t1238+t2139+t2140+t2159+t2165+t2754+t2814+t2953+t3072+t3405+t3412);
t5880 = -t5879;
t5900 = t2297.*t5841;
et106 = -t2306-t2317+t3144+t3147+t35.*t941.*t948.*(t850-t874).*3.775747223193135e-1;
et107 = t36.*t941.*t948.*(t850-t874).*2.244797987218524e-1;
t5909 = t3617.*(et106+et107).*(-t321+t332+t1196+t1212+t1237+t1238+t2139+t2140+t2159+t2165+t2754+t2814+t2953+t3072+t3405+t3412);
t5911 = -t3985.*(t3081-t3086+t4048-t4061+t4067+t17.*t3229.*(t1861-t3214).*4.0e-8);
t5943 = t4336+t4337+t4463+t4466;
t5944 = t4338+t4339+t4462+t4465;
t5992 = t2162+t2775+t2803+t2807+t2808+t3998+t4000+t4004+t4206+t4210;
t5995 = t3739+t3740+t4225+t4229+t4317+t4318;
t6018 = t3452+t3461+t4290+t4294+t4360+t4364;
t6020 = (t1477-t2502).*(t4474+t4481-t4484-t4488);
t6026 = t3807+t3825+t3867+t4283+t4300+t4371;
t6041 = t3016+t3068+t4416+t4417+t4451+t4461;
et108 = t3015-t3068+t4415-t4461+t3481.*(t1959-t3306+t38.*t1022.*(t855-t878).*2.196325630278387e-1).*9.840000000000001e-6;
et109 = t3230.*((t237.*(t42-t43))./9.007199254740992e+15+t21.*(-t1881+t3121+t3269)).*9.840000000000001e-6;
t6057 = -t2388.*(et108+et109);
et110 = t3015-t3068+t4415-t4461+t3481.*(t1959-t3306+t38.*t1022.*(t855-t878).*2.196325630278387e-1).*9.840000000000001e-6;
et111 = t3230.*((t237.*(t42-t43))./9.007199254740992e+15+t21.*(-t1881+t3121+t3269)).*9.840000000000001e-6;
t6058 = t2388.*(et110+et111);
et112 = -t2748-t2749+t2773+t2781-t2788+t3204+t3458+t3997-t4009+t262.*(t46-t47).*2.075672598245148e-23;
et113 = t264.*(t46-t47).*1.875105520197095e-20;
t6065 = (et112+et113).*(-t56+t60+t649+t670+t686+t687+t1577+t1578+t1586+t1600+t2303+t2339+t2689+t3030+t3292+t3305);
t6094 = -t5510.*(-t321+t332+t1196+t1212+t1237+t1238+t2139+t2140+t2159+t2165+t2754+t2814+t2953+t3072+t3405+t3412);
t6095 = t5510.*(-t321+t332+t1196+t1212+t1237+t1238+t2139+t2140+t2159+t2165+t2754+t2814+t2953+t3072+t3405+t3412);
t6135 = -t3985.*(t4474+t4481-t4484-t4488);
et114 = t3015-t3068+t4415-t4461+t3481.*(t1959-t3306+t38.*t1022.*(t855-t878).*2.196325630278387e-1).*9.840000000000001e-6;
et115 = t3230.*((t237.*(t42-t43))./9.007199254740992e+15+t21.*(-t1881+t3121+t3269)).*9.840000000000001e-6;
t6151 = -t3524.*(et114+et115);
et116 = t3015-t3068+t4415-t4461+t3481.*(t1959-t3306+t38.*t1022.*(t855-t878).*2.196325630278387e-1).*9.840000000000001e-6;
et117 = t3230.*((t237.*(t42-t43))./9.007199254740992e+15+t21.*(-t1881+t3121+t3269)).*9.840000000000001e-6;
t6153 = -t3531.*(et116+et117);
et118 = t707+t708-t721-t722-t749+t762+t768-t777-t792-t793-t801-t802-t808+t813-t819+t821-t1629+t1637-t1640-t1641-t1659-t1661+t1666+t1667+t1683+t1692+t1705-t1712+t1758+t1759+t1775+t1776+t1973+t1993+t1994+t2023+t2053+t2060-t2089-t2090+t2098+t2099-t14.*t15.*t21.*t50.*t189.*3.670836568391568e-22;
et119 = t16.*t19.*t20.*t50.*t189.*(-3.279367663374749e-19)-t14.*t15.*t17.*t21.*t50.*t189.*7.075931802640439e-19;
et120 = t14.*t17.*t20.*t21.*t50.*t189.*(-1.190170786299927e-18)-t15.*t17.*t19.*t21.*t50.*t189.*1.190170786299927e-18;
et121 = t19.*t20.*t21.*t22.*t50.*t189.*(-3.226512155691387e-19);
t6321 = (t3410-t3708+t3714+t26.*t50.*t202.*(t46-t47).*8.687615694748404e-39).*(et118+et119+et120+et121);
t6323 = t4175.*t5941.*(t2694-t2701+t3036-t3043).*(-1.08769e-2);
t6324 = t4175.*t5941.*(t2694-t2701+t3036-t3043).*1.08769e-2;
t6375 = -t3209.*(-t4196+t4285+t4582+t3206.*(t1896-t3232)+t3985.*(t2801-t2850)+t27.*t3863.*(t1896-t3232));
t6405 = (t1861-t3214).*(-t4196+t4285+t4582+t3206.*(t1896-t3232)+t3985.*(t2801-t2850)+t27.*t3863.*(t1896-t3232));
t6450 = (t2674-t2676+t3022-t3027).*(-t4196+t4285+t4582+t3206.*(t1896-t3232)+t3985.*(t2801-t2850)+t27.*t3863.*(t1896-t3232));
t6516 = t4820+t4821+t5159+t5160;
t6565 = t2735+t2823+t2927+t2941+t3006+t3010+t3970+t4188+t4214+t4215+t4889+t4891;
t6861 = t3901.*t6515.*(t1513+t1879+t2598+t2820+t2834+t3117+t3118).*(-7.26735e-3);
t6862 = t3901.*t6515.*(t1513+t1879+t2598+t2820+t2834+t3117+t3118).*7.26735e-3;
t6980 = t2965+t2966+t3019+t3083+t4327+t4329+t4346+t4352+t4423+t4426+t4471+t4472;
t6981 = t2969+t2970+t3018+t3082+t4328+t4330+t4344+t4351+t4422+t4425+t4469+t4479;
t7029 = t50.*t189.*t7009.*9.543032792050485e-17;
t7039 = t5941.*t6183;
t7043 = t1598+t1703+t2358+t2402+t2413+t2422+t2433+t2434+t2539+t2664+t2985+t2986+t3178+t3383+t3917+t3955+t3971+t4143+t4182+t4183+t4861+t4862;
t7051 = t2297.*t7032;
t7064 = t1612+t2358+t2447+t2450+t2459+t2460+t2508+t2539+t2664+t2985+t2986+t3956+t3960+t3966+t4177+t4182+t4183+t4186+t4861+t4862;
t7217 = t4689+t4697+t4831+t4838+t5036+t5045+t5164+t5168;
t7218 = t4695+t4698+t4830+t4837+t5037+t5046+t5163+t5167;
et122 = t4693-t5037+t5044-t5163+t4865.*(t1861-t3214).*3.24e-6+t3901.*(t951+t16.*(-t1881+t3121+t3269)).*3.24e-6+t4080.*(t2694-t2701+t3036-t3043).*3.24e-6;
et123 = t3901.*(-t1901+t3122+t3270).*3.11e-6;
t7219 = t50.*t202.*(et122+et123).*(-9.543032792050485e-17);
et124 = t4693-t5037+t5044-t5163+t4865.*(t1861-t3214).*3.24e-6+t3901.*(t951+t16.*(-t1881+t3121+t3269)).*3.24e-6+t4080.*(t2694-t2701+t3036-t3043).*3.24e-6;
et125 = t3901.*(-t1901+t3122+t3270).*3.11e-6;
t7220 = t50.*t202.*(et124+et125).*9.543032792050485e-17;
et126 = t4688-t5036+t5042-t5164+t4865.*(t1861-t3214).*7.83e-6+t3901.*(t951+t16.*(-t1881+t3121+t3269)).*7.83e-6+t4080.*(t2694-t2701+t3036-t3043).*7.83e-6;
et127 = t3901.*(-t1901+t3122+t3270).*3.24e-6;
t7221 = -t2363.*(et126+et127);
et128 = t4693-t5037+t5044-t5163+t4865.*(t1861-t3214).*3.24e-6+t3901.*(t951+t16.*(-t1881+t3121+t3269)).*3.24e-6+t4080.*(t2694-t2701+t3036-t3043).*3.24e-6;
et129 = t3901.*(-t1901+t3122+t3270).*3.11e-6;
t7226 = -t3229.*(et128+et129);
et130 = t4693-t5037+t5044-t5163+t4865.*(t1861-t3214).*3.24e-6+t3901.*(t951+t16.*(-t1881+t3121+t3269)).*3.24e-6+t4080.*(t2694-t2701+t3036-t3043).*3.24e-6;
et131 = t3901.*(-t1901+t3122+t3270).*3.11e-6;
t7227 = -t3230.*(et130+et131);
et132 = t4693-t5037+t5044-t5163+t4865.*(t1861-t3214).*3.24e-6+t3901.*(t951+t16.*(-t1881+t3121+t3269)).*3.24e-6+t4080.*(t2694-t2701+t3036-t3043).*3.24e-6;
et133 = t3901.*(-t1901+t3122+t3270).*3.11e-6;
t7228 = t3229.*(et132+et133);
et134 = t4688-t5036+t5042-t5164+t4865.*(t1861-t3214).*7.83e-6+t3901.*(t951+t16.*(-t1881+t3121+t3269)).*7.83e-6+t4080.*(t2694-t2701+t3036-t3043).*7.83e-6;
et135 = t3901.*(-t1901+t3122+t3270).*3.24e-6;
t7229 = (et134+et135).*(t1896-t3232);
et136 = t4688-t5036+t5042-t5164+t4865.*(t1861-t3214).*7.83e-6+t3901.*(t951+t16.*(-t1881+t3121+t3269)).*7.83e-6+t4080.*(t2694-t2701+t3036-t3043).*7.83e-6;
et137 = t3901.*(-t1901+t3122+t3270).*3.24e-6;
t7230 = -t3528.*(et136+et137);
t3509 = -t3501;
t3518 = -t3516;
t3565 = -t3556;
t3569 = -t3568;
t3596 = -t3585;
t3600 = -t3589;
t3609 = t3502.*9.99471e-3;
t3610 = t3501.*1.838876e-2;
t3611 = -t3601;
t3612 = -t3604;
t3614 = -t3608;
t3639 = -t3631;
t3641 = -t3635;
t3646 = -t3642;
t3651 = -t3644;
t3653 = t3557.*9.99471e-3;
t3654 = t3556.*1.838876e-2;
t3663 = -t3661;
t3718 = -t3710;
t3726 = -t3719;
t3728 = -t3723;
t3730 = t3557.*7.26350557185e-5;
t3731 = t3556.*1.33637554986e-4;
t3963 = -t3951;
t3967 = t3220+t3507;
t3996 = t3238+t3554;
t4007 = t3950.*9.99471e-3;
t4008 = t3951.*9.99471e-3;
t4010 = t3950.*1.838876e-2;
t4011 = t3951.*1.838876e-2;
t4021 = t23.*t3946.*9.99471e-3;
t4022 = t18.*t3946.*1.838876e-2;
t4025 = t23.*t3957.*9.99471e-3;
t4026 = t18.*t3957.*1.838876e-2;
t4071 = t3991.*1.838876e-2;
t4072 = t3990.*9.99471e-3;
t4073 = t3991.*9.99471e-3;
t4074 = t3990.*1.838876e-2;
t4083 = t34.*t3992.*9.99471e-3;
t4084 = t28.*t3992.*1.838876e-2;
t4118 = t3990.*1.33637554986e-4;
t4119 = t3991.*1.33637554986e-4;
t4120 = t3990.*7.26350557185e-5;
t4121 = t3991.*7.26350557185e-5;
t4141 = t28.*t3992.*1.33637554986e-4;
t4142 = t34.*t3992.*7.26350557185e-5;
t4224 = t3497+t3502;
t4247 = t3546+t3557;
t4275 = t17.*t2297.*t3992.*1.02e-6;
t4297 = t3063.*t3992;
t4307 = -t4305;
t4311 = t3132.*t3992;
t4313 = -t3992.*(t1953-t2828);
t4357 = (t3229.*t3946)./1.0e+8;
t4359 = (t3230.*t3957)./1.0e+8;
t4374 = t3229.*t3946.*5.7e-7;
t4375 = t3229.*t3946.*1.02e-6;
t4376 = -t4372;
t4377 = -t4373;
t4378 = t3229.*t3946.*2.4e-7;
t4379 = t3229.*t3946.*4.0e-8;
t4381 = t23.*t3229.*t3946.*9.3e-7;
t4382 = t3230.*t3957.*5.7e-7;
t4383 = t3230.*t3957.*1.02e-6;
t4385 = t18.*t3229.*t3946.*9.0e-8;
t4386 = t23.*t3229.*t3946.*9.0e-8;
t4387 = t3230.*t3957.*2.4e-7;
t4388 = t3230.*t3957.*4.0e-8;
t4390 = t23.*t3230.*t3957.*9.3e-7;
t4395 = t18.*t3230.*t3957.*9.0e-8;
t4396 = t23.*t3230.*t3957.*9.0e-8;
t4491 = t3490+t3950;
t4499 = (t3524.*t3946)./1.0e+8;
t4501 = t3946.*(t1896-t3232).*(-1.0e-8);
t4502 = (t3528.*t3957)./1.0e+8;
t4504 = (t3531.*t3957)./1.0e+8;
t4510 = t3541+t3990;
t4511 = -t4509;
t4514 = t3547+t3991;
t4516 = -t4512;
t4517 = -t4513;
t4522 = t3524.*t3946.*1.02e-6;
t4526 = t3946.*(t1896-t3232).*(-5.7e-7);
t4528 = t3946.*(t1896-t3232).*(-1.02e-6);
t4531 = t3524.*t3946.*2.4e-7;
t4533 = t3524.*t3946.*4.0e-8;
t4535 = t3946.*(t1896-t3232).*(-2.4e-7);
t4536 = t3946.*(t1896-t3232).*(-4.0e-8);
t4539 = t23.*t3946.*(t1896-t3232).*(-9.3e-7);
t4542 = t3528.*t3957.*5.7e-7;
t4543 = t3528.*t3957.*1.02e-6;
t4545 = t18.*t3946.*(t1896-t3232).*(-9.0e-8);
t4546 = t23.*t3946.*(t1896-t3232).*(-9.0e-8);
t4549 = t3531.*t3957.*1.02e-6;
t4550 = t27.*t3946.*(t1896-t3232).*1.02e-6;
t4551 = t3528.*t3957.*2.4e-7;
t4552 = t3528.*t3957.*4.0e-8;
t4555 = t23.*t3528.*t3957.*9.3e-7;
t4560 = t3531.*t3957.*2.4e-7;
t4562 = t3531.*t3957.*4.0e-8;
t4563 = t18.*t3528.*t3957.*(-1.02e-6);
t4571 = t18.*t3528.*t3957.*9.0e-8;
t4572 = t23.*t3528.*t3957.*9.0e-8;
t4584 = -t3992.*(t335-t1539-t2831+t2851);
t4586 = t17.*t3483.*t3992.*1.02e-6;
t4622 = -t4618;
t4623 = t3789.*t3992;
t4627 = t3793.*t3992;
t4651 = t2310+t3294+t3594+t3602;
t4657 = t3843.*t3992;
t4672 = t3863.*t3992;
t4708 = t3946.*(t2694-t2701+t3036-t3043).*(-1.0e-8);
t4709 = t3946.*(t1959-t3306+t38.*t1022.*(t855-t878).*2.196325630278387e-1).*(-1.0e-8);
t4710 = (t3901.*t3957)./1.0e+8;
t4711 = (t3904.*t3957)./1.0e+8;
t4717 = t2769+t3413+t3708+t3722;
t4722 = t3946.*(t2694-t2701+t3036-t3043).*(-5.7e-7);
t4723 = t3946.*(t2694-t2701+t3036-t3043).*(-1.02e-6);
t4725 = t3946.*(t2694-t2701+t3036-t3043).*5.7e-7;
t4726 = t3946.*(t2694-t2701+t3036-t3043).*1.02e-6;
t4727 = t3946.*(t2694-t2701+t3036-t3043).*(-2.4e-7);
t4729 = t3946.*(t2694-t2701+t3036-t3043).*(-4.0e-8);
t4731 = t23.*t3946.*(t2694-t2701+t3036-t3043).*(-9.3e-7);
t4733 = t3901.*t3957.*5.7e-7;
t4734 = t3901.*t3957.*1.02e-6;
t4735 = t3946.*(t1959-t3306+t38.*t1022.*(t855-t878).*2.196325630278387e-1).*(-1.02e-6);
t4736 = t3904.*t3957.*1.02e-6;
t4737 = t3946.*(t2694-t2701+t3036-t3043).*4.0e-8;
t4738 = t3946.*(t1959-t3306+t38.*t1022.*(t855-t878).*2.196325630278387e-1).*(-2.4e-7);
t4740 = t23.*t3946.*(t2694-t2701+t3036-t3043).*9.3e-7;
t4741 = t3901.*t3957.*2.4e-7;
t4744 = t3901.*t3957.*4.0e-8;
t4745 = t18.*t3946.*(t2694-t2701+t3036-t3043).*(-9.0e-8);
t4746 = t3904.*t3957.*2.4e-7;
t4747 = t23.*t3946.*(t2694-t2701+t3036-t3043).*(-9.0e-8);
t4749 = t23.*t3901.*t3957.*9.3e-7;
t4750 = t3946.*(t1959-t3306+t38.*t1022.*(t855-t878).*2.196325630278387e-1).*(-4.0e-8);
t4756 = t18.*t3946.*(t2694-t2701+t3036-t3043).*9.0e-8;
t4759 = t23.*t3946.*(t2694-t2701+t3036-t3043).*9.0e-8;
t4760 = t3946.*(t1959-t3306+t38.*t1022.*(t855-t878).*2.196325630278387e-1).*4.0e-8;
t4762 = t3904.*t3957.*4.0e-8;
t4768 = t18.*t3901.*t3957.*9.0e-8;
t4769 = t23.*t3901.*t3957.*9.0e-8;
t4797 = t3229.*(t3951+t18.*(t1861-t3214)).*(-9.3e-7);
t4798 = t3229.*(t3951+t18.*(t1861-t3214)).*(-1.02e-6);
t4799 = t3229.*(t3951+t18.*(t1861-t3214)).*9.3e-7;
t4800 = t3229.*(t3951+t18.*(t1861-t3214)).*(-9.0e-8);
t4801 = t3229.*(t3951+t18.*(t1861-t3214)).*9.0e-8;
t4819 = t3946.*t3985.*1.02e-6;
t4828 = t3946.*(t3235-t3535).*(-1.02e-6);
t4833 = t3946.*(t3235-t3535).*1.02e-6;
t4836 = t23.*t3946.*(t3235-t3535).*(-9.3e-7);
t4845 = t23.*t3946.*(t3235-t3535).*(-9.0e-8);
t4846 = t3957.*t3992.*1.02e-6;
t4847 = t18.*t3946.*(t3235-t3535).*(-9.0e-8);
t4849 = t23.*t3957.*t3992.*9.3e-7;
t4852 = t18.*t3957.*t3992.*(-1.02e-6);
t4856 = t23.*t3957.*t3992.*9.0e-8;
t4857 = t18.*t3957.*t3992.*9.0e-8;
t4863 = t4844.*9.99471e-3;
t4864 = t4843.*1.838876e-2;
t4866 = t3946.*(t1005+t26.*(t1941-t3308+t39.*t1022.*(t855-t878).*2.196325630278387e-1)).*(-1.0e-8);
t4867 = (t3957.*t4113)./1.0e+8;
t4878 = -t28.*t3992.*(t2813-t2835+t18.*(t1456-t2355).*1.02e-6+t23.*(t1456-t2355).*9.0e-8);
t4879 = -t34.*t3992.*(-t2804+t2838+t3109+t23.*(t1456-t2355).*9.3e-7);
t4881 = t3946.*(t1005+t26.*(t1941-t3308+t39.*t1022.*(t855-t878).*2.196325630278387e-1)).*(-1.02e-6);
t4882 = t28.*t3992.*(t2813-t2835+t18.*(t1456-t2355).*1.02e-6+t23.*(t1456-t2355).*9.0e-8);
t4883 = t34.*t3992.*(-t2804+t2838+t3109+t23.*(t1456-t2355).*9.3e-7);
t4885 = t3946.*(t1005+t26.*(t1941-t3308+t39.*t1022.*(t855-t878).*2.196325630278387e-1)).*(-2.4e-7);
t4887 = t3946.*(t1005+t26.*(t1941-t3308+t39.*t1022.*(t855-t878).*2.196325630278387e-1)).*(-4.0e-8);
t4888 = t3957.*t4113.*1.02e-6;
t4890 = t3957.*t4113.*2.4e-7;
t4892 = t4844.*7.26350557185e-5;
t4893 = t3957.*t4113.*4.0e-8;
t4894 = t4843.*1.33637554986e-4;
t4897 = t3286+t3288+t3604+t3606;
t4917 = t3524.*(t3951+t18.*(t1861-t3214)).*(-9.3e-7);
t4921 = (t3951+t18.*(t1861-t3214)).*(t1896-t3232).*9.3e-7;
t4922 = (t3951+t18.*(t1861-t3214)).*(t1896-t3232).*1.02e-6;
t4925 = t3524.*(t3951+t18.*(t1861-t3214)).*(-9.0e-8);
t4927 = (t3951+t18.*(t1861-t3214)).*(t1896-t3232).*9.0e-8;
t4975 = t3400+t3404+t3717+t3721;
t4989 = t3064+t4023+t4031;
t4993 = t3080+t4049+t4064;
t5034 = t50.*t202.*t4991.*9.543032792050485e-17;
t5052 = t2363.*t4990;
t5053 = t2388.*t4990;
t5054 = t2399.*t4990;
t5056 = t2363.*t4992;
t5067 = (t3951+t18.*(t1861-t3214)).*(t2694-t2701+t3036-t3043).*9.3e-7;
t5068 = (t3951+t18.*(t1861-t3214)).*(t2694-t2701+t3036-t3043).*1.02e-6;
t5073 = (t3951+t18.*(t1861-t3214)).*(t1959-t3306+t38.*t1022.*(t855-t878).*2.196325630278387e-1).*9.3e-7;
t5074 = (t3951+t18.*(t1861-t3214)).*(t2694-t2701+t3036-t3043).*9.0e-8;
t5077 = (t3951+t18.*(t1861-t3214)).*(t1959-t3306+t38.*t1022.*(t855-t878).*2.196325630278387e-1).*9.0e-8;
t5091 = t3836+t3839+t3897;
t5105 = t3985.*(t3951+t18.*(t1861-t3214)).*(-9.3e-7);
t5108 = t3985.*(t3951+t18.*(t1861-t3214)).*9.3e-7;
t5111 = t3985.*(t3951+t18.*(t1861-t3214)).*(-9.0e-8);
t5113 = (t3951+t18.*(t1861-t3214)).*(t3235-t3535).*9.3e-7;
t5114 = (t3951+t18.*(t1861-t3214)).*(t3235-t3535).*1.02e-6;
t5116 = t3985.*(t3951+t18.*(t1861-t3214)).*9.0e-8;
t5119 = (t3951+t18.*(t1861-t3214)).*(t3235-t3535).*9.0e-8;
t5154 = t56+t73+t5093;
t5158 = (t1005+t26.*(t1941-t3308+t39.*t1022.*(t855-t878).*2.196325630278387e-1)).*(t3951+t18.*(t1861-t3214)).*9.3e-7;
t5162 = (t1005+t26.*(t1941-t3308+t39.*t1022.*(t855-t878).*2.196325630278387e-1)).*(t3951+t18.*(t1861-t3214)).*9.0e-8;
t5192 = t3229.*t4991;
t5193 = t3230.*t4991;
t5209 = t3524.*t4990;
t5210 = -t4990.*(t1896-t3232);
t5211 = t3528.*t4990;
t5213 = t3531.*t4990;
t5214 = t4990.*(t1896-t3232);
t5216 = -t4992.*(t1896-t3232);
t5217 = t3528.*t4992;
t5218 = t3511+t3570+t3580+t3595+t3598;
t5259 = t3992.*(t17.*((t237.*(t42-t43))./9.007199254740992e+15+t21.*(-t1881+t3121+t3269))+t22.*(-t1901+t3122+t3270)).*(-1.02e-6);
t5261 = t3992.*(t17.*((t237.*(t42-t43))./9.007199254740992e+15+t21.*(-t1881+t3121+t3269))+t22.*(-t1901+t3122+t3270)).*1.02e-6;
t5267 = t3957.*t4814.*1.02e-6;
t5269 = t3946.*(t4127+t33.*(t1959-t3306+t38.*t1022.*(t855-t878).*2.196325630278387e-1)).*(-1.02e-6);
t5270 = (t3957.*t4860)./1.0e+8;
t5272 = (t3946.*t4865)./1.0e+8;
t5274 = t3957.*t4860.*1.02e-6;
t5275 = t3946.*t4865.*1.02e-6;
t5276 = t3957.*t4860.*2.4e-7;
t5281 = t3946.*t4865.*2.4e-7;
t5282 = t3957.*t4860.*4.0e-8;
t5285 = t3946.*t4865.*4.0e-8;
t5293 = t4131+t4844;
t5296 = t4140+t4843;
t5305 = t321+t343+t5251;
t5313 = t3655+t3694+t3701+t3725+t3727;
t5322 = t50.*t202.*t5297.*9.543032792050485e-17;
t5330 = t2363.*t5291;
t5331 = t2388.*t5290;
t5332 = t2399.*t5291;
t5335 = t2363.*t5298;
t5357 = -t3992.*(-t3080+t4062+t17.*t3229.*(t1861-t3214).*1.02e-6);
t5358 = t3992.*(-t3080+t4062+t17.*t3229.*(t1861-t3214).*1.02e-6);
t5365 = t3057.*t5299;
t5369 = t4990.*(t3908-(t262.*(t46-t47))./9.007199254740992e+15);
t5370 = t4111.*t4990;
t5385 = t3229.*t5263.*1.02e-6;
t5386 = t3229.*t5263.*9.0e-8;
t5408 = t3229.*t5297;
t5409 = t3230.*t5297;
t5412 = t635+t636+t679+t689+t1587+t1606+t1608+t1609+t2295+t3272+t3278+t3290+t3575+t3582;
t5418 = (t4127+t33.*(t1959-t3306+t38.*t1022.*(t855-t878).*2.196325630278387e-1)).*(t3951+t18.*(t1861-t3214)).*9.3e-7;
t5420 = (t4127+t33.*(t1959-t3306+t38.*t1022.*(t855-t878).*2.196325630278387e-1)).*(t3951+t18.*(t1861-t3214)).*9.0e-8;
t5445 = t5263.*(t1896-t3232).*(-1.02e-6);
t5446 = t5263.*(t1896-t3232).*1.02e-6;
